simulink model "ASM_Traffic_V2X_Complete_Model_2"  (R2019a)
settings: Solver=ode1  StartTime=SIM.tstart.v  StopTime=Inf  FixedStep=SIM.StepSize.v  RelTol=1e-3
PostLoadFcn:
  | if any(exist('dsrtsu_mdlpostloadfcn', 'file') ~= 0), dsrtsu_mdlpostloadfcn('Execute', bdroot); end
  | try, asm_mdl_postloadfcn(bdroot, 'UpdateModel', 2200); catch, disp(lasterr); end,
undefined symbols (not defined in the file): _SensorPnts_1, _SensorPnts_13, _SensorPnts_17, _SensorPnts_21, _SensorPnts_25, _SensorPnts_29, _SensorPnts_33, _SensorPnts_37, _SensorPnts_41, _SensorPnts_45, _SensorPnts_49, _SensorPnts_5, _SensorPnts_53, _SensorPnts_57, _SensorPnts_9, _to_, CPT, G5A, ITS, MDL, rad, s_to_rpm, SIM
libraries: simulink x169, ASM_VehicleDynamics_lib x126, ASM_Traffic_lib x83, ASM_Utils_lib x49, mdbs x45, ASM_Environment_lib x17, dspindex x12, dsaV2xLibraryAux x10, dsmpblib x6, dsaV2xAsn1Library x4, dsaV2xLibrary x4, ASM_BrakeHydraulics_lib x4
(part 7 of 36)

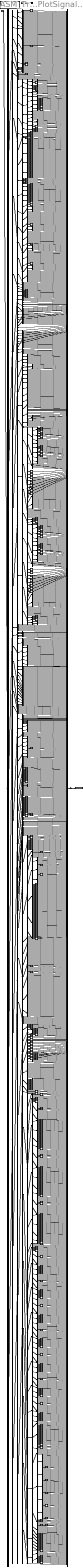
== system ASM_Traffic_V2X_Complete_Model_2/MDLUserInterface/ModelDesk_Plotting/ModelDesk_PlotSignalCollector ==
  ASMSignalBus : Inport
  Accelerations : BusSelector  OutputSignals=VehicleCoG,Wheels
  ActiveBrakeCylinder : BusSelector  OutputSignals=p[bar],p_max[bar],Enable_p_Brake_Desired[0|1],p_Brake_Desired[bar]
  ActiveLateralController : BusSelector  OutputSignals=s_Preview_LatCtrl[m],Angle_SteeringWheel_LatCtrl[deg],e_Lat[m]
  ActiveTire : BusSelector  OutputSignals=v_Circumf_Dyn_FL_Wheel[km|h],Slip_x_FL[],Slip_y_FL[],r_Dyn_FL_Tire[m],CorneringStiffness_FL[N],Coef_RollingRes_FL[],Trq_x_FL_CoorSys_CP[Nm],Trq_y_FL_CoorSys_W[Nm],Trq_z_FL_CoorSys_CP[Nm],F_x_Dyn_FL_Tire_CoorSys_CP[N],F_y_Dyn_FL_Tire_CoorSys_CP[N],F_z_Dyn_FL_Tire_CoorSys_CP[N]
  ActiveTire1 : BusSelector  OutputSignals=v_Circumf_Dyn_FR_Wheel[km|h],Slip_x_FR[],Slip_y_FR[],r_Dyn_FR_Tire[m],CorneringStiffness_FR[N],Coef_RollingRes_FR[],Trq_x_FR_CoorSys_CP[Nm],Trq_y_FR_CoorSys_W[Nm],Trq_z_FR_CoorSys_CP[Nm],F_x_Dyn_FR_Tire_CoorSys_CP[N],F_y_Dyn_FR_Tire_CoorSys_CP[N],F_z_Dyn_FR_Tire_CoorSys_CP[N]
  ActiveTire2 : BusSelector  OutputSignals=v_Circumf_Dyn_RL_Wheel[km|h],Slip_x_RL[],Slip_y_RL[],r_Dyn_RL_Tire[m],CorneringStiffness_RL[N],Coef_RollingRes_RL[],Trq_x_RL_CoorSys_CP[Nm],Trq_y_RL_CoorSys_W[Nm],Trq_z_RL_CoorSys_CP[Nm],F_x_Dyn_RL_Tire_CoorSys_CP[N],F_y_Dyn_RL_Tire_CoorSys_CP[N],F_z_Dyn_RL_Tire_CoorSys_CP[N]
  ActiveTire3 : BusSelector  OutputSignals=v_Circumf_Dyn_RR_Wheel[km|h],Slip_x_RR[],Slip_y_RR[],r_Dyn_RR_Tire[m],CorneringStiffness_RR[N],Coef_RollingRes_RR[],Trq_x_RR_CoorSys_CP[Nm],Trq_y_RR_CoorSys_W[Nm],Trq_z_RR_CoorSys_CP[Nm],F_x_Dyn_RR_Tire_CoorSys_CP[N],F_y_Dyn_RR_Tire_CoorSys_CP[N],F_z_Dyn_RR_Tire_CoorSys_CP[N]
  ActiveTransmission : BusSelector  OutputSignals=Gear[],omega_In_Trm[rad|s],omega_Out_Trm[rad|s],Trq_Out_Trm[Nm],i_Trm[],Inertia_Trm[kgm2],i_unsync_Trm[]
  Aerodynamics : BusSelector  OutputSignals=Forces,Torques,Coefficients
  Ambient : BusSelector  OutputSignals=T_Ambient[degC],p_Ambient[Pa]
  Angle_FL_Wheel[Alpha;Beta;Gamma][deg] : BusSelector  OutputSignals=Angle_Alpha_FL_Wheel[deg],Angle_Beta_FL_Wheel[deg],Angle_Gamma_FL_Wheel[deg]
  Angle_FL_Wheel[Toe;Camber][deg] : BusSelector  OutputSignals=Angle_Toe_FL_Wheel_CoorSys_V[deg],Angle_Camber_FL_Wheel_CoorSys_V[deg]
  Angle_FR_Wheel[Alpha;Beta;Gamma][deg] : BusSelector  OutputSignals=Angle_Alpha_FR_Wheel[deg],Angle_Beta_FR_Wheel[deg],Angle_Gamma_FR_Wheel[deg]
  Angle_FR_Wheel[Toe;Camber][deg] : BusSelector  OutputSignals=Angle_Toe_FR_Wheel_CoorSys_V[deg],Angle_Camber_FR_Wheel_CoorSys_V[deg]
  Angle_Fellows[x;y;z][deg] : BusSelector  OutputSignals=Angle_Roll_Fellows[deg],Angle_Pitch_Fellows[deg],Angle_Yaw_Fellows[deg],Angle_Wheel_Fellows[deg]
  Angle_RL_Wheel[Alpha;Beta;Gamma][deg] : BusSelector  OutputSignals=Angle_Alpha_RL_Wheel[deg],Angle_Beta_RL_Wheel[deg],Angle_Gamma_RL_Wheel[deg]
  Angle_RL_Wheel[Toe;Camber][deg] : BusSelector  OutputSignals=Angle_Toe_RL_Wheel_CoorSys_V[deg],Angle_Camber_RL_Wheel_CoorSys_V[deg]
  Angle_RR_Wheel[Alpha;Beta;Gamma][deg] : BusSelector  OutputSignals=Angle_Alpha_RR_Wheel[deg],Angle_Beta_RR_Wheel[deg],Angle_Gamma_RR_Wheel[deg]
  Angle_RR_Wheel[Toe;Camber][deg] : BusSelector  OutputSignals=Angle_Toe_RR_Wheel_CoorSys_V[deg],Angle_Camber_RR_Wheel_CoorSys_V[deg]
  Angle_Vehicle_CoorSys_E[x;y;z][deg] : BusSelector  OutputSignals=Angle_Roll_Vehicle_CoorSys_E[deg],Angle_Pitch_Vehicle_CoorSys_E[deg],Angle_Yaw_Vehicle_CoorSys_E[deg]
  Angle_Vehicle_Init_CoorSys_E[x;y;z][rad] : BusSelector  OutputSignals=Angle_Roll_Vehicle_Init[rad],Angle_Pitch_Vehicle_Init[rad],Angle_Yaw_Vehicle_Init[rad]
  Angle_Wheel[FL;FR][Toe;Camber][deg] : BusSelector  OutputSignals=Angle_FL_Wheel[Toe;Camber][deg],Angle_FR_Wheel[Toe;Camber][deg]
  Angle_Wheel[RL;RR][Toe;Camber][deg] : BusSelector  OutputSignals=Angle_RL_Wheel[Toe;Camber][deg],Angle_RR_Wheel[Toe;Camber][deg]
  Angular : BusSelector  OutputSignals=w_Vehicle_CoG_dt[x;y;z][rad|s2]
  Angular1 : BusSelector  OutputSignals=w_Vehicle_CoG[x;y;z][deg|s]
  Angular2 : BusSelector  OutputSignals=WheelBodyAngularVelocity,WheelAngularVelocity
  Angular3 : BusSelector  OutputSignals=Angle_Vehicle_CoorSys_E[x;y;z][deg],RotationMatrix_V_to_E[3x3]
  AutomaticTransmission : BusSelector  OutputSignals=LockUpClutch,GearBox,TorqueConverter
  AutomaticTrmCtrlSignals : BusSelector  OutputSignals=SelectorLever[-3T|-2P|-1R|0N|1D],SW_TipTronic[-1Down|0Off|1Up]
  BasicEngine : BusSelector  OutputSignals=EngineTorques,FuelConsumption
  BellValve : BusSelector  OutputSignals=ValveState[1ChamberCon|2AmbientCon|3CloseAll],p_In_BellValve[bar],p_Out_BellValve[bar],T_In_BellValve[degC],m_dot_BellValve[Kg|s],Ctrl_BellValve[0_1]
  Brake : BusSelector  OutputSignals=MasterBrakeCylinder,BrakeHydraulics,BrakeDisc,BrakeBooster,Manifold
  BrakeBooster : BusSelector  OutputSignals=ManifoldValve,VacuumChamber,BellValve,RearChamber,PushRod,ControllerBellValve
  BrakeCylinderLinear : BusSelector  OutputSignals=p[bar],p_max[bar]
  BrakeCylinderPhysical : BusSelector  OutputSignals=Displ_Piston[mm],F[N],p[bar],p_max[bar]
  BrakeDisc : BusSelector  OutputSignals=Torque,MaximumTorque,Pressure,Const_BrakeDiscFactor
  BrakeHydraulics : BusSelector  OutputSignals=BrakingCircuit,BrakeHydraulicsModel[]
  BrakingCircuit : BusSelector  OutputSignals=Pressure
  BusSelector_1 : BusSelector  OutputSignals=SoftECU,VehicleDynamics,BasicEngine,Drivetrain,Environment
  CO2_Emission : BusSelector  OutputSignals=CO2_Emission[kg|h],CO2_Emission_Total[kg]
  CentralDifferential : BusSelector  OutputSignals=omega_Out_Front_CentralDiff[rad|s],omega_Out_Rear_CentralDiff[rad|s],omega_In_CentralDiff[rad|s],Trq_Lock[Nm],omega_Cage[rad|s],Const_i_MainReductionGear[],Const_TrqDistribution[]
  Clutch : BusSelector  OutputSignals=Trq_Fric_Clutch[Nm],Trq_TorsionSpring_Clutch[Nm],omega_Out_ClutchPlate[rad|s]
  Clutch_4WD : BusSelector  OutputSignals=Trq_Lock_Clutch_4WD[Nm],omega_Clutch_4WD_In[rad|s],omega_Clutch_4WD_Out[rad|s]
  Coefficients : BusSelector  OutputSignals=Cw_x[]
  Collision_Sensor : BusSelector  OutputSignals=Collision_Sensor_1
  Collision_Sensor_1 : BusSelector  OutputSignals=Info,SensorOutput
  Common : BusSelector  OutputSignals=LaneID_PrefLane[],LaneID_Absolute[],LaneDirection_Absolute[],LaneDirection_Relative[],LaneWidth[m],LaneCurvature[1|m],Curvature[1|m]
  ComplianceAligningTorque : BusSelector  OutputSignals=Displ_x_Wheel_Trq_z_Left[mm],Displ_x_Wheel_Trq_z_Right[mm],Displ_y_Wheel_Trq_z_Left[mm],Displ_y_Wheel_Trq_z_Right[mm],Angle_Alpha_Wheel_Trq_z_Left[deg],Angle_Alpha_Wheel_Trq_z_Right[deg],Angle_Gamma_Wheel_Trq_z_Left[deg],Angle_Gamma_Wheel_Trq_z_Right[deg]
  ComplianceAligningTorque1 : BusSelector  OutputSignals=Displ_x_Wheel_Trq_z_Left[mm],Displ_x_Wheel_Trq_z_Right[mm],Displ_y_Wheel_Trq_z_Left[mm],Displ_y_Wheel_Trq_z_Right[mm],Angle_Alpha_Wheel_Trq_z_Left[deg],Angle_Alpha_Wheel_Trq_z_Right[deg],Angle_Gamma_Wheel_Trq_z_Left[deg],Angle_Gamma_Wheel_Trq_z_Right[deg]
  ComplianceLatForce : BusSelector  OutputSignals=Displ_x_Wheel_F_y_Left[mm],Displ_x_Wheel_F_y_Right[mm],Displ_y_Wheel_F_y_Left[mm],Displ_y_Wheel_F_y_Right[mm],Angle_Alpha_Wheel_F_y_Left[deg],Angle_Alpha_Wheel_F_y_Right[deg],Angle_Gamma_Wheel_F_y_Left[deg],Angle_Gamma_Wheel_F_y_Right[deg]
  ComplianceLatForce1 : BusSelector  OutputSignals=Displ_x_Wheel_F_y_Left[mm],Displ_x_Wheel_F_y_Right[mm],Displ_y_Wheel_F_y_Left[mm],Displ_y_Wheel_F_y_Right[mm],Angle_Alpha_Wheel_F_y_Left[deg],Angle_Alpha_Wheel_F_y_Right[deg],Angle_Gamma_Wheel_F_y_Left[deg],Angle_Gamma_Wheel_F_y_Right[deg]
  ComplianceLongForce : BusSelector  OutputSignals=Displ_x_Wheel_F_x_Left[mm],Displ_x_Wheel_F_x_Right[mm],Displ_y_Wheel_F_x_Left[mm],Displ_y_Wheel_F_x_Right[mm],Angle_Alpha_Wheel_F_x_Left[deg],Angle_Alpha_Wheel_F_x_Right[deg],Angle_Gamma_Wheel_F_x_Left[deg],Angle_Gamma_Wheel_F_x_Right[deg]
  ComplianceLongForce1 : BusSelector  OutputSignals=Displ_x_Wheel_F_x_Left[mm],Displ_x_Wheel_F_x_Right[mm],Displ_y_Wheel_F_x_Left[mm],Displ_y_Wheel_F_x_Right[mm],Angle_Alpha_Wheel_F_x_Left[deg],Angle_Alpha_Wheel_F_x_Right[deg],Angle_Gamma_Wheel_F_x_Left[deg],Angle_Gamma_Wheel_F_x_Right[deg]
  ComplianceLongTorque : BusSelector  OutputSignals=Displ_x_Wheel_Trq_x_Left[mm],Displ_x_Wheel_Trq_x_Right[mm],Displ_y_Wheel_Trq_x_Left[mm],Displ_y_Wheel_Trq_x_Right[mm],Angle_Alpha_Wheel_Trq_x_Left[deg],Angle_Alpha_Wheel_Trq_x_Right[deg],Angle_Gamma_Wheel_Trq_x_Left[deg],Angle_Gamma_Wheel_Trq_x_Right[deg]
  ComplianceLongTorque1 : BusSelector  OutputSignals=Displ_x_Wheel_Trq_x_Left[mm],Displ_x_Wheel_Trq_x_Right[mm],Displ_y_Wheel_Trq_x_Left[mm],Displ_y_Wheel_Trq_x_Right[mm],Angle_Alpha_Wheel_Trq_x_Left[deg],Angle_Alpha_Wheel_Trq_x_Right[deg],Angle_Gamma_Wheel_Trq_x_Left[deg],Angle_Gamma_Wheel_Trq_x_Right[deg]
  Const_BrakeDiscFactor : BusSelector  OutputSignals=Const_BrakeDiscFactor_FL[m3],Const_BrakeDiscFactor_FR[m3],Const_BrakeDiscFactor_RL[m3],Const_BrakeDiscFactor_RR[m3]
  ContactPoint : BusSelector  OutputSignals=r_FL_Tire[m],Pos_CP_FL_CoorSys_E[x;y][m]
  ContactPoint1 : BusSelector  OutputSignals=r_FR_Tire[m],Pos_CP_FR_CoorSys_E[x;y][m]
  ContactPoint2 : BusSelector  OutputSignals=r_RL_Tire[m],Pos_CP_RL_CoorSys_E[x;y][m]
  ContactPoint3 : BusSelector  OutputSignals=r_RR_Tire[m],Pos_CP_RR_CoorSys_E[x;y][m]
  ContentID : Constant  Value=81472368640
  ControllerBellValve : BusSelector  OutputSignals=p_Setpoint[bar],p_MasterBrakeCyl[bar],p_delta[bar],ValveState[1ChamberCon|2AmbientCon],Ctrl_A_BellValve[0_1],F_Pedal[N]
  Controller_ACC : BusSelector  OutputSignals=State_ACC[0Off|1On],Sw_ACC_Distance[s],Control_Mode_ACC[0Off|1CC|2DC],v_Set_CC[km|h],v_Set_DC[km|h],v_Set[km|h],a_x_Set[m|s2],a_x_UpperLimit[m|s2],a_x_LowerLimit[m|s2],a_x_RisingRateMax[m|s3],a_x_FallingRateMax[m|s3]s,Distance_Set[m],Dist_Ref_Vehicle[m],FCW[0Off|1On],AEB[0Off|1On],TTC[s],Collision[0Off|1On],Sw_BrakeMode[1Comfort|2AEBOnly|3AEBOff],Enable_Trq_Brake_ACC[0|1],Enable_Trq_Engine_ACC[0|1]
  Crankshaft : BusSelector  OutputSignals=n_Engine[rad|s],n_Engine[rpm],Trq_Mass_Mod[Nm],Const_Inertia_Engine[kgm2],Trq_Eff_Crank[Nm]
  CurrentLane : BusSelector  OutputSignals=Common,LeftSide,RightSide
  CustomPoints : BusSelector  OutputSignals=ID[],Object_ID[],Dist_CoorSys_S[m],Angle_Hor_CoorSys_S[deg],Pos_CoorSys_E[x;y;z][m]
  CustomPoints1 : BusSelector  OutputSignals=ID[],Object_ID[],Dist_CoorSys_S[m],Angle_Hor_CoorSys_S[deg],Pos_CoorSys_E[x;y;z][m]
  CustomPoints2 : BusSelector  OutputSignals=ID[],Object_ID[],Dist_CoorSys_S[m],Angle_Hor_CoorSys_S[deg],Pos_CoorSys_E[x;y;z][m]
  Custom_Sensor : BusSelector  OutputSignals=Sensor_Front_1
  Damper_Left : BusSelector  OutputSignals=Displ_Damper_FL_dt[m|s],Displ_Damper_FL_dq1_Front[],Displ_Damper_FL_dq2_Front[],Displ_Damper_FL[m]
  Damper_Left1 : BusSelector  OutputSignals=Displ_Damper_RL_dt[m|s],Displ_Damper_RL_dq1_Rear,Displ_Damper_RL_dq2_Rear,Displ_Damper_RL[m]
  Damper_Right : BusSelector  OutputSignals=Displ_Damper_FR_dt[m|s],Displ_Damper_FR_dq1_Front[],Displ_Damper_FR_dq2_Front[],Displ_Damper_FR[m]
  Damper_Right1 : BusSelector  OutputSignals=Displ_Damper_RR_dt[m|s],Displ_Damper_RR_dq1_Rear[],Displ_Damper_RR_dq2_Rear[],Displ_Damper_RR[m]
  DataTypeConversion_{1,37,66,856,1103,1105..1106,1258,1545} (9 alike) : DataTypeConversion  OutDataTypeStr=double  SaturateOnIntegerOverflow=on  RndMeth=Zero
  DesiredBrakePressure : BusSelector  OutputSignals=Enable_p_Brake_Desired[0|1],p_Brake_Desired[bar]
  DiscreteObjects : BusSelector  OutputSignals=DiscreteObjectsState[],Data_Valid[]
  Dist_Response_Maneuver : BusSelector  OutputSignals=Distance_xy[m],Distance_z[m]
  Dist_Response_Traffic : BusSelector  OutputSignals=Distance_xy[m],Distance_z[m]
  Driver : BusSelector  OutputSignals=OutputSignals,LongitudinalController,ReferenceVelocity,LateralController
  Drivetrain : BusSelector  OutputSignals=Transmission,FinalDriveAssembly,Crankshaft,Starter,TestBench
  Efficiency : BusSelector  OutputSignals=eta_Eff_Engine[0_1],eta_Ind_Engine[0_1],eta_Mechanical_Engine[0_1]
  EngineOperation : BusSelector  OutputSignals=Sw_Starter[0Off|1On],State_Engine[0|1|2|3|4]
  EngineTorques : BusSelector  OutputSignals=Const_TimeConst[s],Trq_Eff_Engine[Nm],Trq_Driver_Des[Nm],Trq_Fric_Engine[Nm],Trq_Ind_Engine[Nm],Trq_FullLoad_Engine[Nm]
  Environment : BusSelector  OutputSignals=Driver,Road,Maneuver,Traffic
  F_FL_Tire_CoorSys_V[x;y;z][N] : BusSelector  OutputSignals=F_x_FL_Tire_CoorSys_V[N],F_y_FL_Tire_CoorSys_V[N],F_z_FL_Tire_CoorSys_V[N]
  F_FR_Tire_CoorSys_V[x;y;z][N] : BusSelector  OutputSignals=F_x_FR_Tire_CoorSys_V[N],F_y_FR_Tire_CoorSys_V[N],F_z_FR_Tire_CoorSys_V[N]
  F_RL_Tire_CoorSys_V[x;y;z][N] : BusSelector  OutputSignals=F_x_RL_Tire_CoorSys_V[N],F_y_RL_Tire_CoorSys_V[N],F_z_RL_Tire_CoorSys_V[N]
  F_RR_Tire_CoorSys_V[x;y;z][N] : BusSelector  OutputSignals=F_x_RR_Tire_CoorSys_V[N],F_y_RR_Tire_CoorSys_V[N],F_z_RR_Tire_CoorSys_V[N]
  FellowMovement : BusSelector  OutputSignals=FellowMovement,FellowPositions,FellowVelocities,TrafficScheduler,UserSignals_Customized
  FellowMovement1 : BusSelector  OutputSignals=d_Total_Fellows[m],LaneIdx_Total_Fellows[],s_Fellows[m],v_Fellows[km|h]
  FellowPositions : BusSelector  OutputSignals=Pos_Fellows_MainPnt_CoorSys_E[x;y;z][m],Angle_Fellows[x;y;z][deg],Angle_Wheel_Fellows[deg]
  FellowVelocities : BusSelector  OutputSignals=v_Fellows[x;y;z][km|h],w_Fellows[x;y;z][deg|s]
  FellowsGeometry : BusSelector  OutputSignals=Info,Data_Valid_Fellows[0|1],PosVec_MainPnt_Fellows[x;y;z][m],Length_Fellows[m],Width_Fellows[m],Height_Fellows[m],Wheel_Radius_Fellows[m],TrackWidth_Front_Fellows[m],TrackWidth_Rear_Fellows[m],WheelBase_Fellows[m],TrafficObject_Type_Fellows[]
  FinalDriveAssembly : BusSelector  OutputSignals=i_FinalDrive[],CentralDifferential,FrontDifferential,RearDifferential,Shaft_TGCL4WD,Shaft_CF,Shaft_CR,TransferGearbox,Clutch_4WD,Shaft_FL,Shaft_FR,Shaft_RL,Shaft_RR
  Forces : BusSelector  OutputSignals=F_x_Aero_CoorSys_V[N],F_y_Aero_CoorSys_V[N],F_z_Aero_CoorSys_V[N]
  ForcesAndTorques : BusSelector  OutputSignals=g_F_Steering_SteeringRod[N],Trq_Steering[Nm],Trq_PowerSteering[Nm],TrqSpring_SteeringColumn[Nm],Trq_PowerSteeringDynamics[Nm],TrqSpring_PowerSteeringSystem[Nm]
  FrontDifferential : BusSelector  OutputSignals=omega_Out_Lef_FrontDifferentialt[rad|s],omega_Out_Right_FrontDifferential[rad|s],omega_In_CentralDiff_FrontDifferential[rad|s],Trq_Lock_FrontDifferential[Nm],omega_Cage[rad|s],Const_i_MainReductionGear[],Const_TrqDistribution[]
  FuelConsumption : BusSelector  OutputSignals=mdot_Fuel[g|h],b_e[g|kWh],Efficiency,CO2_Emission,Fuel_Consumption[l|h],Fuel_Consumption_Total[l]
  GearBox : BusSelector  OutputSignals=i_unsync_Trm[],i_Trm[],Trq_Out_Trm[Nm],omega_In_Trm[rad|s],Inertia_Trm[kgm2],omega_Out_Trm[rad|s]
  GearBox1 : BusSelector  OutputSignals=i_unsync_Trm[],i_Trm[],Trq_Out_Trm[Nm],omega_In_Trm[rad|s],Inertia_Trm[kgm2],omega_Out_Trm[rad|s]
  GearShifter : BusSelector  OutputSignals=Pos_AccPedal[%],Pos_BrakePedal[%],Pos_ClutchPedal[%],Gear[],SelectorLever[-3T|-2P|-1R|0N|1D]
  Generalized : BusSelector  OutputSignals=v_Vehicle[x;y;z][km|h],w_Vehicle[x;y;z][deg|s],z_Wheel_dt[FL;FR;RL;RR][m|s]
  GeneralizedForcesAndTorques : BusSelector  OutputSignals=g_F_Vehicle[x;y;z][N],g_Trq_Vehicle[x;y;z][N],g_F_z_Wheel[FL;FR;RL;RR][N]
  GeneralizedForcesAndTorques1 : BusSelector  OutputSignals=g_FTrq_Tire_Steering[N],g_Trq_FL_Steering[N],g_Trq_FR_Steering[N],g_F_FL_Steering[N],g_F_FR_Steering[N]
  GeneralizedVelocitiesDerivative : BusSelector  OutputSignals=v_Vehicle_dt[x;y;z][m|s2],w_Vehicle_dt[x;y;z][rad|s2],q_Wheel_dt2[q1_Front;q2_Front;q1_Rear;q2_Rear][]
  GravitationalForces : BusSelector  OutputSignals=F_Vehicle_Gravitational[x;y;z][N],F_FL_Gravitational[x;y;z][N],F_FR_Gravitational[x;y;z][N],F_RL_Gravitational[x;y;z][N],F_RR_Gravitationa[x;y;z]l[N]
  GravityAcceleration : BusSelector  OutputSignals=a_Gravity_CoorSys_V[x;y;z][m|s2]
  GyroscopicForces : BusSelector  OutputSignals=F_Vehicle_Gyroscopic[x;y;z][N],F_FL_Gyroscopic[x;y;z][N],F_FR_Gyroscopic[x;y;z][N],F_RL_Gyroscopic[x;y;z][N],F_RR_Gyroscopic[x;y;z][N]
  GyroscopicTorques : BusSelector  OutputSignals=Trq_Vehicle_Gyroscope[x;y;z][Nm],Trq_FL_Gyroscope[x;y;z][Nm],Trq_FR_Gyroscope[x;y;z][Nm],Trq_RL_Gyroscope[x;y;z][Nm],Trq_RR_Gyroscope[x;y;z][Nm]
  IdleSpeedControl : BusSelector  OutputSignals=Const_n_Engine_Idle_Set[rpm],Pos_AccPedal[%]
  Info : BusSelector  OutputSignals=CurrentSegment[],t_local[s],s_local[m],ManeuverTime[s],ManeuverState[],ErrorFlag[],CurrentSequence[]
  Info1 : BusSelector  OutputSignals=TrafficState[],ErrorFlag[],CurrentSequence_Fellows[],CurrentSegment_Fellows[],t_local_Fellows[s],CurrentSequence_UserSignals[],CurrentSegment_UserSignals[],t_local_UserSignals[s],CurrentSegment[],t_local[s]
  Info{6..12} (7 alike) : BusSelector  OutputSignals=ObjectSensor2D_Sfcn_State[],ObjectSensor2D_Data_Valid[0|1]
  Info13 : BusSelector  OutputSignals=TrafficSignSensor_Dyn_Sfcn_State[],TrafficSignSensor_Dyn_Data_Valid[0|1]
  Info14 : BusSelector  OutputSignals=CustomSensor_ScopezoneSfcn_State[],CustomSensor_OutputSfcn_State[],CustomSensor_Data_Valid[0|1]
  Info15 : BusSelector  OutputSignals=LineSensor_Data_Outport[],LineSensor_Data_Outport_Version[],LineSensor_Data_Valid[0|1|2],Num_Pnts_Detected_Road_Lanes[],Num_Pnts_Detected_Road_Shape_Lines[],Num_Pnts_Detected_Road_Shape_ContObj[],Num_Pnts_Detected_Junction_Borders[],Num_Pnts_Detected_Junction_Shape_Lines[],Num_Pnts_Detected_Junction_Shape_ContObj[]
  Info16 : BusSelector  OutputSignals=Sfunc_State[],Data_Valid[0|1]
  Info2 : BusSelector  OutputSignals=FellowParameters_Sfcn_State[],FellowParameters_Data_Valid[0|1]
  Info3 : BusSelector  OutputSignals=Flag_Object_In_Scope[0Out|1In],Flag_Sensor_Apex_In_Object[0Out|1In]
  Info4 : BusSelector  OutputSignals=Flag_Object_In_Scope[0Out|1In],Flag_Sensor_Apex_In_Object[0Out|1In]
  Info5 : BusSelector  OutputSignals=Flag_Object_In_Scope[0Out|1In],Flag_Sensor_Apex_In_Object[0Out|1In]
  InfoBlock : Subsystem
      settings: OpenFcn=|
      | parent_blk=get_param(gcb,'Parent');
      | asm_mdld_plot_update_gui(parent_blk);
      mask Display: fprintf('Structural changes of the signal bus require an update \nof the ''ModelDesk_PlotSignalCollector'' block. \n\nTo start the update process double click this information block.\n\n WARNING:\n During update this subsystem will be cleared completely')
  InitialVehStates : BusSelector  OutputSignals=s_Vehicle_Init[m],d_Vehicle_Init[m],LaneIdx_Vehicle_Init[],Pos_z_Vehicle_Rel_Init[m],Angle_Yaw_Vehicle_Rel_Init[deg],v_Vehicle_Init[km|h],Route_Id_Init[],Route_Direction_Init[]
  Interface_ACC : BusSelector  OutputSignals=Trq_Request_Brake_ACC[Nm],Trq_Request_Engine_ACC[Nm]
  Kinematics_Left : BusSelector  OutputSignals=Position_Left,Orientation_Left,Spring_Left,Damper_Left
  Kinematics_Left1 : BusSelector  OutputSignals=Position_Left,Orientation_Left,Spring_Left,Damper_Left
  Kinematics_Right : BusSelector  OutputSignals=Position_Right,Orientation_Right,Spring_Right,Damper_Right
  Kinematics_Right1 : BusSelector  OutputSignals=Position_Right,Orientation_Right,Spring_Right,Damper_Right
  LaneSensor_Dynamic : BusSelector  OutputSignals=Parameters,Sensor_Output
  Lanes_Left : BusSelector  OutputSignals=LaneID_PrefLane[],LaneID_Absolute[],LaneDirection_Absolute[],LaneDirection_Relative[],LaneWidth[m],LaneCurvature[1|m],Pos_Left[x;y;z][m],Yaw_Angle_Left[deg],Yaw_Angle_RelVehicle_Left[deg],Curvature_Left[1|m],MarkerType_Left[],MarkerWidth_Left[m],MarkerColor_Left[],LineID_1_Left[],LineID_2_Left[],Distance_Marker_Left[m],Pos_Right[x;y;z][m],Yaw_Angle_Right[deg],Yaw_Angle_RelVehicle_Right[deg],Curvature_Right[1|m],MarkerType_Right[],MarkerWidth_Right[m],MarkerColor_Right[],LineID_1_Right[],LineID_2_Right[],Distance_Marker_Right[m]
  Lanes_Right : BusSelector  OutputSignals=LaneID_PrefLane[],LaneID_Absolute[],LaneDirection_Absolute[],LaneDirection_Relative[],LaneWidth[m],LaneCurvature[1|m],Pos_Left[x;y;z][m],Yaw_Angle_Left[deg],Yaw_Angle_RelVehicle_Left[deg],Curvature_Left[1|m],MarkerType_Left[],MarkerWidth_Left[m],MarkerColor_Left[],LineID_1_Left[],LineID_2_Left[],Distance_Marker_Left[m],Pos_Right[x;y;z][m],Yaw_Angle_Right[deg],Yaw_Angle_RelVehicle_Right[deg],Curvature_Right[1|m],MarkerType_Right[],MarkerWidth_Right[m],MarkerColor_Right[],LineID_1_Right[],LineID_2_Right[],Distance_Marker_Right[m]
  LatCtrl1 : BusSelector  OutputSignals=s_Preview_Lat[m],Angle_Steering[rad],Angle_SteeringWheel[deg]
  LatCtrl2 : BusSelector  OutputSignals=Angle_SteeringWheel[deg],Angle_Steering[deg],s_Preview_Lat[m],e_Yaw[deg],e_Lat[m],e_Lat_Preview[m]
  LateralController : BusSelector  OutputSignals=ActiveLateralController,signal2.LatCtrl1,LatCtrl2,PositionError
  LeftSide : BusSelector  OutputSignals=Pos_Left[x;y;z][m],Yaw_Angle_Left[deg],Yaw_Angle_RelVehicle_Left[deg],Curvature_Left[1|m],MarkerType_Left[],MarkerWidth_Left[m],MarkerColor_Left[],LineID_1_Left[],LineID_2_Left[],Distance_Marker_Left[m]
  Line_Sensor : BusSelector  OutputSignals=Line_Sensor_1
  Line_Sensor_1 : BusSelector  OutputSignals=Info,Pos_Road_Lane_Animation_CoorSys_E,Pos_Road_Shape_Line_Animation_CoorSys_E,Pos_Road_Shape_ContObj_Animation_CoorSys_E,Pos_Junction_Border_Animation_CoorSys_E,Pos_Junction_Shape_Line_Animation_CoorSys_E,Pos_Junction_Shape_ContObj_Animation_CoorSys_E,Dummy_SensorOutput
  Linear : BusSelector  OutputSignals=a_Vehicle_CoG[x;y;z][m|s2],a_Vehicle_Cog_withG[x;y;z][m|s2]
  Linear1 : BusSelector  OutputSignals=a_FL_Wheel[x;y;z][m|s2],a_FR_Wheel[x;y;z][m|s2],a_RL_Wheel[x;y;z][m|s2],a_RR_Wheel[x;y;z][m|s2]
  Linear2 : BusSelector  OutputSignals=v_Vehicle_CoG[x;y;z][km|h],v_Total_Vehicle[km|h],Angle_SideSlip_Vehicle[deg]
  Linear3 : BusSelector  OutputSignals=WheelBodyVelocity
  Linear4 : BusSelector  OutputSignals=Pos_Vehicle_CoorSys_E[x;y;z][m],s_Vehicle[m]
  Linear5 : BusSelector  OutputSignals=Pos_FL_Wheels_CoorSys_E[x;y;z][m],Pos_FR_Wheels_CoorSys_E[x;y;z][m],Pos_RL_Wheels_CoorSys_E[x;y;z][m],Pos_RR_Wheels_CoorSys_E[x;y;z][m]
  LockUpClutch : BusSelector  OutputSignals=Trq_Fric_Clutch[Nm],Trq_TorsionSpring_Clutch[Nm],omega_Out_ClutchPlate[rad|s]
  Lockup_Clutch_Control : BusSelector  OutputSignals=Ctrl_Lockup_Clutch[%]
  LongCtrl : BusSelector  OutputSignals=t_Preview[s],Pos_AccPedal[%],Pos_BrakePedal[%]
  LongitudinalController : BusSelector  OutputSignals=LongCtrl,GearShifter
  MDLD_DATA_CAPTURE : MDLD_Utils_lib/ModelDeskPlotInterface/DataCapture_Sfcn/MDLD_DATA_CAPTURE  inputPortWidth=15518  measurementSignals=[0 0 0 0 0 0 0 0 0 0 0 0 0 0 0 0 0 0 0 0 0 0 0 0 0 0 0 0 0 0 0 0 0 0 0 0 0 0 0 0 0 0 0 0 0 0 0 0 0 0 0 0 0 0 0 0 0 0 0 0 0 0 0 0 0 0 0 0 0 0 0 0 0 0 0 0 0 0 0 0 0 0 0 0 0 0 0 0 0 0 0 0 0 0 0 0 0 0 0 0 0 0 0 0 0 0 0 0 0 0 0 0 0 0 0 0 0 0 0 0 0 0 0 0 0 0 0 0 0 0 0 0 0 0 0 0 0 0 0 0 0 0 0 0 0 0 0 0 0 0 0 0 0 0 0 0 0 0 0 0 0 0 0 0 0 0 0 0 0 0 0 0 0 0 0 0 0 0 0 0 0 0 0 0 0 0 0 0 0 0 0 0 0 0 0 0 0 0 0 0 0 0 0 0 0 0 0 0 0 0 0 0 0 0 0 0 0 0 0 0 0 0 0 0 0 0 0 0 0 0 0 0 0 0 0 0 0 0 0 0 0 0 0 0 0 0 0 0 0 0 0 0 0 0 0 0 0 0 0 0 0 0 0 0 0 0 0 0 0 0 0 0 0 0 0 0 0 0 0 0 0 0 0 0 0 0 0 0 0 0 0 0 0 0 0 0 0 0 0 0 0 0 0 0 0 0 0 0 0 0 0 0 0 0 0 0 0 0 0 0 0 0 0 0 0 0 0 0 0 0 0 0 0 0 0 0 0 0 0 0 0 0 0 0 0 0 0 0 0 0 0 0 0 0 0 0 0 0 0 0 0 0 0 0 0 0 0 0 0 0 0 0 0 0 0 0 0 0 0 0 0 0 0 0 0 0 0 0 0 0 0 0 0 0 0 0 0 0 0 0 0 0 0 0 0 0 0 0 0 0 0 0 0 0 0 0 0 0 0 0 0 0 0 0 0 0 0 0 0 0 0 0 0 0 0 0 0 0 0 0 0 0 0 0 0 0 0 0 0 0 0 0 0 0 0 0 0 0 0 0 0 0 0 0 0 0 0 0 0 0 0 0 0 0 0 0 0 0 0 0 0 0 0 0 0 0 0 0 0 0 0 0 0 0 0 0 0 0 0 0 0 0 0 0 0 0 0 0 0 0 0 0 0 0 0 0 0 0 0 0 0 0 0 0 0 0 0 0 0 0 0 0 0 0 0 0 0 0 0 0 0 0 0 0 0 0 0 0 0 0 0 0 0 0 0 0 0 0 0 0 0 0 0 0 0 0 0 0 0 0 0 0 0 0 0 0 0 0 0 0 0 0 0 0 0 0 0 0 0 0 0 0 0 0 0 0 0 0 0 0 0 0 0 0 0 0 0 0 0 0 0 0 0 0 0 0 0 0 0 0 0 0 0 0 0 0 0 0 0 0 0 0 0 0 0 0 0 0 0 0 0 0 0 0 0 0 0 0 0 0 0 0 0 0 0 0 0 0 0 0 0 0 0 0 0 0 0 0 0 0 0 0 0 0 0 0 0 0 0 0 0 0 0 0 0 0 0 0 0 0 0 0 0 0 0 0 0 0 0 0 0 0 0 0 0 0 0 0 0 0 0 0 0 0 0 0 0 0 0 0 0 0 0 0 0 0 0 0 0 0 0 0 0 0 0 0 0 0 0 0 0 0 0 0 0 0 0 0 0 0 0 0 0 0 0 0 0 0 0 0 0 0 0 0 0 0 0 0 0 0 0 0 0 0 0 0 0 0 0 0 0 0 0 0 0 0 0 0 0 0 0 0 0 0 0 0 0 0 0 0 0 0 0 0 0 0 0 0 0 0 0 0 0 0 0 0 0 0 0 0 0 0 0 0 0 0 0 0 0 0 0 0 0 0 0 0 0 0 0 0 0 0 0 0 0 0 0 0 0 0 0 0 0 0 0 0 0 0 0 0 0 0 0 0 0 0 0 0 0 0 0 0 0 0 0 0 0 0 0 0 0 0 0 0 0 0 0 0 0 0 0 0 0 0 0 0 0 0 0 0 0 0 0 0 0 0 0 0 0 0 0 0 0 0 0 0 0 0 0 0 0 0 0 0 0 0 0 0 0 0 0 0 0 0 0 0 0 0 0 0 0 0 0 0 0 0 0 0 0 0 0 0 0 0 0 0 0 0 0 0 0 0 0 0 0 0 0 0 0 0 0 0 0 0 0 0 0 0 0 0 0 0 0 0 0 0 0 0 0 0 0 0 0 0 0 0 0 0 0 0 0 0 0 0 0 0 0 0 0 0 0 0 0 0 0 0 0 0 0 0 0 0 0 0 0 0 0 0 0 0 0 0 0 0 0 0 0 0 0 0 0 0 0 0 0 0 0 0 0 0 0 0 0 0 0 0 0 0 0 0 0 0 0 0 0 0 0 0 0 0 0 0 0 0 0 0 0 0 0 0 0 0 0 0 0 0 0 0 0 0 0 0 0 0 0 0 0 0 0 0 0 0 0 0 0 0 0 0 0 0 0 0 0 0 0 0 0 0 0 0 0 0 0 0 0 0 0 0 0 0 0 0 0 0 0 0 0 0 0 0 0 0 0 0 0 0 0 0 0 0 0 0 0 0 0 0 0 0 0 0 0 0 0 0 0 0 0 0 0 0 0 0 0 0 0 0 0 0 0 0 0 0 0 0 0 0 0 0 0 0 0 0 0 0 0 0 0 0 0 0 0 0 0 0 0 0 0 0 0 0 0 0 0 0 0 0 0 0 0 0 0 0 0 0 0 0 0 0 0 0 0 0 0 0 0 0 0 0 0 0 0 0 0 0 0 0 0 0 0 0 0 0 0 0 0 0 0 0 0 0 0 0 0 0 0 0 0 0 0 0 0 0 0 0 0 0 0 0 0 0 0 0 0 0 0 0 0 0 0 0 0 0 0 0 0 0 0 0 0 0 0 0 0 0 0 0 0 0 0 0 0 0 0 0 0 0 0 0 0 0 0 0 0 0 0 0 0 0 0 0 0 0 0 0 0 0 0 0 0 0 0 0 0 0 0 0 0 0 0 0 0 0 0 0 0 0 0 0 0 0 0 0 0 0 0 0 0 0 0 0 0 0 0 0 0 0 0 0 0 0 0 0 0 0 0 0 0 0 0 0 0 0 0 0 0 0 0 0 0 0 0 0 0 0 0 0 0 0 0 0 0 0 0 0 0 0 0 0 0 0 0 0 0 0 0 0 0 0 0 0 0 0 0 0 0 0 0 0 0 0 0 0 0 0 0 0 0 0 0 0 0 0 0 0 0 0 0 0 0 0 0 0 0 0 0 0 0 0 0 0 0 0 0 0 0 0 0 0 0 0 0 0 0 0 0 0 0 0 0 0 0 0 0 0 0 0 0 0 0 0 0 0 0 0 0 0 0 0 0 0 0 0 0 0 0 0 0 0 0 0 0 0 0 0 0 0 0 0 0 0 0 0 0 0 0 0 0 0 0 0 0 0 0 0 0 0 0 0 0 0 0 0 0 0 0 0 0 0 0 0 0 0 0 0 0 0 0 0 0 0 0 0 0 0 0 0 0 0 0 0 0 0 0 0 0 0 0 0 0 0 0 0 0 0 0 0 0 0 0 0 0 0 0 0 0 0 0 0 0 0 0 0 0 0 0 0 0 0 0 0 0 0 0 0 0 0 0 0 0 0 0 0 0 0 0 0 0 0 0 0 0 0 0 0 0 0 0 0 0 0 0 0 0 0 0 0 0 0 0 0 0 0 0 0 0 0 0 0 0 0 0 0 0 0 0 0 0 0 0 0 0 0 0 0 0 0 0 0 0 0 0 0 0 0 0 0 0 0 0 0 0 0 0 0 0 0 0 0 0 0 0 0 0 0 0 0 0 0 0 0 0 0 0 0 0 0 0 0 0 0 0 0 0 0 0 0 0 0 0 0 0 0 0 0 0 0 0 0 0 0 0 0 0 0 0 0 0 0 0 0 0 0 0 0 0 0 0 0 0 0 0 0 0 0 0 0 0 0 0 0 0 0 0 0 0 0 0 0 0 0 0 0 0 0 0 0 0 0 0 0 0 0 0 0 0 0 0 0 0 0 0 0 0 0 0 0 0 0 0 0 0 0 0 0 0 0 0 0 0 0 0 0 0 0 0 0 0 0 0 0 0 0 0 0 0 0 0 0 0 0 0 0 0 0 0 0 0 0 0 0 0 0 0 0 0 0 0 0 0 0 0 0 0 0 0 0 0 0 0 0 0 0 0 0 0 0 0 0 0 0 0 0 0 0 0 0 0 0 0 0 0 0 0 0 0 0 0 0 0 0 0 0 0 0 0 0 0 0 0 0 0 0 0 0 0 0 0 0 0 0 0 0 0 0 0 0 0 0 0 0 0 0 0 0 0 0 0 0 0 0 0 0 0 0 0 0 0 0 0 0 0 0 0 0 0 0 0 0 0 0 0 0 0 0 0 0 0 0 0 0 0 0 0 0 0 0 0 0 0 0 0 0 0 0 0 0 0 0 0 ...(+27038 chars)]  downsampling=1  samplingPeriod=SIM.StepSize.v  uuid=0  ASMProperties=struct('Name','mdld_data_capture','Version','1.0','Library','mdld_utils_lib')  startTriggerDelay=0  startTriggerLogic=0  startTriggerCount=0  startTriggerConditions=[0,0,0,0,0,0,0,0,0]  stopTriggerDelay=0  stopTriggerLogic=0  stopTriggerCount=0  stopTriggerConditions=[0,0,0,0,0,0,0,0,0]
  Maneuver : BusSelector  OutputSignals=ManeuverScheduler,UserSignals_Customized
  ManeuverScheduler : BusSelector  OutputSignals=MdlControl,InitialVehStates,ModeSignals,RefSignals,Parameters,UserSignals,Info
  Manifold : BusSelector  OutputSignals=Pos_AccPedal[%],p_Manifold[bar]
  ManifoldValve : BusSelector  OutputSignals=p_In_MainfoldValve[bar],p_Out_MainfoldValve[bar],T_In_MainfoldValve[degC],m_dot_ManifoldValve[Kg|s],m_dot_Out_ManifoldValve[Kg|s],m_dot_In_ManifoldValve[Kg|s]
  ManualTransmission : BusSelector  OutputSignals=Clutch,GearBox
  MassForcesAndTorques : BusSelector  OutputSignals=GravitationalForces,GyroscopicForces,GyroscopicTorques,ResidualAccelerations
  MasterBrakeCylinder : BusSelector  OutputSignals=ActiveBrakeCylinder,BrakeCylinderLinear,BrakeCylinderPhysical
  MaximumTorque : BusSelector  OutputSignals=Trq_FL_max_Brake[Nm],Trq_FR_max_Brake[Nm],Trq_RL_max_Brake[Nm],Trq_RR_max_Brake[Nm]
  MdlControl : BusSelector  OutputSignals=Reset_VehicleStates[0|1],RoadControl[],Get_VehPos_Trigger[],Keep_VehiclePosition[0|1]
  Measurement_Points : BusSelector  OutputSignals=Distance_MeasPnt_Marker_Left[m],Distance_MeasPnt_Marker_Right[m],Velocity_MeasPnt_Marker_Left[m|s],Velocity_MeasPnt_Marker_Right[m|s]
  ModeSignals : BusSelector  OutputSignals=AccBr_Mode[1Stim|2Driver],GearClutch_Mode[1Stim|2Driver|3OpenClutch|4RefGear],Steer_Mode[1Stim|2Driver|3Fix],Road_Mode[1NoRoad|2Straight|3Circle|4Road],LatDriver[1LatCtrl1|2LatCtrl2],LatCtrl_Mode[1Pos|2Yaw],AdaptVelocityToRoad_Mode[1Off|2On],ForceToRoad_Mode[1Off|2On],SelectorLever_Mode[1Stim|2Driver],CurvatureCalculation_Mode[1Road|2Driver]
  Network_Item : BusSelector  OutputSignals=Network_Item_ID[],Network_Item_Type[],Network_Item_Type_Absolute[],Preferred_Lane_Direct[],Preferred_Lane_Oncoming[]
  Object{1..5} (5 alike) : BusSelector  OutputSignals=Object_Valid[0|1],Object_ID[],Object_Type[],Pos_x_CoorSys_S[m],Pos_y_CoorSys_S[m],Pos_z_CoorSys_S[m],Angle_Hor_Rel[deg],Angle_Ver_Rel[deg],Distance[m],Network_Item_Type[0Junction|1Road],Network_Item_ID[],Parent_Object_ID[],CustomValues[]
  ObjectParameters : BusSelector  OutputSignals=FellowsGeometry,TrafficObjects,DiscreteObjects
  Object_Sensor_2D : BusSelector  OutputSignals=Sample_Pulse,Sensor_Scheduler,Sensor_1_Front,Sensor_2_Front_Left,Sensor_3_Left,Sensor_4_Rear_Left,Sensor_5_Front_Right,Sensor_6_Right,Sensor_7_Rear_Right
  Object_Sensor_3D : BusSelector  OutputSignals=Sample_Pulse,Sensor_Scheduler,Sensor_1_Front_Long,Sensor_2_Front_Mid,Sensor_3_Rear
  Operator_Interface_ACC : BusSelector  OutputSignals=Sw_ACC_On[0Off|1On],Sw_ACC_Off[0Off|1On],Sw_ACC_Cancel[0Off|1On],Sw_ACC_Resume[0Off|1On],Sw_ACC_Speed_Set[0Off|1On],Sw_ACC_Speed_Increase[0Off|1On],Sw_ACC_Speed_Decrease[0Off|1On],ACC_State[1OFF|2Standby|3ON],V_Set_CruiseControl[km|h]
  Orientation_Left : BusSelector  OutputSignals=Angle_FL_Wheel[Alpha;Beta;Gamma][deg],w_Rel_FL_Wheel_dq1_Front_dt[x;y;z][],w_Rel_FL_Wheel_dq2_Front_dt[x;y;z][],w_Rel_FL_Wheel_dDispl_SteeringRod_dt[x;y;z][rad|m],UnitVec_y_Wheel_FL_CoorSys_V[x;y;z]
  Orientation_Left1 : BusSelector  OutputSignals=Angle_RL_Wheel[Alpha;Beta;Gamma][deg],w_Rel_RL_Wheel_dq1_Rear_dt[x;y;z][],w_Rel_RL_Wheel_dq2_Rear_dt[x;y;z][],w_Rel_RL_Wheel_dDispl_SteeringRod_dt[x;y;z][rad|m],UnitVec_y_Wheel_RL_CoorSys_V[x;y;z]
  Orientation_Right : BusSelector  OutputSignals=Angle_FR_Wheel[Alpha;Beta;Gamma][deg],w_Rel_FR_Wheel_dq1_Front[x;y;z][],w_Rel_FR_Wheel_dq2_Front[x;y;z][],w_Rel_FR_Wheel_dDispl_SteeringRod_dt[x;y;z][rad|m],UnitVec_y_Wheel_FR_CoorSys_V[x;y;z]
  Orientation_Right1 : BusSelector  OutputSignals=Angle_RR_Wheel[Alpha;Beta;Gamma][deg],w_Rel_RR_Wheel_dq1_Rear[x;y;z][],w_Rel_RR_Wheel_dq2_Rear[x;y;z][],w_Rel_RR_Wheel_dDispl_SteeringRod_dt[x;y;z][rad|m],UnitVec_y_Wheel_RR_CoorSys_V[x;y;z]
  OutputPoint : BusSelector  OutputSignals=F_OutputPoint[N],p_OutputPoint[bar],Pos_BrakePedal_OutputPoint[%],F_Max_Pedal[N],p_Max_Booster[bar]
  OutputSignals : BusSelector  OutputSignals=Pos_AccPedal[%],Pos_BrakePedal[%],Pos_ClutchPedal[%],Gear[],t_Preview_vRef[s],Angle_SteeringWheel[deg],AutomaticTrmCtrlSignals,StartButtonSignals,ParkingBrakeSignals
  Parameter : BusSelector  OutputSignals=Sensor_Enable[0Off|1On],SensorIdx[],t_Offs_Sensor[s],t_Cycle_Sensor[s],t_Delay_SensorOutput[s],Geometry[],Pos_Sensor_Apex_CoorSys_V[x;y;z][m],Angle_Orientation_Sensor_CoorSys_V[x;y;z][deg],Length_ScopeZone[m],Angle_ScopeZone_Horizontal[deg],Angle_ScopeZone_Vertical[deg],Length_ScopeZone_Head[m],Length_BlindZone[m],Occlusion_Mode[1No_Occlusion|2Basic_3D|3Occlusion_Ratio_3D],Threshold_Occlusion_Ratio[0_1],Object_Points_Calculation_Enable[0Off|1On],Object_Points_Occlusion_Enable[0Off|1On]
  Parameter1 : BusSelector  OutputSignals=Sensor_Enable[0Off|1On],SensorIdx[],t_Offs_Sensor[s],t_Cycle_Sensor[s],t_Delay_SensorOutput[s],Geometry[],Pos_Sensor_Apex_CoorSys_V[x;y;z][m],Angle_Orientation_Sensor_CoorSys_V[x;y;z][deg],Length_ScopeZone[m],Angle_ScopeZone_Horizontal[deg],Angle_ScopeZone_Vertical[deg],Length_ScopeZone_Head[m],Length_BlindZone[m],Occlusion_Mode[1No_Occlusion|2Basic_3D|3Occlusion_Ratio_3D],Threshold_Occlusion_Ratio[0_1],Object_Points_Calculation_Enable[0Off|1On],Object_Points_Occlusion_Enable[0Off|1On]
  Parameter2 : BusSelector  OutputSignals=Sensor_Enable[0Off|1On],SensorIdx[],t_Offs_Sensor[s],t_Cycle_Sensor[s],t_Delay_SensorOutput[s],Geometry[],Pos_Sensor_Apex_CoorSys_V[x;y;z][m],Angle_Orientation_Sensor_CoorSys_V[x;y;z][deg],Length_ScopeZone[m],Angle_ScopeZone_Horizontal[deg],Angle_ScopeZone_Vertical[deg],Length_ScopeZone_Head[m],Length_BlindZone[m],Occlusion_Mode[1No_Occlusion|2Basic_3D|3Occlusion_Ratio_3D],Threshold_Occlusion_Ratio[0_1],Object_Points_Calculation_Enable[0Off|1On],Object_Points_Occlusion_Enable[0Off|1On]
  Parameters : BusSelector  OutputSignals=Enable_Evaluation[0|1],Evaluation_Distance[m],Border_Mode[0Center|1Inner|2Outer],Enable_Junction_Evaluation[0|1],Num_Lanes[Left;Right],Enable_MeasPoint[0|1],MeasPoint_1_CoorSysV[x;y][m],MeasPoint_2_CoorSysV[x;y][m],MeasPoint_3_CoorSysV[x;y][m],MeasPoint_4_CoorSysV[x;y][m],MeasPoint_1_CoorSysE[x;y][m],MeasPoint_2_CoorSysE[x;y][m],MeasPoint_3_CoorSysE[x;y][m],MeasPoint_4_CoorSysE[x;y][m]
  Parameters1 : BusSelector  OutputSignals=a_x_Max[m|s2],a_x_Brake_Threshold[m|s2],a_y_Max[m|s2],Curv_Road_Circle[1|m],Gear_Max[],Width_Deadzone_LatCtrl[m],v_Lat[m|s],Object_Type_ID[]
  Parameters10 : BusSelector  OutputSignals=Sensor_Enable[0Off|1On],Pos_Sensor_Apex_CoorSys_V[x;y;z][m],Angle_Orientation_Sensor_CoorSys_V[x;y;z][deg],Length_ScopeZone[m],Angle_ScopeZone_Horizontal[deg],Angle_ScopeZone_Vertical[deg]
  Parameters{2..8} (7 alike) : BusSelector  OutputSignals=Sensor_Enable[0Off|1On],SensorIdx[],t_Offs_Sensor[s],t_Cycle_Sensor[s],t_Delay_SensorOutput[s],Pos_Sensor_Apex_CoorSys_V[x;y;z][m],Angle_z_Orientation_Sensor_CoorSys_V[deg],Angle_ScopeZone_Horizontal[deg],Length_ScopeZone[m],Num_SensorRays_Used[],Sensor_Detection_Mode[1Ray|2Sector],Object_Detection_Mode[1Object|2Continuous|3All]
  Parameters9 : BusSelector  OutputSignals=Sensor_Enable[0Off|1On],Pos_Sensor_Apex_CoorSys_V[x;y;z][m],Angle_Orientation_Sensor_CoorSys_V[x;y;z][deg],Length_ScopeZone[m],Angle_ScopeZone_Horizontal[deg],Angle_ScopeZone_Vertical[deg],Angle_Sign_Orientation_Max[deg]
  ParkingBrakeSignals : BusSelector  OutputSignals=Sw_ParkingBrake[0Off|1On]
  Pos_Fellows_MainPnt_CoorSys_E[x;y;z][m] : BusSelector  OutputSignals=Pos_x_Fellows[m],Pos_y_Fellows[m],Pos_z_Fellows[m]
  Pos_Junction_Border_Animation_CoorSys_E : BusSelector  OutputSignals=Pos_x_Junction_Border_Animation_CoorSys_E,Pos_y_Junction_Border_Animation_CoorSys_E,Pos_z_Junction_Border_Animation_CoorSys_E
  Pos_Junction_Shape_ContObj_Animation_CoorSys_E : BusSelector  OutputSignals=Pos_x_Junction_Shape_ContObj_Animation_CoorSys_E,Pos_y_Junction_Shape_ContObj_Animation_CoorSys_E,Pos_z_Junction_Shape_ContObj_Animation_CoorSys_E
  Pos_Junction_Shape_Line_Animation_CoorSys_E : BusSelector  OutputSignals=Pos_x_Junction_Shape_Line_Animation_CoorSys_E,Pos_y_Junction_Shape_Line_Animation_CoorSys_E,Pos_z_Junction_Shape_Line_Animation_CoorSys_E
  Pos_Road_Lane_Animation_CoorSys_E : BusSelector  OutputSignals=Pos_x_Road_Lane_Animation_CoorSys_E,Pos_y_Road_Lane_Animation_CoorSys_E,Pos_z_Road_Lane_Animation_CoorSys_E
  Pos_Road_Shape_ContObj_Animation_CoorSys_E : BusSelector  OutputSignals=Pos_x_Road_Shape_ContObj_Animation_CoorSys_E,Pos_y_Road_Shape_ContObj_Animation_CoorSys_E,Pos_z_Road_Shape_ContObj_Animation_CoorSys_E
  Pos_Road_Shape_Line_Animation_CoorSys_E : BusSelector  OutputSignals=Pos_x_Road_Shape_Line_Animation_CoorSys_E,Pos_y_Road_Shape_Line_Animation_CoorSys_E,Pos_z_Road_Shape_Line_Animation_CoorSys_E
  Pos_Vehicle_CoorSys_E[x;y;z][m] : BusSelector  OutputSignals=Pos_x_Vehicle_CoorSys_E[m],Pos_y_Vehicle_CoorSys_E[m],Pos_z_Vehicle_CoorSys_E[m]
  Pos_Vehicle_GPS[Long;Lat][deg] : BusSelector  OutputSignals=Longitude[deg],Latitude[deg]
  Pos_Vehicle_Init_CoorSys_E[x;y;z][m] : BusSelector  OutputSignals=Const_Pos_x_Vehicle_Init[m],Const_Pos_y_Vehicle_Init[m],Const_Pos_z_Vehicle_Init[m]
  Pos_Wheel[FL;FR][x;y;z][m] : BusSelector  OutputSignals=Pos_FL_Wheel[x;y;z][m],Pos_FR_Wheel[x;y;z][m]
  Pos_Wheel[RL;RR][x;y;z][m] : BusSelector  OutputSignals=Pos_RL_Wheel[x;y;z][m],Pos_RR_Wheel[x;y;z][m]
  PositionError : BusSelector  OutputSignals=e_Lat[m],e_Lat_Abs[m],e_Lat_Total[m]
  Position_Left : BusSelector  OutputSignals=Pos_FL_Wheel[x;y;z][m],Pos_FL_Wheel_dq1_Front[x;y;z][],Pos_FL_Wheel_dq2_Front[x;y;z][],Pos_FL_Wheel_dDispl_SteeringRod[x;y;z][]
  Position_Left1 : BusSelector  OutputSignals=Pos_RL_Wheel[x;y;z][m],Pos_RL_Wheel_dq1_Rear[x;y;z][],Pos_RL_Wheel_dq2_Rear[x;y;z][],Pos_RL_Wheel_dDispl_SteeringRod[x;y;z][]
  Position_Right : BusSelector  OutputSignals=Pos_FR_Wheel[x;y;z][m],Pos_FR_Wheel_dq1_Front[x;y;z][],Pos_FR_Wheel_dq2_Front[x;y;z][],Pos_FR_Wheel_dDispl_SteeringRod[x;y;z][]
  Position_Right1 : BusSelector  OutputSignals=Pos_RR_Wheel[x;y;z][m],Pos_RR_Wheel_dq1_Rear[x;y;z][],Pos_RR_Wheel_dq2_Rear[x;y;z][],Pos_RR_Wheel_dDispl_SteeringRod[x;y;z][]
  Positions : BusSelector  OutputSignals=Vehicle,Wheels
  Pressure : BusSelector  OutputSignals=p_FL_Brake[bar],p_FR_Brake[bar],p_RL_Brake[bar],p_RR_Brake[bar]
  Pressure1 : BusSelector  OutputSignals=p_FL_Brake[bar],p_FR_Brake[bar],p_RL_Brake[bar],p_RR_Brake[bar]
  PushRod : BusSelector  OutputSignals=F_Pedal[N],F_Spring[N],F_RearChamber[N],F_VacuumChamber[N],F_PushRod[N],x[m],V_delta[m3],A_Diaphragm[m2],OutputPoint
  RadarEffects : BusSelector  OutputSignals=ID[],Object_ID[],Dist_CoorSys_S[m],Angle_Hor_CoorSys_S[deg],Pos_ObjectPoint_CoorSys_E[x;y;z][m]
  RadarEffects1 : BusSelector  OutputSignals=ID[],Object_ID[],Dist_CoorSys_S[m],Angle_Hor_CoorSys_S[deg],Pos_ObjectPoint_CoorSys_E[x;y;z][m]
  RadarEffects2 : BusSelector  OutputSignals=ID[],Object_ID[],Dist_CoorSys_S[m],Angle_Hor_CoorSys_S[deg],Pos_ObjectPoint_CoorSys_E[x;y;z][m]
  RearChamber : BusSelector  OutputSignals=m_dot_In_RearChamber[kg|s],m_dot_Out_RearChamber[kg|s],T_RearChamber[degC],p_RearChamber[bar],V_RearChamber[m3]
  RearDifferential : BusSelector  OutputSignals=omega_Out_Lef_RearDifferentialt[rad|s],omega_Out_Right_RearDifferential[rad|s],omega_In_CentralDiff_RearDifferential[rad|s],Trq_Lock_RearDifferential[Nm],omega_Cage[rad|s],Const_i_MainReductionGear[],Const_TrqDistribution[]
  RefSignals : BusSelector  OutputSignals=Pos_AccPedal_Maneuver[%],Pos_BrakePedal_Maneuver[%],Pos_ClutchPedal_Maneuver[%],Gear_Maneuver[],Angle_SteeringWheel_Maneuver[deg],v_Vehicle_Ref_Maneuver[m|s],d_Maneuver[m],LaneIdx_Maneuver[],Dist_Def_Maneuver[],v_Vehicle_Ref_Preview_Maneuver[m|s],v_Vehicle_Ref_Preview_State[0Invalid|1CurrentSeg|2NextSeg],Sw_SteeringMode_Maneuver[1Angle|2Trq],Trq_Steering_Maneuver[Nm],SelectorLever_Maneuver[],Dist_Def_Refline_Maneuver[]
  ReferenceVelocity : BusSelector  OutputSignals=v_Road[km|h],s_Preview_vRef[m],a_x_Vehicle_Ref[m|s2],v_Vehicle_Ref[m|s],v_Vehicle_Ref[km|h]
  RelativePositionFront : BusSelector  OutputSignals=Pos_Wheel[FL;FR][x;y;z][m],UnitVec_y_Wheel_CoorSys_V[FL;FR][x;y;z],Angle_Wheel[FL;FR][Toe;Camber][deg]
  RelativePositionRear : BusSelector  OutputSignals=Pos_Wheel[RL;RR][x;y;z][m],UnitVec_y_Wheel_CoorSys_V[RL;RR][x;y;z],Angle_Wheel[RL;RR][Toe;Camber][deg]
  Reshape_{55..56,75,79..82,91..102,120..171,173..174,176..197,199,219,239,259,286..293,427..430,434..437,445..448,452..455,469..476,519..522,527..530,534..537,545..548,552..555,569..576,619..622,753,773,775..787,803..822,840..841,844..853,869,879,889..944,975,981,1035..1062,1065..1070,1092..1101,1110..1113,1120..1121,1132..1161,1168..1169,1180..1209,1216..1217,1228..1257,1262..1265,1271,1281..1288,1296,1306..1313,1321,1331..1338,1346,1356..1363,1371,1381..1388,1396,1406..1413,1421,1431..1438,1443..1463,1465..1466,1486,1499,1512,1525,1538,1540..1541,1545,1554..1571,1577..1583} (537 alike) : Reshape
  ResidualAccelerations : BusSelector  OutputSignals=a_Vehicle_CoG_Residual[x;y;z][m|s2],a_FL_Residual[x;y;z][m|s2],a_FR_Residual[x;y;z][m|s2],a_RL_Residua[x;y;z]l[m|s2],a_RR_Residual[x;y;z][m|s2]
  RightSide : BusSelector  OutputSignals=Pos_Right[x;y;z][m],Yaw_Angle_Right[deg],Yaw_Angle_RelVehicle_Right[deg],Curvature_Right[1|m],MarkerType_Right[],MarkerWidth_Right[m],MarkerColor_Right[],LineID_1_Right[],LineID_2_Right[],Distance_Marker_Right[m]
  Road : BusSelector  OutputSignals=Road_Init,Road_ASMVeh,Road_ContactPoints,Road_Preview,Road_Info,Road_TrafficFellows,UserSignals,UserSignals_Customized,Pos_Vehicle_GPS[Long;Lat][deg],Ambient,LaneSensor_Dynamic
  Road_ASMVeh : BusSelector  OutputSignals=s_Veh_Road[m],s_Total_Veh_Road[m],d_Total_Veh_Road[m],s_Veh_Road_Trj[m],LaneIdx_Total_Veh_Road[],Curv_Veh_Road[1|m],Pos_x_Ref_Veh_Road[m],Pos_y_Ref_Veh_Road[m],Angle_Yaw_Veh_Road[deg],Slope_Veh_Road[%],v_Wind_Coor_Sys_E[x;y;z][m|s],Slope_Lateral_Veh_Road[deg]
  Road_ContactPoints : BusSelector  OutputSignals=Pos_z_CP[:][m],Fric_Coeff_CP[:][],UnitVec_z_CP[:][x;y;z],Sw_Tire_Parameter_Set_CP[:][1|2|3|4]
  Road_Info : BusSelector  OutputSignals=RoadState[],RouteLength_Veh[m],Flag_RouteClosed_Veh[0|1],Dist_Response_Maneuver,Speed_Limit_Veh[km|h],Network_Item_Type_Veh[],Network_Item_Id_Veh[],RoadSegment_Veh[],LaneSection_Veh[],RoadWidth_Veh[m],Network_Load_Idx[],d_Veh_Ref_Line[m],Dist_Border_Left[m],Dist_Border_Right[m]
  Road_Init : BusSelector  OutputSignals=Pos_Vehicle_Init_CoorSys_E[x;y;z][m],Angle_Vehicle_Init_CoorSys_E[x;y;z][rad]
  Road_Preview : BusSelector  OutputSignals=Pos_x_Preview_Road[m],Pos_y_Preview_Road[m],Curv_Preview_Road[1|m],Speed_Limit_Preview_Road[km|h],Pos_z_Preview_Road[m],Roll_Preview_Road[deg],Pitch_Preview_Road[deg],x_Preview_DriverCurv[m],y_Preview_DriverCurv[m]
  Road_TrafficFellows : BusSelector  OutputSignals=Pos_x_Fellows_Road[m],Pos_y_Fellows_Road[m],Pos_z_Fellows_Road[m],Angle_Yaw_Fellows_Road[deg],Angle_Pitch_Fellows_Road[deg],Angle_Roll_Fellows_Road[deg],Curv_Fellows_Road[1|m],d_Total_Fellows_Road[m],LaneIdx_Total_Fellows_Road[],RoadSegment_Fellows[],LaneSection_Fellows[],Speed_Limit_Fellows[],Network_Item_Type_Fellows[],Network_Item_Id_Fellows[],d_Fellows_RefLine[m],RouteLength_Fellows[m],Flag_RouteClosed_Fellows[0|1],Dist_Response_Traffic,Angle_Yaw_Fellows_RoadRefline[deg]
  RotationAngle : BusSelector  OutputSignals=Angle_Rot_FL_Wheel[deg],Angle_Rot_FR_Wheel[deg],Angle_Rot_RL_Wheel[deg],Angle_Rot_RR_Wheel[deg]
  SFunction_Info : BusSelector  OutputSignals=Sfcn_State[0|1],Input_Data_Valid[0|1],Data_Valid[0|1]
  Sample_Pulse : BusSelector  OutputSignals=Pulse[0|1]
  Sample_Pulse1 : BusSelector  OutputSignals=Pulse[0|1]
  Sensor1 : BusSelector  OutputSignals=a_Angular_Sensor1_CoorSys_V[x;y;z][rad|s2],a_Total_Sensor1_CoorSys_V[x;y;z][m|s2],a_Sensor1_CoorSys_V[x;y;z][m|s2],v_Sensor1_CoorSys_V[x;y;z][m|s],w_Sensor1_CoorSys_V[x;y;z][rad|s],a_Angular_Sensor1_CoorSys_VH[x;y;z][rad|s2],a_Total_Sensor1_CoorSys_VH[x;y;z][m|s2],a_Sensor1_CoorSys_VH[x;y;z][m|s2],v_Sensor1_CoorSys_VH[x;y;z][m|s],w_Sensor1_CoorSys_VH[x;y;z][rad|s]
  Sensor2 : BusSelector  OutputSignals=a_Angular_Sensor2_CoorSys_V[x;y;z][rad|s2],a_Total_Sensor2_CoorSys_V[x;y;z][m|s2],a_Sensor2_CoorSys_V[x;y;z][m|s2],v_Sensor2_CoorSys_V[x;y;z][m|s],w_Sensor2_CoorSys_V[x;y;z][rad|s],a_Angular_Sensor2_CoorSys_VH[x;y;z][rad|s2],a_Total_Sensor2_CoorSys_VH[x;y;z][m|s2],a_Sensor2_CoorSys_VH[x;y;z][m|s2],v_Sensor2_CoorSys_VH[x;y;z][m|s],w_Sensor2_CoorSys_VH[x;y;z][rad|s]
  Sensor3 : BusSelector  OutputSignals=a_Angular_Sensor3_CoorSys_V[x;y;z][rad|s2],a_Total_Sensor3_CoorSys_V[x;y;z][m|s2],a_Sensor3_CoorSys_V[x;y;z][m|s2],v_Sensor3_CoorSys_V[x;y;z][m|s],w_Sensor3_CoorSys_V[x;y;z][rad|s],a_Angular_Sensor3_CoorSys_VH[x;y;z][rad|s2],a_Total_Sensor3_CoorSys_VH[x;y;z][m|s2],a_Sensor3_CoorSys_VH[x;y;z][m|s2],v_Sensor3_CoorSys_VH[x;y;z][m|s],w_Sensor3_CoorSys_VH[x;y;z][rad|s]
  Sensor4 : BusSelector  OutputSignals=a_Angular_Sensor4_CoorSys_V[x;y;z][rad|s2],a_Total_Sensor4_CoorSys_V[x;y;z][m|s2],a_Sensor4_CoorSys_V[x;y;z][m|s2],v_Sensor4_CoorSys_V[x;y;z][m|s],w_Sensor4_CoorSys_V[x;y;z][rad|s],a_Angular_Sensor4_CoorSys_VH[x;y;z][rad|s2],a_Total_Sensor4_CoorSys_VH[x;y;z][m|s2],a_Sensor4_CoorSys_VH[x;y;z][m|s2],v_Sensor4_CoorSys_VH[x;y;z][m|s],w_Sensor4_CoorSys_VH[x;y;z][rad|s]
  SensorIndex{,1..9} (10 alike) : BusSelector  OutputSignals=Idx_Sensor[]
  SensorMotion : BusSelector  OutputSignals=Sensor1,Sensor2,Sensor3,Sensor4
  SensorOutput : BusSelector  OutputSignals=v_Rel_Object[m|s],a_Rel_Object[m|s2],Dist_Object[m],Angle_Hor_Object[deg],Angle_Ver_Object[deg],Pos_Sensor_Apex_E[x;y;z][m],Pos_Object_NearestPnt_E[x;y;z][m],Object_Info[-1None|1Fellow|2Static],Object_ID[],Object_Type[],Occlusion_Ratio_Object[-1|0_1],Flag_NearestPnt_Occluded[-1|0|1],Pos_NearestSurf_Pnt1_CoorSys_S[x;y;z][m],Pos_NearestSurf_Pnt2_CoorSys_S[x;y;z][m],Pos_NearestSurf_Pnt3_CoorSys_S[x;y;z][m],Pos_NearestSurf_Pnt4_CoorSys_S[x;y;z][m],NearestSurf_Pnts_Index[],NearestSurf_Index[]
  SensorOutput1 : BusSelector  OutputSignals=v_Rel_Object[m|s],a_Rel_Object[m|s2],Dist_Object[m],Angle_Hor_Object[deg],Angle_Ver_Object[deg],Pos_Sensor_Apex_E[x;y;z][m],Pos_Object_NearestPnt_E[x;y;z][m],Object_Info[-1None|1Fellow|2Static],Object_ID[],Object_Type[],Occlusion_Ratio_Object[-1|0_1],Flag_NearestPnt_Occluded[-1|0|1],Pos_NearestSurf_Pnt1_CoorSys_S[x;y;z][m],Pos_NearestSurf_Pnt2_CoorSys_S[x;y;z][m],Pos_NearestSurf_Pnt3_CoorSys_S[x;y;z][m],Pos_NearestSurf_Pnt4_CoorSys_S[x;y;z][m],NearestSurf_Pnts_Index[],NearestSurf_Index[]
  SensorOutput10 : BusSelector  OutputSignals=Object1,Object2,Object3,Object4,Object5
  SensorOutput11 : BusSelector  OutputSignals=Collision_Flag[0NoCollision|1Collision],Collision_Flag_Held[0NoCollision|1Collision],Object_ID[],Time_Collision[s],Pos_Collision_Point[x;y][m],v_Collision_CoG_Vehicle[x;y][m|s],v_Collision_CoG_Vehicle_Total[m|s],v_Rel_Collision_Point[x;y][m|s],v_Rel_Collision_Point_Total[m|s]
  SensorOutput2 : BusSelector  OutputSignals=v_Rel_Object[m|s],a_Rel_Object[m|s2],Dist_Object[m],Angle_Hor_Object[deg],Angle_Ver_Object[deg],Pos_Sensor_Apex_E[x;y;z][m],Pos_Object_NearestPnt_E[x;y;z][m],Object_Info[-1None|1Fellow|2Static],Object_ID[],Object_Type[],Occlusion_Ratio_Object[-1|0_1],Flag_NearestPnt_Occluded[-1|0|1],Pos_NearestSurf_Pnt1_CoorSys_S[x;y;z][m],Pos_NearestSurf_Pnt2_CoorSys_S[x;y;z][m],Pos_NearestSurf_Pnt3_CoorSys_S[x;y;z][m],Pos_NearestSurf_Pnt4_CoorSys_S[x;y;z][m],NearestSurf_Pnts_Index[],NearestSurf_Index[]
  SensorOutput{3..9} (7 alike) : BusSelector  OutputSignals=Angle_Hor_Rel[deg],Object_ID[],Object_Type[],Distance[m],v_Rel[m|s],a_Rel[m|s2],Height_Min[m],Height_Max[m]
  SensorOutput[] : BusSelector  OutputSignals=Traffic_Sign_Valid[0|1],TrafficObject_ID[],TrafficObject_Type[],Pos_CoorSys_E[x;y;z][m],Angle_CoorSys_E[x;y;z][deg],Pos_CoorSys_S[x;y;z][m],Angle_Hor_Rel[deg],Angle_Ver_Rel[deg],Angle_Sign_Orientation_Rel[deg],Distance[m],Traffic_Sign_Type[],Traffic_Sign_Subtype[],Traffic_Sign_Value[],Traffic_Sign_Country[],Traffic_Sign_Visibility[0_100],Traffic_Sign_Lanes[],Object_Stream_ID[],Object_State[],Parent_Object_ID[],Network_Item_Type[0Junction|1Road],Network_Item_ID[]
  SensorStatus{,1..6} (7 alike) : BusSelector  OutputSignals=Flag_Object_In_Scope[0Out|1In],Flag_Sensor_Apex_In_Object[0Out|1In]
  Sensor_1_Front : BusSelector  OutputSignals=Parameters,SensorIndex,SensorStatus,SensorOutput,Info
  Sensor_1_Front_Long : BusSelector  OutputSignals=Parameter,SensorIndex,Info,SensorOutput,RadarEffects,CustomPoints
  Sensor_2_Front_Left : BusSelector  OutputSignals=Parameters,SensorIndex,SensorStatus,SensorOutput,Info
  Sensor_2_Front_Mid : BusSelector  OutputSignals=Parameter,SensorIndex,Info,SensorOutput,RadarEffects,CustomPoints
  Sensor_3_Left : BusSelector  OutputSignals=Parameters,SensorIndex,SensorStatus,SensorOutput,Info
  Sensor_3_Rear : BusSelector  OutputSignals=Parameter,SensorIndex,Info,SensorOutput,RadarEffects,CustomPoints
  Sensor_4_Rear_Left : BusSelector  OutputSignals=Parameters,SensorIndex,SensorStatus,SensorOutput,Info
  Sensor_5_Front_Right : BusSelector  OutputSignals=Parameters,SensorIndex,SensorStatus,SensorOutput,Info
  Sensor_6_Right : BusSelector  OutputSignals=Parameters,SensorIndex,SensorStatus,SensorOutput,Info
  Sensor_7_Rear_Right : BusSelector  OutputSignals=Parameters,SensorIndex,SensorStatus,SensorOutput,Info
  Sensor_Front_1 : BusSelector  OutputSignals=Info,SensorOutput[],Parameters
  Sensor_Front_2 : BusSelector  OutputSignals=Info,SensorOutput,Parameters
  Sensor_Output : BusSelector  OutputSignals=SFunction_Info,Network_Item,CurrentLane,Lanes_Left,Lanes_Right,Measurement_Points
  Sensor_Scheduler : BusSelector  OutputSignals=SensorEnable[0Off|1On],SensorIdx_Selected[],Conflict_Flag[0|1],CylceConflict_Info[],IndexConflict_Info[],SensorSelection_Data[0|1],DelayPulse_SensorOutput[0|1]
  Sensor_Scheduler1 : BusSelector  OutputSignals=SensorEnable[0Off|1On],SensorIdx_Selected[],Conflict_Flag[0|1],CylceConflict_Info[],IndexConflict_Info[],SensorSelection_Data[0|1],DelayPulse_SensorOutput[0|1]
  Sensors : BusSelector  OutputSignals=Object_Sensor_3D,Object_Sensor_2D,TrafficSign_Sensor_Dyn,Custom_Sensor,Line_Sensor,Collision_Sensor,Sensors_Common
  Sensors_Common : BusSelector  OutputSignals=Enable_SensorScheduling[0Off|1On]
  Shaft_CF : BusSelector  OutputSignals=Trq_CF_Shaft[Nm],omega_Delta_CF_Shaft[rad|s]
  Shaft_CR : BusSelector  OutputSignals=Trq_CR_Shaft[Nm],omega_Delta_CR_Shaft[rad|s]
  Shaft_FL : BusSelector  OutputSignals=Trq_FL_Shaft[Nm],omega_Delta_FL_Shaft[rad|s]
  Shaft_FR : BusSelector  OutputSignals=Trq_FR_Shaft[Nm],omega_Delta_FR_Shaft[rad|s]
  Shaft_RL : BusSelector  OutputSignals=Trq_RL_Shaft[Nm],omega_Delta_RL_Shaft[rad|s]
  Shaft_RR : BusSelector  OutputSignals=Trq_RR_Shaft[Nm],omega_Delta_RR_Shaft[rad|s]
  Shaft_TGCL4WD : BusSelector  OutputSignals=Trq_TGCL4WD_Shaft[Nm],omega_Delta_TGCL4WD_Shaft[rad|s]
  ShaftsTorques_CoorSys_V : BusSelector  OutputSignals=Trq_Shaft_FL_CoorSys_V[x;y;z][Nm],Trq_Shaft_FR_CoorSys_V[x;y;z][Nm],Trq_Shaft_RL_CoorSys_V[x;y;z][Nm],Trq_Shaft_RR_CoorSys_V[x;y;z][Nm]
  Shift_Lock_Control : BusSelector  OutputSignals=Ctrl_Parking_Pawl[0|1]
  Shift_Strategy : BusSelector  OutputSignals=Gear_Requested[]
  SignalFilter : Mux  Inputs=1584
  SignalFilterGain : Gain  SaturateOnIntegerOverflow=on  OutDataTypeStr=Inherit: Same as input  ParamDataTypeStr=Inherit: Same as input
  SoftECU : BusSelector  OutputSignals=SoftECU_Engine,SoftECU_Brake,SoftECU_ACC,SoftECU_Transmission,SoftECU_PowerSteering,SoftECU_StartButton
  SoftECU_ACC : BusSelector  OutputSignals=Controller_ACC,Interface_ACC,Operator_Interface_ACC,Target_Selection_ACC
  SoftECU_Brake : BusSelector  OutputSignals=DesiredBrakePressure
  SoftECU_Engine : BusSelector  OutputSignals=TorqueIntervention_Fast,TorqueIntervention_Slow,IdleSpeedControl,EngineOperation
  SoftECU_PowerSteering : BusSelector  OutputSignals=Trq_PowerSteering[Nm]
  SoftECU_StartButton : BusSelector  OutputSignals=Flag_NotPressed_Pedal[0|1],Lock[0|1],Sw_Acc[0|1],Sw_Ignition[0|1],Sw_StarterReq[0|1],State_StartButton[-2|-1|0|1|2|3]
  SoftECU_Transmission : BusSelector  OutputSignals=Lockup_Clutch_Control,Shift_Lock_Control,Shift_Strategy,Tip_Shift_Control,Torque_Intervention_Control
  Spring_Left : BusSelector  OutputSignals=Displ_Spring_FL[m],Displ_Spring_FL_dq1_Front[],Displ_Spring_FL_dq2_Front[]
  Spring_Left1 : BusSelector  OutputSignals=Displ_Spring_RL[m],Displ_Spring_RL_dq1_Rear[],Displ_Spring_RL_dq2_Rear[]
  Spring_Right : BusSelector  OutputSignals=Displ_Spring_FR[m],Displ_Spring_FR_dq1_Front[],Displ_Spring_FR_dq2_Front[]
  Spring_Right1 : BusSelector  OutputSignals=Displ_Spring_RR[m],Displ_Spring_RR_dq1_Rear[],Displ_Spring_RR_dq2_Rear[]
  Stabilizer : BusSelector  OutputSignals=Displ_Stabilizer[m],Displ_Stabilizer_FL[m],Displ_Stabilizer_FR[m],Displ_Stabilizer_dq1_Front[],Displ_Stabilizer_dq2_Front[]
  Stabilizer1 : BusSelector  OutputSignals=Displ_Stabilizer[m],Displ_Stabilizer_RL[m],Displ_Stabilizer_RR[m],Displ_Stabilizer_dq1_Rear[],Displ_Stabilizer_dq2_Rear[]
  StartButtonSignals : BusSelector  OutputSignals=Sw_StartButton[0Off|1On]
  Starter : BusSelector  OutputSignals=Trq_Starter[Nm],Inertia_Starter[kgm2]
  StatesSteeringSystem : BusSelector  OutputSignals=Angle_EPSSystem[deg],Angle_EPSSystem_dt[deg|s],Angle_LowerSteeringColumn[deg],Angle_LowerSteeringColumn_dt[deg|s],Angle_UpperSteeringColumn[deg],Angle_UpperSteeringColumn_dt[deg|s],Angle_SteeringWheel[deg],Angle_SteeringWheel_dt[deg|s],Displ_Steering[m],Displ_Steering_dt[m|s],Displ_SteeringRod_dt2[m|s2],Angle_SteeringGear[deg],Angle_SteeringGear_dt[deg|s],Angle_EPSPinion[rad],Angle_EPSPinion_dt[rad|s],i_Steering[rad|m],FrictionForce_SteeringRod[N],i_Steering_Wheel2Rod[rad|m]
  Steering : BusSelector  OutputSignals=Displ_Steering[m],Displ_Steering_dt[m|s],Displ_SteeringRod_dt2[m|s2],m_Steering[kg],ForcesAndTorques,GeneralizedForcesAndTorques,i_Steering[rad|m],i_Steering_Mean[],Angle_SteeringGear[deg],Angle_SteeringWheel[deg],Angle_SteeringGear_dt[deg|s],Angle_SteeringWheel_dt[deg|s],Const_Stiffness_SteeringColumn[Nm|rad],StatesSteeringSystem,FrictionTrq_SteeringSystem[Nm],SteeringWheelTorque
  SteeringWheelTorque : BusSelector  OutputSignals=TrqSensor_Steering[Nm],Trq_Driver[Nm],g_torque_SteeringWheel[Nm],TrqFriction_SteeringWheel[Nm],Trq_SteeringWheel[Nm]
  Suspension : BusSelector  OutputSignals=SuspensionFront,SuspensionRear
  SuspensionComplianceFront : BusSelector  OutputSignals=Angle_Comp_FR_Wheel_dt[x;y;z][m],Angle_Comp_FL_Wheel_dt[x;y;z][m],Angle_Comp_FR_Wheel[x;y;z][rad],Angle_Comp_FL_Wheel[x;y;z][rad],Displ_Comp_FR_Wheel_dt[x;y;z][m],Displ_Comp_FL_Wheel_dt[x;y;z][m],Displ_Comp_FR_Wheel[x;y;z][m],Displ_Comp_FL_Wheel[x;y;z][m],ComplianceLongForce,ComplianceLatForce,ComplianceAligningTorque,ComplianceLongTorque
  SuspensionComplianceRear : BusSelector  OutputSignals=Angle_Comp_RR_Wheel_dt[x;y;z][m],Angle_Comp_RL_Wheel_dt[x;y;z][m],Angle_Comp_RR_Wheel[x;y;z][rad],Angle_Comp_RL_Wheel[x;y;z][rad],Displ_Comp_RR_Wheel_dt[x;y;z][m],Displ_Comp_RL_Wheel_dt[x;y;z][m],Displ_Comp_RR_Wheel[x;y;z][m],Displ_Comp_RL_Wheel[x;y;z][m],ComplianceLongForce,ComplianceLatForce,ComplianceAligningTorque,ComplianceLongTorque
  SuspensionForcesFront : BusSelector  OutputSignals=F_FL_Spring[N],F_FL_Spring_dDispl_FL_Spring[N|m],F_FL_Damper[N],F_FL_Damper_dDispl_FL_Damper_dt[N|(m|s)],F_Stabilizer[N],F_Stabilizer_dDispl_Stabilizer[N|m],F_FR_Spring[N],F_FR_Spring_dDispl_FR_Spring[N|m],F_FR_Damper[N],F_FR_Damper_dDispl_FR_Damper_dt[N|(m|s)]
  SuspensionForcesRear : BusSelector  OutputSignals=F_RL_Spring[N],F_RL_Spring_dDispl_RL_Spring[N|m],F_RL_Damper[N],F_RL_Damper_dDispl_RL_Damper_dt[N|(m|s)],F_Stabilizer[N],F_Stabilizer_dDispl_Stabilizer[N|m],F_RR_Spring[N],F_RR_Spring_dDispl_RR_Spring[N|m],F_RR_Damper[N],F_RR_Damper_dDispl_RR_Damper_dt[N|(m|s)]
  SuspensionFront : BusSelector  OutputSignals=SuspensionKinematicsFront,SuspensionComplianceFront,SuspensionForcesFront,RelativePositionFront
  SuspensionKinematicsFront : BusSelector  OutputSignals=Kinematics_Left,Kinematics_Right,Stabilizer,SusKinFrontModel[]
  SuspensionKinematicsRear : BusSelector  OutputSignals=Kinematics_Left,Kinematics_Right,Stabilizer,SusKinRearModel[]
  SuspensionRear : BusSelector  OutputSignals=SuspensionKinematicsRear,SuspensionComplianceRear,SuspensionForcesRear,RelativePositionRear
  Target_Selection_ACC : BusSelector  OutputSignals=Target_Detected[0|1],Dist_Long[m],v_Rel[m|s],InLaneCheck[0|1],LaneCrossingCheck[0|1],v_Rel_Road[m|s],s_Fellows_Near[m]
  Terminator : Terminator
  TestBench : BusSelector  OutputSignals=Trq_TestBench[Nm],Inertia_TestBench[kgm2]
  Tip_Shift_Control : BusSelector  OutputSignals=Gear_Requested[]
  Tire : BusSelector  OutputSignals=Tire_FL,Tire_FR,Tire_RL,Tire_RR,TireModelSwitch
  TireForcesAndTorques : BusSelector  OutputSignals=F_FL_Tire_CoorSys_V[x;y;z][N],Trq_FL_Tire_CoorSys_V[x;y;z][Nm]
  TireForcesAndTorques1 : BusSelector  OutputSignals=F_FR_Tire_CoorSys_V[x;y;z][N],Trq_FR_Tire_CoorSys_V[x;y;z][Nm]
  TireForcesAndTorques2 : BusSelector  OutputSignals=F_RL_Tire_CoorSys_V[x;y;z][N],Trq_RL_Tire_CoorSys_V[x;y;z][Nm]
  TireForcesAndTorques3 : BusSelector  OutputSignals=F_RR_Tire_CoorSys_V[x;y;z][N],Trq_RR_Tire_CoorSys_V[x;y;z][Nm]
  TireModelSwitch : BusSelector  OutputSignals=Sw_Tire_Model[1TMEasy|2MF]
  TireWheelTorques : BusSelector  OutputSignals=Trq_Tire_Whee_FL[Nm],Trq_Tire_Whee_FR[Nm],Trq_Tire_Whee_RL[Nm],Trq_Tire_Whee_RR[Nm]
  Tire_FL : BusSelector  OutputSignals=ContactPoint,TireForcesAndTorques,ActiveTire
  Tire_FR : BusSelector  OutputSignals=ContactPoint,TireForcesAndTorques,ActiveTire
  Tire_RL : BusSelector  OutputSignals=ContactPoint,TireForcesAndTorques,ActiveTire
  Tire_RR : BusSelector  OutputSignals=ContactPoint,TireForcesAndTorques,ActiveTire
  Torque : BusSelector  OutputSignals=Trq_FL_Brake[Nm],Trq_FR_Brake[Nm],Trq_RL_Brake[Nm],Trq_RR_Brake[Nm]
  TorqueConverter : BusSelector  OutputSignals=Trq_Pump[Nm],Trq_Turbine[Nm]
  TorqueIntervention_Fast : BusSelector  OutputSignals=Enable_Trq_Intervention_Fast[0|1],Trq_Request_Fast[Nm],Engine_Dynamic_Fast[0|1]
  TorqueIntervention_Slow : BusSelector  OutputSignals=Enable_Trq_Intervention_Fast[0|1],Trq_Request_Fast[Nm],Enable_TrqDecrease_ESP[0|1],Trq_DecreaseRequest_ESP[Nm],Enable_TrqDecrease_Extern[0|1],Trq_DecreaseRequest_Extern[Nm],Pos_AccPedal[%],Pos_AccPedal_Request_Fast_ESP[%],Pos_AccPedal_Request_Slow_ESP[%],Pos_AccPedal_Request_Extern[%],Pos_AccPedal_Influenced[%]
  Torque_Intervention_Control : BusSelector  OutputSignals=Gear[],Factor_Trq_Engine_Red[%]
  Torques : BusSelector  OutputSignals=Trq_x_Aero_CoorSys_V[Nm],Trq_y_Aero_CoorSys_V[Nm],Trq_z_Aero_CoorSys_V[Nm]
  Traffic : BusSelector  OutputSignals=FellowMovement,ObjectParameters,Sensors
  TrafficObjects : BusSelector  OutputSignals=TrafficObjectsState[],Data_Valid[]
  TrafficScheduler : BusSelector  OutputSignals=s_Fellows_Ref_Scheduler[m],v_Fellows_Ref_Scheduler[km|h],Angle_Yaw_Fellows_Ref_Scheduler[deg],d_Fellows_Ref_Scheduler[m],LaneIdx_Fellows_Ref_Scheduler[],ForceToRoad_Fellows_Ref_Scheduler[0|1],v_Lat_Fellows_Ref_Scheduler[m|s],Flag_FellowsUsed[0|1],Direction_Fellows_Ref_Scheduler[-1|1],Flag_FellowsMode[0vel|1pos],Dist_Def_Trf[],Route_Id_Fellows_Ref_Scheduler[],UserSignals[],UserSignals_Fellows[],Info,Dist_Refline_Response[m]
  TrafficSign_Sensor_Dyn : BusSelector  OutputSignals=Sensor_Front_1
  TransferGearbox : BusSelector  OutputSignals=Trq_In_Transfer_Gearbox[Nm],omega_Out_Transfer_Gearbox[rad|s]
  Transmission : BusSelector  OutputSignals=ActiveTransmission,ManualTransmission,AutomaticTransmission
  Trq_FL_Tire_CoorSys_V[x;y;z][Nm] : BusSelector  OutputSignals=Trq_x_FL_Tire_CoorSys_V[Nm],Trq_y_FL_Tire_CoorSys_V[Nm],Trq_z_FL_Tire_CoorSys_V[Nm]
  Trq_FR_Tire_CoorSys_V[x;y;z][Nm] : BusSelector  OutputSignals=Trq_x_FR_Tire_CoorSys_V[Nm],Trq_y_FR_Tire_CoorSys_V[Nm],Trq_z_FR_Tire_CoorSys_V[Nm]
  Trq_RL_Tire_CoorSys_V[x;y;z][Nm] : BusSelector  OutputSignals=Trq_x_RL_Tire_CoorSys_V[Nm],Trq_y_RL_Tire_CoorSys_V[Nm],Trq_z_RL_Tire_CoorSys_V[Nm]
  Trq_RR_Tire_CoorSys_V[x;y;z][Nm] : BusSelector  OutputSignals=Trq_x_RR_Tire_CoorSys_V[Nm],Trq_y_RR_Tire_CoorSys_V[Nm],Trq_z_RR_Tire_CoorSys_V[Nm]
  UnitVec_y_Wheel_CoorSys_V[FL;FR][x;y;z] : BusSelector  OutputSignals=UnitVec_y_FL_Wheel_CoorSys_V[x;y;z],UnitVec_y_FR_Wheel_CoorSys_V[x;y;z]
  UnitVec_y_Wheel_CoorSys_V[RL;RR][x;y;z] : BusSelector  OutputSignals=UnitVec_y_RL_Wheel_CoorSys_V[x;y;z],UnitVec_y_RR_Wheel_CoorSys_V[x;y;z]
  UserSignals : BusSelector  OutputSignals=User1[],User2[],User3[],User4[],User5[],User6[],User7[],User8[],User9[],User10[]
  UserSignals1 : BusSelector  OutputSignals=User1[],User2[],User3[],User4[],User5[],User6[],User7[],User8[],User9[],User10[],User11[],User12[],User13[],User14[],User15[],User16[],User17[],User18[],User19[],User20[],User21[],User22[],User23[],User24[],User25[],User26[],User27[],User28[],User29[],User30[]
  UserSignals_Customized : BusSelector  OutputSignals=GPS_Method[],Const_Offset_Lat[deg],Const_Offset_Long[deg]
  UserSignals_Customized1 : BusSelector  OutputSignals=ExternalSegmentEnd_Mode[],ExternalSegmentEnd_Value[],ASM_Vehicle_TurnLights[],ECU_Commands[],Mnv_DataStream_5[],Mnv_DataStream_6[],Mnv_DataStream_7[],Mnv_DataStream_8[]
  UserSignals_Customized2 : BusSelector  OutputSignals=ManeuverSegmentEndTrigger[0|1],Fellow1_TurnLights,Fellow2_TurnLights,Fellow3_TurnLights,Fellow4_TurnLights,Fellow5_TurnLights,Fellow6_TurnLights,Fellow7_TurnLights,Fellow8_TurnLights,Fellow9_TurnLights,Fellow10_TurnLights,Fellow11_TurnLights,Fellow12_TurnLights,Fellow13_TurnLights,Fellow14_TurnLights,Fellow15_TurnLights
  VacuumChamber : BusSelector  OutputSignals=m_dot_In_1_VacuumChamber[kg|s],m_dot_In_2_VacuumChamber[kg|s],m_dot_Out_2_VacuumChamber[kg|s],T_VacuumChamber[degC],p_VacuumChamber[bar],V_VacuumChamber[m3]
  Vehicle : BusSelector  OutputSignals=Linear,Angular
  Vehicle1 : BusSelector  OutputSignals=Linear,Angular
  VehicleCoG : BusSelector  OutputSignals=Linear,Angular
  VehicleDynamics : BusSelector  OutputSignals=VehicleMovement,Tire,Aerodynamics,Wheel,Steering,Brake,Suspension
  VehicleEquationOfMotion : BusSelector  OutputSignals=GeneralizedForcesAndTorques,GeneralizedVelocitiesDerivative
  VehicleMassAndAdditionalLoads : BusSelector  OutputSignals=m_TotalVehicle[kg],PosVec_CoG_TotalVehicle[x;y;z][m],Inertia_Tensor_TotalVehicle[3x3][kgm2],m_TotalV1[kg],PosVec_CoG_TotalV1[x;y;z][m],Inertia_Tensor_TotalV1[3x3][kgm2]
  VehicleMovement : BusSelector  OutputSignals=Accelerations,Velocities,Positions,VehicleEquationOfMotion,GravityAcceleration,SensorMotion,VehicleMassAndAdditionalLoads,MassForcesAndTorques
  Velocities : BusSelector  OutputSignals=Vehicle,Wheels,Generalized
  Wheel : BusSelector  OutputSignals=WheelSpeed_CoorSys_V,ShaftsTorques_CoorSys_V,TireWheelTorques,WheelSpeed,RotationAngle
  WheelAngularVelocity : BusSelector  OutputSignals=w_FL_Abs_Wheel[x;y;z][rad|s],w_FR_Abs_Wheel[x;y;z][rad|s],w_RL_Abs_Wheel[x;y;z][rad|s],w_RR_Abs_Wheel[x;y;z][rad|s]
  WheelBodyAngularVelocity : BusSelector  OutputSignals=w_FL_Abs_WheelBody[x;y;z][rad|s],w_FR_Abs_WheelBody[x;y;z][rad|s],w_RL_Abs_WheelBody[x;y;z][rad|s],w_RR_Abs_WheelBody[x;y;z][rad|s]
  WheelBodyVelocity : BusSelector  OutputSignals=v_FL_Abs_WheelBody[x;y;z][km|h],v_FR_Abs_WheelBody[x;y;z][km|h],v_RL_Abs_WheelBody[x;y;z][km|h],v_RR_Abs_WheelBody[x;y;z][km|h]
  WheelSpeed : BusSelector  OutputSignals=omega_FL_Wheel[rad|s],omega_FR_Wheel[rad|s],omega_RL_Wheel[rad|s],omega_RR_Wheel[rad|s]
  WheelSpeed_CoorSys_V : BusSelector  OutputSignals=w_Wheel_FL_CoorSys_V[x;y;z][rad|s],w_Wheel_FR_CoorSys_V[x;y;z][rad|s],w_Wheel_RL_CoorSys_V[x;y;z][rad|s],w_Wheel_RR_CoorSys_V[x;y;z][rad|s]
  Wheels : BusSelector  OutputSignals=Linear
  Wheels1 : BusSelector  OutputSignals=Linear,Angular
  Wheels2 : BusSelector  OutputSignals=Linear
  a_Vehicle_CoG[x;y;z][m|s2] : BusSelector  OutputSignals=a_x_Vehicle_CoG[m|s2],a_y_Vehicle_CoG[m|s2],a_z_Vehicle_CoG[m|s2]
  v_Vehicle[x;y;z][km|h] : BusSelector  OutputSignals=v_x_Vehicle[km|h],v_y_Vehicle[km|h],v_z_Vehicle[km|h]
  v_Vehicle_CoG[x;y;z][km|h] : BusSelector  OutputSignals=v_x_Vehicle_CoG[km|h],v_y_Vehicle_CoG[km|h],v_z_Vehicle_CoG[km|h]
  w_Vehicle[x;y;z][deg|s] : BusSelector  OutputSignals=RollRate_Vehicle[deg|s],PitchRate_Vehicle[deg|s],YawRate_Vehicle[deg|s]
  w_Vehicle_CoG[x;y;z][deg|s] : BusSelector  OutputSignals=RollRate_Vehicle_CoG[deg|s],PitchRate_Vehicle_CoG[deg|s],YawRate_Vehicle_CoG[deg|s]
  w_Vehicle_CoG_dt[x;y;z][rad|s2] : BusSelector  OutputSignals=w_x_Vehicle_CoG_dt[rad|s2],w_y_Vehicle_CoG_dt[rad|s2],w_z_Vehicle_CoG_dt[rad|s2]
  z_Wheel_dt[FL;FR;RL;RR][m|s] : BusSelector  OutputSignals=z_FL_Wheel_dt[m|s],z_FR_Wheel_dt[m|s],z_RL_Wheel_dt[m|s],z_RR_Wheel_dt[m|s]
  wires:
  ASMSignalBus/1 -> BusSelector_1/1
  BusSelector_1/1 -> SoftECU/1  "<SoftECU>"
  SoftECU/1 -> SoftECU_Engine/1  "<SoftECU_Engine>"
  SoftECU_Engine/1 -> TorqueIntervention_Fast/1  "<TorqueIntervention_Fast>"
  SoftECU_Engine/2 -> TorqueIntervention_Slow/1  "<TorqueIntervention_Slow>"
  SoftECU_Engine/3 -> IdleSpeedControl/1  "<IdleSpeedControl>"
  SoftECU_Engine/4 -> EngineOperation/1  "<EngineOperation>"
  SoftECU/2 -> SoftECU_Brake/1  "<SoftECU_Brake>"
  SoftECU_Brake/1 -> DesiredBrakePressure/1  "<DesiredBrakePressure>"
  SoftECU/3 -> SoftECU_ACC/1  "<SoftECU_ACC>"
  SoftECU_ACC/1 -> Controller_ACC/1  "<Controller_ACC>"
  SoftECU_ACC/2 -> Interface_ACC/1  "<Interface_ACC>"
  SoftECU_ACC/3 -> Operator_Interface_ACC/1  "<Operator_Interface_ACC>"
  SoftECU_ACC/4 -> Target_Selection_ACC/1  "<Target_Selection_ACC>"
  SoftECU/4 -> SoftECU_Transmission/1  "<SoftECU_Transmission>"
  SoftECU_Transmission/1 -> Lockup_Clutch_Control/1  "<Lockup_Clutch_Control>"
  SoftECU_Transmission/2 -> Shift_Lock_Control/1  "<Shift_Lock_Control>"
  SoftECU_Transmission/3 -> Shift_Strategy/1  "<Shift_Strategy>"
  SoftECU_Transmission/4 -> Tip_Shift_Control/1  "<Tip_Shift_Control>"
  SoftECU_Transmission/5 -> Torque_Intervention_Control/1  "<Torque_Intervention_Control>"
  SoftECU/5 -> SoftECU_PowerSteering/1  "<SoftECU_PowerSteering>"
  SoftECU/6 -> SoftECU_StartButton/1  "<SoftECU_StartButton>"
  BusSelector_1/2 -> VehicleDynamics/1  "<VehicleDynamics>"
  VehicleDynamics/1 -> VehicleMovement/1  "<VehicleMovement>"
  VehicleMovement/1 -> Accelerations/1  "<Accelerations>"
  Accelerations/1 -> VehicleCoG/1  "<VehicleCoG>"
  VehicleCoG/1 -> Linear/1  "<Linear>"
  Linear/1 -> a_Vehicle_CoG[x;y;z][m|s2]/1  "<a_Vehicle_CoG[x;y;z][m|s2]>"
  VehicleCoG/2 -> Angular/1  "<Angular>"
  Angular/1 -> w_Vehicle_CoG_dt[x;y;z][rad|s2]/1  "<w_Vehicle_CoG_dt[x;y;z][rad|s2]>"
  Accelerations/2 -> Wheels/1  "<Wheels>"
  Wheels/1 -> Linear1/1  "<Linear>"
  VehicleMovement/2 -> Velocities/1  "<Velocities>"
  Velocities/1 -> Vehicle/1  "<Vehicle>"
  Vehicle/1 -> Linear2/1  "<Linear>"
  Linear2/1 -> v_Vehicle_CoG[x;y;z][km|h]/1  "<v_Vehicle_CoG[x;y;z][km|h]>"
  Vehicle/2 -> Angular1/1  "<Angular>"
  Angular1/1 -> w_Vehicle_CoG[x;y;z][deg|s]/1  "<w_Vehicle_CoG[x;y;z][deg|s]>"
  Velocities/2 -> Wheels1/1  "<Wheels>"
  Wheels1/1 -> Linear3/1  "<Linear>"
  Linear3/1 -> WheelBodyVelocity/1  "<WheelBodyVelocity>"
  Wheels1/2 -> Angular2/1  "<Angular>"
  Angular2/1 -> WheelBodyAngularVelocity/1  "<WheelBodyAngularVelocity>"
  Angular2/2 -> WheelAngularVelocity/1  "<WheelAngularVelocity>"
  Velocities/3 -> Generalized/1  "<Generalized>"
  Generalized/1 -> v_Vehicle[x;y;z][km|h]/1  "<v_Vehicle[x;y;z][km|h]>"
  Generalized/2 -> w_Vehicle[x;y;z][deg|s]/1  "<w_Vehicle[x;y;z][deg|s]>"
  Generalized/3 -> z_Wheel_dt[FL;FR;RL;RR][m|s]/1  "<z_Wheel_dt[FL;FR;RL;RR][m|s]>"
  VehicleMovement/3 -> Positions/1  "<Positions>"
  Positions/1 -> Vehicle1/1  "<Vehicle>"
  Vehicle1/1 -> Linear4/1  "<Linear>"
  Linear4/1 -> Pos_Vehicle_CoorSys_E[x;y;z][m]/1  "<Pos_Vehicle_CoorSys_E[x;y;z][m]>"
  Vehicle1/2 -> Angular3/1  "<Angular>"
  Angular3/1 -> Angle_Vehicle_CoorSys_E[x;y;z][deg]/1  "<Angle_Vehicle_CoorSys_E[x;y;z][deg]>"
  Positions/2 -> Wheels2/1  "<Wheels>"
  Wheels2/1 -> Linear5/1  "<Linear>"
  VehicleMovement/4 -> VehicleEquationOfMotion/1  "<VehicleEquationOfMotion>"
  VehicleEquationOfMotion/1 -> GeneralizedForcesAndTorques/1  "<GeneralizedForcesAndTorques>"
  VehicleEquationOfMotion/2 -> GeneralizedVelocitiesDerivative/1  "<GeneralizedVelocitiesDerivative>"
  VehicleMovement/5 -> GravityAcceleration/1  "<GravityAcceleration>"
  VehicleMovement/6 -> SensorMotion/1  "<SensorMotion>"
  SensorMotion/1 -> Sensor1/1  "<Sensor1>"
  SensorMotion/2 -> Sensor2/1  "<Sensor2>"
  SensorMotion/3 -> Sensor3/1  "<Sensor3>"
  SensorMotion/4 -> Sensor4/1  "<Sensor4>"
  VehicleMovement/7 -> VehicleMassAndAdditionalLoads/1  "<VehicleMassAndAdditionalLoads>"
  VehicleMovement/8 -> MassForcesAndTorques/1  "<MassForcesAndTorques>"
  MassForcesAndTorques/1 -> GravitationalForces/1  "<GravitationalForces>"
  MassForcesAndTorques/2 -> GyroscopicForces/1  "<GyroscopicForces>"
  MassForcesAndTorques/3 -> GyroscopicTorques/1  "<GyroscopicTorques>"
  MassForcesAndTorques/4 -> ResidualAccelerations/1  "<ResidualAccelerations>"
  VehicleDynamics/2 -> Tire/1  "<Tire>"
  Tire/1 -> Tire_FL/1  "<Tire_FL>"
  Tire_FL/1 -> ContactPoint/1  "<ContactPoint>"
  Tire_FL/2 -> TireForcesAndTorques/1  "<TireForcesAndTorques>"
  TireForcesAndTorques/1 -> F_FL_Tire_CoorSys_V[x;y;z][N]/1  "<F_FL_Tire_CoorSys_V[x;y;z][N]>"
  TireForcesAndTorques/2 -> Trq_FL_Tire_CoorSys_V[x;y;z][Nm]/1  "<Trq_FL_Tire_CoorSys_V[x;y;z][Nm]>"
  Tire_FL/3 -> ActiveTire/1  "<ActiveTire>"
  Tire/2 -> Tire_FR/1  "<Tire_FR>"
  Tire_FR/1 -> ContactPoint1/1  "<ContactPoint>"
  Tire_FR/2 -> TireForcesAndTorques1/1  "<TireForcesAndTorques>"
  TireForcesAndTorques1/1 -> F_FR_Tire_CoorSys_V[x;y;z][N]/1  "<F_FR_Tire_CoorSys_V[x;y;z][N]>"
  TireForcesAndTorques1/2 -> Trq_FR_Tire_CoorSys_V[x;y;z][Nm]/1  "<Trq_FR_Tire_CoorSys_V[x;y;z][Nm]>"
  Tire_FR/3 -> ActiveTire1/1  "<ActiveTire>"
  Tire/3 -> Tire_RL/1  "<Tire_RL>"
  Tire_RL/1 -> ContactPoint2/1  "<ContactPoint>"
  Tire_RL/2 -> TireForcesAndTorques2/1  "<TireForcesAndTorques>"
  TireForcesAndTorques2/1 -> F_RL_Tire_CoorSys_V[x;y;z][N]/1  "<F_RL_Tire_CoorSys_V[x;y;z][N]>"
  TireForcesAndTorques2/2 -> Trq_RL_Tire_CoorSys_V[x;y;z][Nm]/1  "<Trq_RL_Tire_CoorSys_V[x;y;z][Nm]>"
  Tire_RL/3 -> ActiveTire2/1  "<ActiveTire>"
  Tire/4 -> Tire_RR/1  "<Tire_RR>"
  Tire_RR/1 -> ContactPoint3/1  "<ContactPoint>"
  Tire_RR/2 -> TireForcesAndTorques3/1  "<TireForcesAndTorques>"
  TireForcesAndTorques3/1 -> F_RR_Tire_CoorSys_V[x;y;z][N]/1  "<F_RR_Tire_CoorSys_V[x;y;z][N]>"
  TireForcesAndTorques3/2 -> Trq_RR_Tire_CoorSys_V[x;y;z][Nm]/1  "<Trq_RR_Tire_CoorSys_V[x;y;z][Nm]>"
  Tire_RR/3 -> ActiveTire3/1  "<ActiveTire>"
  Tire/5 -> TireModelSwitch/1  "<TireModelSwitch>"
  VehicleDynamics/3 -> Aerodynamics/1  "<Aerodynamics>"
  Aerodynamics/1 -> Forces/1  "<Forces>"
  Aerodynamics/2 -> Torques/1  "<Torques>"
  Aerodynamics/3 -> Coefficients/1  "<Coefficients>"
  VehicleDynamics/4 -> Wheel/1  "<Wheel>"
  Wheel/1 -> WheelSpeed_CoorSys_V/1  "<WheelSpeed_CoorSys_V>"
  Wheel/2 -> ShaftsTorques_CoorSys_V/1  "<ShaftsTorques_CoorSys_V>"
  Wheel/3 -> TireWheelTorques/1  "<TireWheelTorques>"
  Wheel/4 -> WheelSpeed/1  "<WheelSpeed>"
  Wheel/5 -> RotationAngle/1  "<RotationAngle>"
  VehicleDynamics/5 -> Steering/1  "<Steering>"
  Steering/5 -> ForcesAndTorques/1  "<ForcesAndTorques>"
  Steering/6 -> GeneralizedForcesAndTorques1/1  "<GeneralizedForcesAndTorques>"
  Steering/14 -> StatesSteeringSystem/1  "<StatesSteeringSystem>"
  Steering/16 -> SteeringWheelTorque/1  "<SteeringWheelTorque>"
  VehicleDynamics/6 -> Brake/1  "<Brake>"
  Brake/1 -> MasterBrakeCylinder/1  "<MasterBrakeCylinder>"
  MasterBrakeCylinder/1 -> ActiveBrakeCylinder/1  "<ActiveBrakeCylinder>"
  MasterBrakeCylinder/2 -> BrakeCylinderLinear/1  "<BrakeCylinderLinear>"
  MasterBrakeCylinder/3 -> BrakeCylinderPhysical/1  "<BrakeCylinderPhysical>"
  Brake/2 -> BrakeHydraulics/1  "<BrakeHydraulics>"
  BrakeHydraulics/1 -> BrakingCircuit/1  "<BrakingCircuit>"
  BrakingCircuit/1 -> Pressure/1  "<Pressure>"
  Brake/3 -> BrakeDisc/1  "<BrakeDisc>"
  BrakeDisc/1 -> Torque/1  "<Torque>"
  BrakeDisc/2 -> MaximumTorque/1  "<MaximumTorque>"
  BrakeDisc/3 -> Pressure1/1  "<Pressure>"
  BrakeDisc/4 -> Const_BrakeDiscFactor/1  "<Const_BrakeDiscFactor>"
  Brake/4 -> BrakeBooster/1  "<BrakeBooster>"
  BrakeBooster/1 -> ManifoldValve/1  "<ManifoldValve>"
  BrakeBooster/2 -> VacuumChamber/1  "<VacuumChamber>"
  BrakeBooster/3 -> BellValve/1  "<BellValve>"
  BrakeBooster/4 -> RearChamber/1  "<RearChamber>"
  BrakeBooster/5 -> PushRod/1  "<PushRod>"
  PushRod/9 -> OutputPoint/1  "<OutputPoint>"
  BrakeBooster/6 -> ControllerBellValve/1  "<ControllerBellValve>"
  Brake/5 -> Manifold/1  "<Manifold>"
  VehicleDynamics/7 -> Suspension/1  "<Suspension>"
  Suspension/1 -> SuspensionFront/1  "<SuspensionFront>"
  SuspensionFront/1 -> SuspensionKinematicsFront/1  "<SuspensionKinematicsFront>"
  SuspensionKinematicsFront/1 -> Kinematics_Left/1  "<Kinematics_Left>"
  Kinematics_Left/1 -> Position_Left/1  "<Position_Left>"
  Kinematics_Left/2 -> Orientation_Left/1  "<Orientation_Left>"
  Orientation_Left/1 -> Angle_FL_Wheel[Alpha;Beta;Gamma][deg]/1  "<Angle_FL_Wheel[Alpha;Beta;Gamma][deg]>"
  Kinematics_Left/3 -> Spring_Left/1  "<Spring_Left>"
  Kinematics_Left/4 -> Damper_Left/1  "<Damper_Left>"
  SuspensionKinematicsFront/2 -> Kinematics_Right/1  "<Kinematics_Right>"
  Kinematics_Right/1 -> Position_Right/1  "<Position_Right>"
  Kinematics_Right/2 -> Orientation_Right/1  "<Orientation_Right>"
  Orientation_Right/1 -> Angle_FR_Wheel[Alpha;Beta;Gamma][deg]/1  "<Angle_FR_Wheel[Alpha;Beta;Gamma][deg]>"
  Kinematics_Right/3 -> Spring_Right/1  "<Spring_Right>"
  Kinematics_Right/4 -> Damper_Right/1  "<Damper_Right>"
  SuspensionKinematicsFront/3 -> Stabilizer/1  "<Stabilizer>"
  SuspensionFront/2 -> SuspensionComplianceFront/1  "<SuspensionComplianceFront>"
  SuspensionComplianceFront/9 -> ComplianceLongForce/1  "<ComplianceLongForce>"
  SuspensionComplianceFront/10 -> ComplianceLatForce/1  "<ComplianceLatForce>"
  SuspensionComplianceFront/11 -> ComplianceAligningTorque/1  "<ComplianceAligningTorque>"
  SuspensionComplianceFront/12 -> ComplianceLongTorque/1  "<ComplianceLongTorque>"
  SuspensionFront/3 -> SuspensionForcesFront/1  "<SuspensionForcesFront>"
  SuspensionFront/4 -> RelativePositionFront/1  "<RelativePositionFront>"
  RelativePositionFront/1 -> Pos_Wheel[FL;FR][x;y;z][m]/1  "<Pos_Wheel[FL;FR][x;y;z][m]>"
  RelativePositionFront/2 -> UnitVec_y_Wheel_CoorSys_V[FL;FR][x;y;z]/1  "<UnitVec_y_Wheel_CoorSys_V[FL;FR][x;y;z]>"
  RelativePositionFront/3 -> Angle_Wheel[FL;FR][Toe;Camber][deg]/1  "<Angle_Wheel[FL;FR][Toe;Camber][deg]>"
  Angle_Wheel[FL;FR][Toe;Camber][deg]/1 -> Angle_FL_Wheel[Toe;Camber][deg]/1  "<Angle_FL_Wheel[Toe;Camber][deg]>"
  Angle_Wheel[FL;FR][Toe;Camber][deg]/2 -> Angle_FR_Wheel[Toe;Camber][deg]/1  "<Angle_FR_Wheel[Toe;Camber][deg]>"
  Suspension/2 -> SuspensionRear/1  "<SuspensionRear>"
  SuspensionRear/1 -> SuspensionKinematicsRear/1  "<SuspensionKinematicsRear>"
  SuspensionKinematicsRear/1 -> Kinematics_Left1/1  "<Kinematics_Left>"
  Kinematics_Left1/1 -> Position_Left1/1  "<Position_Left>"
  Kinematics_Left1/2 -> Orientation_Left1/1  "<Orientation_Left>"
  Orientation_Left1/1 -> Angle_RL_Wheel[Alpha;Beta;Gamma][deg]/1  "<Angle_RL_Wheel[Alpha;Beta;Gamma][deg]>"
  Kinematics_Left1/3 -> Spring_Left1/1  "<Spring_Left>"
  Kinematics_Left1/4 -> Damper_Left1/1  "<Damper_Left>"
  SuspensionKinematicsRear/2 -> Kinematics_Right1/1  "<Kinematics_Right>"
  Kinematics_Right1/1 -> Position_Right1/1  "<Position_Right>"
  Kinematics_Right1/2 -> Orientation_Right1/1  "<Orientation_Right>"
  Orientation_Right1/1 -> Angle_RR_Wheel[Alpha;Beta;Gamma][deg]/1  "<Angle_RR_Wheel[Alpha;Beta;Gamma][deg]>"
  Kinematics_Right1/3 -> Spring_Right1/1  "<Spring_Right>"
  Kinematics_Right1/4 -> Damper_Right1/1  "<Damper_Right>"
  SuspensionKinematicsRear/3 -> Stabilizer1/1  "<Stabilizer>"
  SuspensionRear/2 -> SuspensionComplianceRear/1  "<SuspensionComplianceRear>"
  SuspensionComplianceRear/9 -> ComplianceLongForce1/1  "<ComplianceLongForce>"
  SuspensionComplianceRear/10 -> ComplianceLatForce1/1  "<ComplianceLatForce>"
  SuspensionComplianceRear/11 -> ComplianceAligningTorque1/1  "<ComplianceAligningTorque>"
  SuspensionComplianceRear/12 -> ComplianceLongTorque1/1  "<ComplianceLongTorque>"
  SuspensionRear/3 -> SuspensionForcesRear/1  "<SuspensionForcesRear>"
  SuspensionRear/4 -> RelativePositionRear/1  "<RelativePositionRear>"
  RelativePositionRear/1 -> Pos_Wheel[RL;RR][x;y;z][m]/1  "<Pos_Wheel[RL;RR][x;y;z][m]>"
  RelativePositionRear/2 -> UnitVec_y_Wheel_CoorSys_V[RL;RR][x;y;z]/1  "<UnitVec_y_Wheel_CoorSys_V[RL;RR][x;y;z]>"
  RelativePositionRear/3 -> Angle_Wheel[RL;RR][Toe;Camber][deg]/1  "<Angle_Wheel[RL;RR][Toe;Camber][deg]>"
  Angle_Wheel[RL;RR][Toe;Camber][deg]/1 -> Angle_RL_Wheel[Toe;Camber][deg]/1  "<Angle_RL_Wheel[Toe;Camber][deg]>"
  Angle_Wheel[RL;RR][Toe;Camber][deg]/2 -> Angle_RR_Wheel[Toe;Camber][deg]/1  "<Angle_RR_Wheel[Toe;Camber][deg]>"
  BusSelector_1/3 -> BasicEngine/1  "<BasicEngine>"
  BasicEngine/1 -> EngineTorques/1  "<EngineTorques>"
  BasicEngine/2 -> FuelConsumption/1  "<FuelConsumption>"
  FuelConsumption/3 -> Efficiency/1  "<Efficiency>"
  FuelConsumption/4 -> CO2_Emission/1  "<CO2_Emission>"
  BusSelector_1/4 -> Drivetrain/1  "<Drivetrain>"
  Drivetrain/1 -> Transmission/1  "<Transmission>"
  Transmission/1 -> ActiveTransmission/1  "<ActiveTransmission>"
  Transmission/2 -> ManualTransmission/1  "<ManualTransmission>"
  ManualTransmission/1 -> Clutch/1  "<Clutch>"
  ManualTransmission/2 -> GearBox/1  "<GearBox>"
  Transmission/3 -> AutomaticTransmission/1  "<AutomaticTransmission>"
  AutomaticTransmission/1 -> LockUpClutch/1  "<LockUpClutch>"
  AutomaticTransmission/2 -> GearBox1/1  "<GearBox>"
  AutomaticTransmission/3 -> TorqueConverter/1  "<TorqueConverter>"
  Drivetrain/2 -> FinalDriveAssembly/1  "<FinalDriveAssembly>"
  FinalDriveAssembly/2 -> CentralDifferential/1  "<CentralDifferential>"
  FinalDriveAssembly/3 -> FrontDifferential/1  "<FrontDifferential>"
  FinalDriveAssembly/4 -> RearDifferential/1  "<RearDifferential>"
  FinalDriveAssembly/5 -> Shaft_TGCL4WD/1  "<Shaft_TGCL4WD>"
  FinalDriveAssembly/6 -> Shaft_CF/1  "<Shaft_CF>"
  FinalDriveAssembly/7 -> Shaft_CR/1  "<Shaft_CR>"
  FinalDriveAssembly/8 -> TransferGearbox/1  "<TransferGearbox>"
  FinalDriveAssembly/9 -> Clutch_4WD/1  "<Clutch_4WD>"
  FinalDriveAssembly/10 -> Shaft_FL/1  "<Shaft_FL>"
  FinalDriveAssembly/11 -> Shaft_FR/1  "<Shaft_FR>"
  FinalDriveAssembly/12 -> Shaft_RL/1  "<Shaft_RL>"
  FinalDriveAssembly/13 -> Shaft_RR/1  "<Shaft_RR>"
  Drivetrain/3 -> Crankshaft/1  "<Crankshaft>"
  Drivetrain/4 -> Starter/1  "<Starter>"
  Drivetrain/5 -> TestBench/1  "<TestBench>"
  BusSelector_1/5 -> Environment/1  "<Environment>"
  Environment/1 -> Driver/1  "<Driver>"
  Driver/1 -> OutputSignals/1  "<OutputSignals>"
  OutputSignals/7 -> AutomaticTrmCtrlSignals/1  "<AutomaticTrmCtrlSignals>"
  OutputSignals/8 -> StartButtonSignals/1  "<StartButtonSignals>"
  OutputSignals/9 -> ParkingBrakeSignals/1  "<ParkingBrakeSignals>"
  Driver/2 -> LongitudinalController/1  "<LongitudinalController>"
  LongitudinalController/1 -> LongCtrl/1  "<LongCtrl>"
  LongitudinalController/2 -> GearShifter/1  "<GearShifter>"
  Driver/3 -> ReferenceVelocity/1  "<ReferenceVelocity>"
  Driver/4 -> LateralController/1  "<LateralController>"
  LateralController/1 -> ActiveLateralController/1  "<ActiveLateralController>"
  LateralController/2 -> LatCtrl1/1  "<LatCtrl1>"
  LateralController/3 -> LatCtrl2/1  "<LatCtrl2>"
  LateralController/4 -> PositionError/1  "<PositionError>"
  Environment/2 -> Road/1  "<Road>"
  Road/1 -> Road_Init/1  "<Road_Init>"
  Road_Init/1 -> Pos_Vehicle_Init_CoorSys_E[x;y;z][m]/1  "<Pos_Vehicle_Init_CoorSys_E[x;y;z][m]>"
  Road_Init/2 -> Angle_Vehicle_Init_CoorSys_E[x;y;z][rad]/1  "<Angle_Vehicle_Init_CoorSys_E[x;y;z][rad]>"
  Road/2 -> Road_ASMVeh/1  "<Road_ASMVeh>"
  Road/3 -> Road_ContactPoints/1  "<Road_ContactPoints>"
  Road/4 -> Road_Preview/1  "<Road_Preview>"
  Road/5 -> Road_Info/1  "<Road_Info>"
  Road_Info/4 -> Dist_Response_Maneuver/1  "<Dist_Response_Maneuver>"
  Road/6 -> Road_TrafficFellows/1  "<Road_TrafficFellows>"
  Road_TrafficFellows/18 -> Dist_Response_Traffic/1  "<Dist_Response_Traffic>"
  Road/7 -> UserSignals/1  "<UserSignals>"
  Road/8 -> UserSignals_Customized/1  "<UserSignals_Customized>"
  Road/9 -> Pos_Vehicle_GPS[Long;Lat][deg]/1  "<Pos_Vehicle_GPS[Long;Lat][deg]>"
  Road/10 -> Ambient/1  "<Ambient>"
  Road/11 -> LaneSensor_Dynamic/1  "<LaneSensor_Dynamic>"
  LaneSensor_Dynamic/1 -> Parameters/1  "<Parameters>"
  LaneSensor_Dynamic/2 -> Sensor_Output/1  "<Sensor_Output>"
  Sensor_Output/1 -> SFunction_Info/1  "<SFunction_Info>"
  Sensor_Output/2 -> Network_Item/1  "<Network_Item>"
  Sensor_Output/3 -> CurrentLane/1  "<CurrentLane>"
  CurrentLane/1 -> Common/1  "<Common>"
  CurrentLane/2 -> LeftSide/1  "<LeftSide>"
  CurrentLane/3 -> RightSide/1  "<RightSide>"
  Sensor_Output/4 -> Lanes_Left/1  "<Lanes_Left>"
  Sensor_Output/5 -> Lanes_Right/1  "<Lanes_Right>"
  Sensor_Output/6 -> Measurement_Points/1  "<Measurement_Points>"
  Environment/3 -> Maneuver/1  "<Maneuver>"
  Maneuver/1 -> ManeuverScheduler/1  "<ManeuverScheduler>"
  ManeuverScheduler/1 -> MdlControl/1  "<MdlControl>"
  ManeuverScheduler/2 -> InitialVehStates/1  "<InitialVehStates>"
  ManeuverScheduler/3 -> ModeSignals/1  "<ModeSignals>"
  ManeuverScheduler/4 -> RefSignals/1  "<RefSignals>"
  ManeuverScheduler/5 -> Parameters1/1  "<Parameters>"
  ManeuverScheduler/6 -> UserSignals1/1  "<UserSignals>"
  ManeuverScheduler/7 -> Info/1  "<Info>"
  Maneuver/2 -> UserSignals_Customized1/1  "<UserSignals_Customized>"
  Environment/4 -> Traffic/1  "<Traffic>"
  Traffic/1 -> FellowMovement/1  "<FellowMovement>"
  FellowMovement/1 -> FellowMovement1/1  "<FellowMovement>"
  FellowMovement/2 -> FellowPositions/1  "<FellowPositions>"
  FellowPositions/1 -> Pos_Fellows_MainPnt_CoorSys_E[x;y;z][m]/1  "<Pos_Fellows_MainPnt_CoorSys_E[x;y;z][m]>"
  FellowPositions/2 -> Angle_Fellows[x;y;z][deg]/1  "<Angle_Fellows[x;y;z][deg]>"
  FellowMovement/3 -> FellowVelocities/1  "<FellowVelocities>"
  FellowMovement/4 -> TrafficScheduler/1  "<TrafficScheduler>"
  TrafficScheduler/15 -> Info1/1  "<Info>"
  FellowMovement/5 -> UserSignals_Customized2/1  "<UserSignals_Customized>"
  Traffic/2 -> ObjectParameters/1  "<ObjectParameters>"
  ObjectParameters/1 -> FellowsGeometry/1  "<FellowsGeometry>"
  FellowsGeometry/1 -> Info2/1  "<Info>"
  ObjectParameters/2 -> TrafficObjects/1  "<TrafficObjects>"
  ObjectParameters/3 -> DiscreteObjects/1  "<DiscreteObjects>"
  Traffic/3 -> Sensors/1  "<Sensors>"
  Sensors/1 -> Object_Sensor_3D/1  "<Object_Sensor_3D>"
  Object_Sensor_3D/1 -> Sample_Pulse/1  "<Sample_Pulse>"
  Object_Sensor_3D/2 -> Sensor_Scheduler/1  "<Sensor_Scheduler>"
  Object_Sensor_3D/3 -> Sensor_1_Front_Long/1  "<Sensor_1_Front_Long>"
  Sensor_1_Front_Long/1 -> Parameter/1  "<Parameter>"
  Sensor_1_Front_Long/2 -> SensorIndex/1  "<SensorIndex>"
  Sensor_1_Front_Long/3 -> Info3/1  "<Info>"
  Sensor_1_Front_Long/4 -> SensorOutput/1  "<SensorOutput>"
  Sensor_1_Front_Long/5 -> RadarEffects/1  "<RadarEffects>"
  Sensor_1_Front_Long/6 -> CustomPoints/1  "<CustomPoints>"
  Object_Sensor_3D/4 -> Sensor_2_Front_Mid/1  "<Sensor_2_Front_Mid>"
  Sensor_2_Front_Mid/1 -> Parameter1/1  "<Parameter>"
  Sensor_2_Front_Mid/2 -> SensorIndex1/1  "<SensorIndex>"
  Sensor_2_Front_Mid/3 -> Info4/1  "<Info>"
  Sensor_2_Front_Mid/4 -> SensorOutput1/1  "<SensorOutput>"
  Sensor_2_Front_Mid/5 -> RadarEffects1/1  "<RadarEffects>"
  Sensor_2_Front_Mid/6 -> CustomPoints1/1  "<CustomPoints>"
  Object_Sensor_3D/5 -> Sensor_3_Rear/1  "<Sensor_3_Rear>"
  Sensor_3_Rear/1 -> Parameter2/1  "<Parameter>"
  Sensor_3_Rear/2 -> SensorIndex2/1  "<SensorIndex>"
  Sensor_3_Rear/3 -> Info5/1  "<Info>"
  Sensor_3_Rear/4 -> SensorOutput2/1  "<SensorOutput>"
  Sensor_3_Rear/5 -> RadarEffects2/1  "<RadarEffects>"
  Sensor_3_Rear/6 -> CustomPoints2/1  "<CustomPoints>"
  Sensors/2 -> Object_Sensor_2D/1  "<Object_Sensor_2D>"
  Object_Sensor_2D/1 -> Sample_Pulse1/1  "<Sample_Pulse>"
  Object_Sensor_2D/2 -> Sensor_Scheduler1/1  "<Sensor_Scheduler>"
  Object_Sensor_2D/3 -> Sensor_1_Front/1  "<Sensor_1_Front>"
  Sensor_1_Front/1 -> Parameters2/1  "<Parameters>"
  Sensor_1_Front/2 -> SensorIndex3/1  "<SensorIndex>"
  Sensor_1_Front/3 -> SensorStatus/1  "<SensorStatus>"
  Sensor_1_Front/4 -> SensorOutput3/1  "<SensorOutput>"
  Sensor_1_Front/5 -> Info6/1  "<Info>"
  Object_Sensor_2D/4 -> Sensor_2_Front_Left/1  "<Sensor_2_Front_Left>"
  Sensor_2_Front_Left/1 -> Parameters3/1  "<Parameters>"
  Sensor_2_Front_Left/2 -> SensorIndex4/1  "<SensorIndex>"
  Sensor_2_Front_Left/3 -> SensorStatus1/1  "<SensorStatus>"
  Sensor_2_Front_Left/4 -> SensorOutput4/1  "<SensorOutput>"
  Sensor_2_Front_Left/5 -> Info7/1  "<Info>"
  Object_Sensor_2D/5 -> Sensor_3_Left/1  "<Sensor_3_Left>"
  Sensor_3_Left/1 -> Parameters4/1  "<Parameters>"
  Sensor_3_Left/2 -> SensorIndex5/1  "<SensorIndex>"
  Sensor_3_Left/3 -> SensorStatus2/1  "<SensorStatus>"
  Sensor_3_Left/4 -> SensorOutput5/1  "<SensorOutput>"
  Sensor_3_Left/5 -> Info8/1  "<Info>"
  Object_Sensor_2D/6 -> Sensor_4_Rear_Left/1  "<Sensor_4_Rear_Left>"
  Sensor_4_Rear_Left/1 -> Parameters5/1  "<Parameters>"
  Sensor_4_Rear_Left/2 -> SensorIndex6/1  "<SensorIndex>"
  Sensor_4_Rear_Left/3 -> SensorStatus3/1  "<SensorStatus>"
  Sensor_4_Rear_Left/4 -> SensorOutput6/1  "<SensorOutput>"
  Sensor_4_Rear_Left/5 -> Info9/1  "<Info>"
  Object_Sensor_2D/7 -> Sensor_5_Front_Right/1  "<Sensor_5_Front_Right>"
  Sensor_5_Front_Right/1 -> Parameters6/1  "<Parameters>"
  Sensor_5_Front_Right/2 -> SensorIndex7/1  "<SensorIndex>"
  Sensor_5_Front_Right/3 -> SensorStatus4/1  "<SensorStatus>"
  Sensor_5_Front_Right/4 -> SensorOutput7/1  "<SensorOutput>"
  Sensor_5_Front_Right/5 -> Info10/1  "<Info>"
  Object_Sensor_2D/8 -> Sensor_6_Right/1  "<Sensor_6_Right>"
  Sensor_6_Right/1 -> Parameters7/1  "<Parameters>"
  Sensor_6_Right/2 -> SensorIndex8/1  "<SensorIndex>"
  Sensor_6_Right/3 -> SensorStatus5/1  "<SensorStatus>"
  Sensor_6_Right/4 -> SensorOutput8/1  "<SensorOutput>"
  Sensor_6_Right/5 -> Info11/1  "<Info>"
  Object_Sensor_2D/9 -> Sensor_7_Rear_Right/1  "<Sensor_7_Rear_Right>"
  Sensor_7_Rear_Right/1 -> Parameters8/1  "<Parameters>"
  Sensor_7_Rear_Right/2 -> SensorIndex9/1  "<SensorIndex>"
  Sensor_7_Rear_Right/3 -> SensorStatus6/1  "<SensorStatus>"
  Sensor_7_Rear_Right/4 -> SensorOutput9/1  "<SensorOutput>"
  Sensor_7_Rear_Right/5 -> Info12/1  "<Info>"
  Sensors/3 -> TrafficSign_Sensor_Dyn/1  "<TrafficSign_Sensor_Dyn>"
  TrafficSign_Sensor_Dyn/1 -> Sensor_Front_1/1  "<Sensor_Front_1>"
  Sensor_Front_1/1 -> Info13/1  "<Info>"
  Sensor_Front_1/2 -> SensorOutput[]/1  "<SensorOutput[]>"
  Sensor_Front_1/3 -> Parameters9/1  "<Parameters>"
  Sensors/4 -> Custom_Sensor/1  "<Custom_Sensor>"
  Custom_Sensor/1 -> Sensor_Front_2/1  "<Sensor_Front_1>"
  Sensor_Front_2/1 -> Info14/1  "<Info>"
  Sensor_Front_2/2 -> SensorOutput10/1  "<SensorOutput>"
  SensorOutput10/1 -> Object1/1  "<Object1>"
  SensorOutput10/2 -> Object2/1  "<Object2>"
  SensorOutput10/3 -> Object3/1  "<Object3>"
  SensorOutput10/4 -> Object4/1  "<Object4>"
  SensorOutput10/5 -> Object5/1  "<Object5>"
  Sensor_Front_2/3 -> Parameters10/1  "<Parameters>"
  Sensors/5 -> Line_Sensor/1  "<Line_Sensor>"
  Line_Sensor/1 -> Line_Sensor_1/1  "<Line_Sensor_1>"
  Line_Sensor_1/1 -> Info15/1  "<Info>"
  Line_Sensor_1/2 -> Pos_Road_Lane_Animation_CoorSys_E/1  "<Pos_Road_Lane_Animation_CoorSys_E>"
  Line_Sensor_1/3 -> Pos_Road_Shape_Line_Animation_CoorSys_E/1  "<Pos_Road_Shape_Line_Animation_CoorSys_E>"
  Line_Sensor_1/4 -> Pos_Road_Shape_ContObj_Animation_CoorSys_E/1  "<Pos_Road_Shape_ContObj_Animation_CoorSys_E>"
  Line_Sensor_1/5 -> Pos_Junction_Border_Animation_CoorSys_E/1  "<Pos_Junction_Border_Animation_CoorSys_E>"
  Line_Sensor_1/6 -> Pos_Junction_Shape_Line_Animation_CoorSys_E/1  "<Pos_Junction_Shape_Line_Animation_CoorSys_E>"
  Line_Sensor_1/7 -> Pos_Junction_Shape_ContObj_Animation_CoorSys_E/1  "<Pos_Junction_Shape_ContObj_Animation_CoorSys_E>"
  Sensors/6 -> Collision_Sensor/1  "<Collision_Sensor>"
  Collision_Sensor/1 -> Collision_Sensor_1/1  "<Collision_Sensor_1>"
  Collision_Sensor_1/1 -> Info16/1  "<Info>"
  Collision_Sensor_1/2 -> SensorOutput11/1  "<SensorOutput>"
  Sensors/7 -> Sensors_Common/1  "<Sensors_Common>"
  ContentID/1 -> Terminator/1
  TorqueIntervention_Fast/1 -> DataTypeConversion_1/1  "<Enable_Trq_Intervention_Fast[0|1]>"
  DataTypeConversion_1/1 -> SignalFilter/1
  TorqueIntervention_Fast/2 -> SignalFilter/2  "<Trq_Request_Fast[Nm]>"
  TorqueIntervention_Fast/3 -> SignalFilter/3  "<Engine_Dynamic_Fast[0|1]>"
  TorqueIntervention_Slow/1 -> SignalFilter/4  "<Enable_Trq_Intervention_Fast[0|1]>"
  TorqueIntervention_Slow/2 -> SignalFilter/5  "<Trq_Request_Fast[Nm]>"
  TorqueIntervention_Slow/3 -> SignalFilter/6  "<Enable_TrqDecrease_ESP[0|1]>"
  TorqueIntervention_Slow/4 -> SignalFilter/7  "<Trq_DecreaseRequest_ESP[Nm]>"
  TorqueIntervention_Slow/5 -> SignalFilter/8  "<Enable_TrqDecrease_Extern[0|1]>"
  TorqueIntervention_Slow/6 -> SignalFilter/9  "<Trq_DecreaseRequest_Extern[Nm]>"
  TorqueIntervention_Slow/7 -> SignalFilter/10  "<Pos_AccPedal[%]>"
  TorqueIntervention_Slow/8 -> SignalFilter/11  "<Pos_AccPedal_Request_Fast_ESP[%]>"
  TorqueIntervention_Slow/9 -> SignalFilter/12  "<Pos_AccPedal_Request_Slow_ESP[%]>"
  TorqueIntervention_Slow/10 -> SignalFilter/13  "<Pos_AccPedal_Request_Extern[%]>"
  TorqueIntervention_Slow/11 -> SignalFilter/14  "<Pos_AccPedal_Influenced[%]>"
  IdleSpeedControl/1 -> SignalFilter/15  "<Const_n_Engine_Idle_Set[rpm]>"
  IdleSpeedControl/2 -> SignalFilter/16  "<Pos_AccPedal[%]>"
  EngineOperation/1 -> SignalFilter/17  "<Sw_Starter[0Off|1On]>"
  EngineOperation/2 -> SignalFilter/18  "<State_Engine[0|1|2|3|4]>"
  DesiredBrakePressure/1 -> SignalFilter/19  "<Enable_p_Brake_Desired[0|1]>"
  DesiredBrakePressure/2 -> SignalFilter/20  "<p_Brake_Desired[bar]>"
  Controller_ACC/1 -> SignalFilter/21  "<State_ACC[0Off|1On]>"
  Controller_ACC/2 -> SignalFilter/22  "<Sw_ACC_Distance[s]>"
  Controller_ACC/3 -> SignalFilter/23  "<Control_Mode_ACC[0Off|1CC|2DC]>"
  Controller_ACC/4 -> SignalFilter/24  "<v_Set_CC[km|h]>"
  Controller_ACC/5 -> SignalFilter/25  "<v_Set_DC[km|h]>"
  Controller_ACC/6 -> SignalFilter/26  "<v_Set[km|h]>"
  Controller_ACC/7 -> SignalFilter/27  "<a_x_Set[m|s2]>"
  Controller_ACC/8 -> SignalFilter/28  "<a_x_UpperLimit[m|s2]>"
  Controller_ACC/9 -> SignalFilter/29  "<a_x_LowerLimit[m|s2]>"
  Controller_ACC/10 -> SignalFilter/30  "<a_x_RisingRateMax[m|s3]>"
  Controller_ACC/11 -> SignalFilter/31  "<a_x_FallingRateMax[m|s3]s>"
  Controller_ACC/12 -> SignalFilter/32  "<Distance_Set[m]>"
  Controller_ACC/13 -> SignalFilter/33  "<Dist_Ref_Vehicle[m]>"
  Controller_ACC/14 -> SignalFilter/34  "<FCW[0Off|1On]>"
  Controller_ACC/15 -> SignalFilter/35  "<AEB[0Off|1On]>"
  Controller_ACC/16 -> SignalFilter/36  "<TTC[s]>"
  Controller_ACC/17 -> DataTypeConversion_37/1  "<Collision[0Off|1On]>"
  DataTypeConversion_37/1 -> SignalFilter/37
  Controller_ACC/18 -> SignalFilter/38  "<Sw_BrakeMode[1Comfort|2AEBOnly|3AEBOff]>"
  Controller_ACC/19 -> SignalFilter/39  "<Enable_Trq_Brake_ACC[0|1]>"
  Controller_ACC/20 -> SignalFilter/40  "<Enable_Trq_Engine_ACC[0|1]>"
  Interface_ACC/1 -> SignalFilter/41  "<Trq_Request_Brake_ACC[Nm]>"
  Interface_ACC/2 -> SignalFilter/42  "<Trq_Request_Engine_ACC[Nm]>"
  Operator_Interface_ACC/1 -> SignalFilter/43  "<Sw_ACC_On[0Off|1On]>"
  Operator_Interface_ACC/2 -> SignalFilter/44  "<Sw_ACC_Off[0Off|1On]>"
  Operator_Interface_ACC/3 -> SignalFilter/45  "<Sw_ACC_Cancel[0Off|1On]>"
  Operator_Interface_ACC/4 -> SignalFilter/46  "<Sw_ACC_Resume[0Off|1On]>"
  Operator_Interface_ACC/5 -> SignalFilter/47  "<Sw_ACC_Speed_Set[0Off|1On]>"
  Operator_Interface_ACC/6 -> SignalFilter/48  "<Sw_ACC_Speed_Increase[0Off|1On]>"
  Operator_Interface_ACC/7 -> SignalFilter/49  "<Sw_ACC_Speed_Decrease[0Off|1On]>"
  Operator_Interface_ACC/8 -> SignalFilter/50  "<ACC_State[1OFF|2Standby|3ON]>"
  Operator_Interface_ACC/9 -> SignalFilter/51  "<V_Set_CruiseControl[km|h]>"
  Target_Selection_ACC/1 -> SignalFilter/52  "<Target_Detected[0|1]>"
  Target_Selection_ACC/2 -> SignalFilter/53  "<Dist_Long[m]>"
  Target_Selection_ACC/3 -> SignalFilter/54  "<v_Rel[m|s]>"
  Target_Selection_ACC/4 -> Reshape_55/1  "<InLaneCheck[0|1]>"
  Reshape_55/1 -> SignalFilter/55
  Target_Selection_ACC/5 -> Reshape_56/1  "<LaneCrossingCheck[0|1]>"
  Reshape_56/1 -> SignalFilter/56
  Target_Selection_ACC/6 -> SignalFilter/57  "<v_Rel_Road[m|s]>"
  Target_Selection_ACC/7 -> SignalFilter/58  "<s_Fellows_Near[m]>"
  Lockup_Clutch_Control/1 -> SignalFilter/59  "<Ctrl_Lockup_Clutch[%]>"
  Shift_Lock_Control/1 -> SignalFilter/60  "<Ctrl_Parking_Pawl[0|1]>"
  Shift_Strategy/1 -> SignalFilter/61  "<Gear_Requested[]>"
  Tip_Shift_Control/1 -> SignalFilter/62  "<Gear_Requested[]>"
  Torque_Intervention_Control/1 -> SignalFilter/63  "<Gear[]>"
  Torque_Intervention_Control/2 -> SignalFilter/64  "<Factor_Trq_Engine_Red[%]>"
  SoftECU_PowerSteering/1 -> SignalFilter/65  "<Trq_PowerSteering[Nm]>"
  SoftECU_StartButton/1 -> DataTypeConversion_66/1  "<Flag_NotPressed_Pedal[0|1]>"
  DataTypeConversion_66/1 -> SignalFilter/66
  SoftECU_StartButton/2 -> SignalFilter/67  "<Lock[0|1]>"
  SoftECU_StartButton/3 -> SignalFilter/68  "<Sw_Acc[0|1]>"
  SoftECU_StartButton/4 -> SignalFilter/69  "<Sw_Ignition[0|1]>"
  SoftECU_StartButton/5 -> SignalFilter/70  "<Sw_StarterReq[0|1]>"
  SoftECU_StartButton/6 -> SignalFilter/71  "<State_StartButton[-2|-1|0|1|2|3]>"
  a_Vehicle_CoG[x;y;z][m|s2]/1 -> SignalFilter/72  "<a_x_Vehicle_CoG[m|s2]>"
  a_Vehicle_CoG[x;y;z][m|s2]/2 -> SignalFilter/73  "<a_y_Vehicle_CoG[m|s2]>"
  a_Vehicle_CoG[x;y;z][m|s2]/3 -> SignalFilter/74  "<a_z_Vehicle_CoG[m|s2]>"
  Linear/2 -> Reshape_75/1  "<a_Vehicle_Cog_withG[x;y;z][m|s2]>"
  Reshape_75/1 -> SignalFilter/75
  w_Vehicle_CoG_dt[x;y;z][rad|s2]/1 -> SignalFilter/76  "<w_x_Vehicle_CoG_dt[rad|s2]>"
  w_Vehicle_CoG_dt[x;y;z][rad|s2]/2 -> SignalFilter/77  "<w_y_Vehicle_CoG_dt[rad|s2]>"
  w_Vehicle_CoG_dt[x;y;z][rad|s2]/3 -> SignalFilter/78  "<w_z_Vehicle_CoG_dt[rad|s2]>"
  Linear1/1 -> Reshape_79/1  "<a_FL_Wheel[x;y;z][m|s2]>"
  Reshape_79/1 -> SignalFilter/79
  Linear1/2 -> Reshape_80/1  "<a_FR_Wheel[x;y;z][m|s2]>"
  Reshape_80/1 -> SignalFilter/80
  Linear1/3 -> Reshape_81/1  "<a_RL_Wheel[x;y;z][m|s2]>"
  Reshape_81/1 -> SignalFilter/81
  Linear1/4 -> Reshape_82/1  "<a_RR_Wheel[x;y;z][m|s2]>"
  Reshape_82/1 -> SignalFilter/82
  v_Vehicle_CoG[x;y;z][km|h]/1 -> SignalFilter/83  "<v_x_Vehicle_CoG[km|h]>"
  v_Vehicle_CoG[x;y;z][km|h]/2 -> SignalFilter/84  "<v_y_Vehicle_CoG[km|h]>"
  v_Vehicle_CoG[x;y;z][km|h]/3 -> SignalFilter/85  "<v_z_Vehicle_CoG[km|h]>"
  Linear2/2 -> SignalFilter/86  "<v_Total_Vehicle[km|h]>"
  Linear2/3 -> SignalFilter/87  "<Angle_SideSlip_Vehicle[deg]>"
  w_Vehicle_CoG[x;y;z][deg|s]/1 -> SignalFilter/88  "<RollRate_Vehicle_CoG[deg|s]>"
  w_Vehicle_CoG[x;y;z][deg|s]/2 -> SignalFilter/89  "<PitchRate_Vehicle_CoG[deg|s]>"
  w_Vehicle_CoG[x;y;z][deg|s]/3 -> SignalFilter/90  "<YawRate_Vehicle_CoG[deg|s]>"
  WheelBodyVelocity/1 -> Reshape_91/1  "<v_FL_Abs_WheelBody[x;y;z][km|h]>"
  Reshape_91/1 -> SignalFilter/91
  WheelBodyVelocity/2 -> Reshape_92/1  "<v_FR_Abs_WheelBody[x;y;z][km|h]>"
  Reshape_92/1 -> SignalFilter/92
  WheelBodyVelocity/3 -> Reshape_93/1  "<v_RL_Abs_WheelBody[x;y;z][km|h]>"
  Reshape_93/1 -> SignalFilter/93
  WheelBodyVelocity/4 -> Reshape_94/1  "<v_RR_Abs_WheelBody[x;y;z][km|h]>"
  Reshape_94/1 -> SignalFilter/94
  WheelBodyAngularVelocity/1 -> Reshape_95/1  "<w_FL_Abs_WheelBody[x;y;z][rad|s]>"
  Reshape_95/1 -> SignalFilter/95
  WheelBodyAngularVelocity/2 -> Reshape_96/1  "<w_FR_Abs_WheelBody[x;y;z][rad|s]>"
  Reshape_96/1 -> SignalFilter/96
  WheelBodyAngularVelocity/3 -> Reshape_97/1  "<w_RL_Abs_WheelBody[x;y;z][rad|s]>"
  Reshape_97/1 -> SignalFilter/97
  WheelBodyAngularVelocity/4 -> Reshape_98/1  "<w_RR_Abs_WheelBody[x;y;z][rad|s]>"
  Reshape_98/1 -> SignalFilter/98
  WheelAngularVelocity/1 -> Reshape_99/1  "<w_FL_Abs_Wheel[x;y;z][rad|s]>"
  Reshape_99/1 -> SignalFilter/99
  WheelAngularVelocity/2 -> Reshape_100/1  "<w_FR_Abs_Wheel[x;y;z][rad|s]>"
  Reshape_100/1 -> SignalFilter/100
  WheelAngularVelocity/3 -> Reshape_101/1  "<w_RL_Abs_Wheel[x;y;z][rad|s]>"
  Reshape_101/1 -> SignalFilter/101
  WheelAngularVelocity/4 -> Reshape_102/1  "<w_RR_Abs_Wheel[x;y;z][rad|s]>"
  Reshape_102/1 -> SignalFilter/102
  v_Vehicle[x;y;z][km|h]/1 -> SignalFilter/103  "<v_x_Vehicle[km|h]>"
  v_Vehicle[x;y;z][km|h]/2 -> SignalFilter/104  "<v_y_Vehicle[km|h]>"
  v_Vehicle[x;y;z][km|h]/3 -> SignalFilter/105  "<v_z_Vehicle[km|h]>"
  w_Vehicle[x;y;z][deg|s]/1 -> SignalFilter/106  "<RollRate_Vehicle[deg|s]>"
  w_Vehicle[x;y;z][deg|s]/2 -> SignalFilter/107  "<PitchRate_Vehicle[deg|s]>"
  w_Vehicle[x;y;z][deg|s]/3 -> SignalFilter/108  "<YawRate_Vehicle[deg|s]>"
  z_Wheel_dt[FL;FR;RL;RR][m|s]/1 -> SignalFilter/109  "<z_FL_Wheel_dt[m|s]>"
  z_Wheel_dt[FL;FR;RL;RR][m|s]/2 -> SignalFilter/110  "<z_FR_Wheel_dt[m|s]>"
  z_Wheel_dt[FL;FR;RL;RR][m|s]/3 -> SignalFilter/111  "<z_RL_Wheel_dt[m|s]>"
  z_Wheel_dt[FL;FR;RL;RR][m|s]/4 -> SignalFilter/112  "<z_RR_Wheel_dt[m|s]>"
  Pos_Vehicle_CoorSys_E[x;y;z][m]/1 -> SignalFilter/113  "<Pos_x_Vehicle_CoorSys_E[m]>"
  Pos_Vehicle_CoorSys_E[x;y;z][m]/2 -> SignalFilter/114  "<Pos_y_Vehicle_CoorSys_E[m]>"
  Pos_Vehicle_CoorSys_E[x;y;z][m]/3 -> SignalFilter/115  "<Pos_z_Vehicle_CoorSys_E[m]>"
  Linear4/2 -> SignalFilter/116  "<s_Vehicle[m]>"
  Angle_Vehicle_CoorSys_E[x;y;z][deg]/1 -> SignalFilter/117  "<Angle_Roll_Vehicle_CoorSys_E[deg]>"
  Angle_Vehicle_CoorSys_E[x;y;z][deg]/2 -> SignalFilter/118  "<Angle_Pitch_Vehicle_CoorSys_E[deg]>"
  Angle_Vehicle_CoorSys_E[x;y;z][deg]/3 -> SignalFilter/119  "<Angle_Yaw_Vehicle_CoorSys_E[deg]>"
  Angular3/2 -> Reshape_120/1  "<RotationMatrix_V_to_E[3x3]>"
  Reshape_120/1 -> SignalFilter/120
  Linear5/1 -> Reshape_121/1  "<Pos_FL_Wheels_CoorSys_E[x;y;z][m]>"
  Reshape_121/1 -> SignalFilter/121
  Linear5/2 -> Reshape_122/1  "<Pos_FR_Wheels_CoorSys_E[x;y;z][m]>"
  Reshape_122/1 -> SignalFilter/122
  Linear5/3 -> Reshape_123/1  "<Pos_RL_Wheels_CoorSys_E[x;y;z][m]>"
  Reshape_123/1 -> SignalFilter/123
  Linear5/4 -> Reshape_124/1  "<Pos_RR_Wheels_CoorSys_E[x;y;z][m]>"
  Reshape_124/1 -> SignalFilter/124
  GeneralizedForcesAndTorques/1 -> Reshape_125/1  "<g_F_Vehicle[x;y;z][N]>"
  Reshape_125/1 -> SignalFilter/125
  GeneralizedForcesAndTorques/2 -> Reshape_126/1  "<g_Trq_Vehicle[x;y;z][N]>"
  Reshape_126/1 -> SignalFilter/126
  GeneralizedForcesAndTorques/3 -> Reshape_127/1  "<g_F_z_Wheel[FL;FR;RL;RR][N]>"
  Reshape_127/1 -> SignalFilter/127
  GeneralizedVelocitiesDerivative/1 -> Reshape_128/1  "<v_Vehicle_dt[x;y;z][m|s2]>"
  Reshape_128/1 -> SignalFilter/128
  GeneralizedVelocitiesDerivative/2 -> Reshape_129/1  "<w_Vehicle_dt[x;y;z][rad|s2]>"
  Reshape_129/1 -> SignalFilter/129
  GeneralizedVelocitiesDerivative/3 -> Reshape_130/1  "<q_Wheel_dt2[q1_Front;q2_Front;q1_Rear;q2_Rear][]>"
  Reshape_130/1 -> SignalFilter/130
  GravityAcceleration/1 -> Reshape_131/1  "<a_Gravity_CoorSys_V[x;y;z][m|s2]>"
  Reshape_131/1 -> SignalFilter/131
  Sensor1/1 -> Reshape_132/1  "<a_Angular_Sensor1_CoorSys_V[x;y;z][rad|s2]>"
  Reshape_132/1 -> SignalFilter/132
  Sensor1/2 -> Reshape_133/1  "<a_Total_Sensor1_CoorSys_V[x;y;z][m|s2]>"
  Reshape_133/1 -> SignalFilter/133
  Sensor1/3 -> Reshape_134/1  "<a_Sensor1_CoorSys_V[x;y;z][m|s2]>"
  Reshape_134/1 -> SignalFilter/134
  Sensor1/4 -> Reshape_135/1  "<v_Sensor1_CoorSys_V[x;y;z][m|s]>"
  Reshape_135/1 -> SignalFilter/135
  Sensor1/5 -> Reshape_136/1  "<w_Sensor1_CoorSys_V[x;y;z][rad|s]>"
  Reshape_136/1 -> SignalFilter/136
  Sensor1/6 -> Reshape_137/1  "<a_Angular_Sensor1_CoorSys_VH[x;y;z][rad|s2]>"
  Reshape_137/1 -> SignalFilter/137
  Sensor1/7 -> Reshape_138/1  "<a_Total_Sensor1_CoorSys_VH[x;y;z][m|s2]>"
  Reshape_138/1 -> SignalFilter/138
  Sensor1/8 -> Reshape_139/1  "<a_Sensor1_CoorSys_VH[x;y;z][m|s2]>"
  Reshape_139/1 -> SignalFilter/139
  Sensor1/9 -> Reshape_140/1  "<v_Sensor1_CoorSys_VH[x;y;z][m|s]>"
  Reshape_140/1 -> SignalFilter/140
  Sensor1/10 -> Reshape_141/1  "<w_Sensor1_CoorSys_VH[x;y;z][rad|s]>"
  Reshape_141/1 -> SignalFilter/141
  Sensor2/1 -> Reshape_142/1  "<a_Angular_Sensor2_CoorSys_V[x;y;z][rad|s2]>"
  Reshape_142/1 -> SignalFilter/142
  Sensor2/2 -> Reshape_143/1  "<a_Total_Sensor2_CoorSys_V[x;y;z][m|s2]>"
  Reshape_143/1 -> SignalFilter/143
  Sensor2/3 -> Reshape_144/1  "<a_Sensor2_CoorSys_V[x;y;z][m|s2]>"
  Reshape_144/1 -> SignalFilter/144
  Sensor2/4 -> Reshape_145/1  "<v_Sensor2_CoorSys_V[x;y;z][m|s]>"
  Reshape_145/1 -> SignalFilter/145
  Sensor2/5 -> Reshape_146/1  "<w_Sensor2_CoorSys_V[x;y;z][rad|s]>"
  Reshape_146/1 -> SignalFilter/146
  Sensor2/6 -> Reshape_147/1  "<a_Angular_Sensor2_CoorSys_VH[x;y;z][rad|s2]>"
  Reshape_147/1 -> SignalFilter/147
  Sensor2/7 -> Reshape_148/1  "<a_Total_Sensor2_CoorSys_VH[x;y;z][m|s2]>"
  Reshape_148/1 -> SignalFilter/148
  Sensor2/8 -> Reshape_149/1  "<a_Sensor2_CoorSys_VH[x;y;z][m|s2]>"
  Reshape_149/1 -> SignalFilter/149
  Sensor2/9 -> Reshape_150/1  "<v_Sensor2_CoorSys_VH[x;y;z][m|s]>"
  Reshape_150/1 -> SignalFilter/150
  Sensor2/10 -> Reshape_151/1  "<w_Sensor2_CoorSys_VH[x;y;z][rad|s]>"
  Reshape_151/1 -> SignalFilter/151
  Sensor3/1 -> Reshape_152/1  "<a_Angular_Sensor3_CoorSys_V[x;y;z][rad|s2]>"
  Reshape_152/1 -> SignalFilter/152
  Sensor3/2 -> Reshape_153/1  "<a_Total_Sensor3_CoorSys_V[x;y;z][m|s2]>"
  Reshape_153/1 -> SignalFilter/153
  Sensor3/3 -> Reshape_154/1  "<a_Sensor3_CoorSys_V[x;y;z][m|s2]>"
  Reshape_154/1 -> SignalFilter/154
  Sensor3/4 -> Reshape_155/1  "<v_Sensor3_CoorSys_V[x;y;z][m|s]>"
  Reshape_155/1 -> SignalFilter/155
  Sensor3/5 -> Reshape_156/1  "<w_Sensor3_CoorSys_V[x;y;z][rad|s]>"
  Reshape_156/1 -> SignalFilter/156
  Sensor3/6 -> Reshape_157/1  "<a_Angular_Sensor3_CoorSys_VH[x;y;z][rad|s2]>"
  Reshape_157/1 -> SignalFilter/157
  Sensor3/7 -> Reshape_158/1  "<a_Total_Sensor3_CoorSys_VH[x;y;z][m|s2]>"
  Reshape_158/1 -> SignalFilter/158
  Sensor3/8 -> Reshape_159/1  "<a_Sensor3_CoorSys_VH[x;y;z][m|s2]>"
  Reshape_159/1 -> SignalFilter/159
  Sensor3/9 -> Reshape_160/1  "<v_Sensor3_CoorSys_VH[x;y;z][m|s]>"
  Reshape_160/1 -> SignalFilter/160
  Sensor3/10 -> Reshape_161/1  "<w_Sensor3_CoorSys_VH[x;y;z][rad|s]>"
  Reshape_161/1 -> SignalFilter/161
  Sensor4/1 -> Reshape_162/1  "<a_Angular_Sensor4_CoorSys_V[x;y;z][rad|s2]>"
  Reshape_162/1 -> SignalFilter/162
  Sensor4/2 -> Reshape_163/1  "<a_Total_Sensor4_CoorSys_V[x;y;z][m|s2]>"
  Reshape_163/1 -> SignalFilter/163
  Sensor4/3 -> Reshape_164/1  "<a_Sensor4_CoorSys_V[x;y;z][m|s2]>"
  Reshape_164/1 -> SignalFilter/164
  Sensor4/4 -> Reshape_165/1  "<v_Sensor4_CoorSys_V[x;y;z][m|s]>"
  Reshape_165/1 -> SignalFilter/165
  Sensor4/5 -> Reshape_166/1  "<w_Sensor4_CoorSys_V[x;y;z][rad|s]>"
  Reshape_166/1 -> SignalFilter/166
  Sensor4/6 -> Reshape_167/1  "<a_Angular_Sensor4_CoorSys_VH[x;y;z][rad|s2]>"
  Reshape_167/1 -> SignalFilter/167
  Sensor4/7 -> Reshape_168/1  "<a_Total_Sensor4_CoorSys_VH[x;y;z][m|s2]>"
  Reshape_168/1 -> SignalFilter/168
  Sensor4/8 -> Reshape_169/1  "<a_Sensor4_CoorSys_VH[x;y;z][m|s2]>"
  Reshape_169/1 -> SignalFilter/169
  Sensor4/9 -> Reshape_170/1  "<v_Sensor4_CoorSys_VH[x;y;z][m|s]>"
  Reshape_170/1 -> SignalFilter/170
  Sensor4/10 -> Reshape_171/1  "<w_Sensor4_CoorSys_VH[x;y;z][rad|s]>"
  Reshape_171/1 -> SignalFilter/171
  VehicleMassAndAdditionalLoads/1 -> SignalFilter/172  "<m_TotalVehicle[kg]>"
  VehicleMassAndAdditionalLoads/2 -> Reshape_173/1  "<PosVec_CoG_TotalVehicle[x;y;z][m]>"
  Reshape_173/1 -> SignalFilter/173
  VehicleMassAndAdditionalLoads/3 -> Reshape_174/1  "<Inertia_Tensor_TotalVehicle[3x3][kgm2]>"
  Reshape_174/1 -> SignalFilter/174
  VehicleMassAndAdditionalLoads/4 -> SignalFilter/175  "<m_TotalV1[kg]>"
  VehicleMassAndAdditionalLoads/5 -> Reshape_176/1  "<PosVec_CoG_TotalV1[x;y;z][m]>"
  Reshape_176/1 -> SignalFilter/176
  VehicleMassAndAdditionalLoads/6 -> Reshape_177/1  "<Inertia_Tensor_TotalV1[3x3][kgm2]>"
  Reshape_177/1 -> SignalFilter/177
  GravitationalForces/1 -> Reshape_178/1  "<F_Vehicle_Gravitational[x;y;z][N]>"
  Reshape_178/1 -> SignalFilter/178
  GravitationalForces/2 -> Reshape_179/1  "<F_FL_Gravitational[x;y;z][N]>"
  Reshape_179/1 -> SignalFilter/179
  GravitationalForces/3 -> Reshape_180/1  "<F_FR_Gravitational[x;y;z][N]>"
  Reshape_180/1 -> SignalFilter/180
  GravitationalForces/4 -> Reshape_181/1  "<F_RL_Gravitational[x;y;z][N]>"
  Reshape_181/1 -> SignalFilter/181
  GravitationalForces/5 -> Reshape_182/1  "<F_RR_Gravitationa[x;y;z]l[N]>"
  Reshape_182/1 -> SignalFilter/182
  GyroscopicForces/1 -> Reshape_183/1  "<F_Vehicle_Gyroscopic[x;y;z][N]>"
  Reshape_183/1 -> SignalFilter/183
  GyroscopicForces/2 -> Reshape_184/1  "<F_FL_Gyroscopic[x;y;z][N]>"
  Reshape_184/1 -> SignalFilter/184
  GyroscopicForces/3 -> Reshape_185/1  "<F_FR_Gyroscopic[x;y;z][N]>"
  Reshape_185/1 -> SignalFilter/185
  GyroscopicForces/4 -> Reshape_186/1  "<F_RL_Gyroscopic[x;y;z][N]>"
  Reshape_186/1 -> SignalFilter/186
  GyroscopicForces/5 -> Reshape_187/1  "<F_RR_Gyroscopic[x;y;z][N]>"
  Reshape_187/1 -> SignalFilter/187
  GyroscopicTorques/1 -> Reshape_188/1  "<Trq_Vehicle_Gyroscope[x;y;z][Nm]>"
  Reshape_188/1 -> SignalFilter/188
  GyroscopicTorques/2 -> Reshape_189/1  "<Trq_FL_Gyroscope[x;y;z][Nm]>"
  Reshape_189/1 -> SignalFilter/189
  GyroscopicTorques/3 -> Reshape_190/1  "<Trq_FR_Gyroscope[x;y;z][Nm]>"
  Reshape_190/1 -> SignalFilter/190
  GyroscopicTorques/4 -> Reshape_191/1  "<Trq_RL_Gyroscope[x;y;z][Nm]>"
  Reshape_191/1 -> SignalFilter/191
  GyroscopicTorques/5 -> Reshape_192/1  "<Trq_RR_Gyroscope[x;y;z][Nm]>"
  Reshape_192/1 -> SignalFilter/192
  ResidualAccelerations/1 -> Reshape_193/1  "<a_Vehicle_CoG_Residual[x;y;z][m|s2]>"
  Reshape_193/1 -> SignalFilter/193
  ResidualAccelerations/2 -> Reshape_194/1  "<a_FL_Residual[x;y;z][m|s2]>"
  Reshape_194/1 -> SignalFilter/194
  ResidualAccelerations/3 -> Reshape_195/1  "<a_FR_Residual[x;y;z][m|s2]>"
  Reshape_195/1 -> SignalFilter/195
  ResidualAccelerations/4 -> Reshape_196/1  "<a_RL_Residua[x;y;z]l[m|s2]>"
  Reshape_196/1 -> SignalFilter/196
  ResidualAccelerations/5 -> Reshape_197/1  "<a_RR_Residual[x;y;z][m|s2]>"
  Reshape_197/1 -> SignalFilter/197
  ContactPoint/1 -> SignalFilter/198  "<r_FL_Tire[m]>"
  ContactPoint/2 -> Reshape_199/1  "<Pos_CP_FL_CoorSys_E[x;y][m]>"
  Reshape_199/1 -> SignalFilter/199
  F_FL_Tire_CoorSys_V[x;y;z][N]/1 -> SignalFilter/200  "<F_x_FL_Tire_CoorSys_V[N]>"
  F_FL_Tire_CoorSys_V[x;y;z][N]/2 -> SignalFilter/201  "<F_y_FL_Tire_CoorSys_V[N]>"
  F_FL_Tire_CoorSys_V[x;y;z][N]/3 -> SignalFilter/202  "<F_z_FL_Tire_CoorSys_V[N]>"
  Trq_FL_Tire_CoorSys_V[x;y;z][Nm]/1 -> SignalFilter/203  "<Trq_x_FL_Tire_CoorSys_V[Nm]>"
  Trq_FL_Tire_CoorSys_V[x;y;z][Nm]/2 -> SignalFilter/204  "<Trq_y_FL_Tire_CoorSys_V[Nm]>"
  Trq_FL_Tire_CoorSys_V[x;y;z][Nm]/3 -> SignalFilter/205  "<Trq_z_FL_Tire_CoorSys_V[Nm]>"
  ActiveTire/1 -> SignalFilter/206  "<v_Circumf_Dyn_FL_Wheel[km|h]>"
  ActiveTire/2 -> SignalFilter/207  "<Slip_x_FL[]>"
  ActiveTire/3 -> SignalFilter/208  "<Slip_y_FL[]>"
  ActiveTire/4 -> SignalFilter/209  "<r_Dyn_FL_Tire[m]>"
  ActiveTire/5 -> SignalFilter/210  "<CorneringStiffness_FL[N]>"
  ActiveTire/6 -> SignalFilter/211  "<Coef_RollingRes_FL[]>"
  ActiveTire/7 -> SignalFilter/212  "<Trq_x_FL_CoorSys_CP[Nm]>"
  ActiveTire/8 -> SignalFilter/213  "<Trq_y_FL_CoorSys_W[Nm]>"
  ActiveTire/9 -> SignalFilter/214  "<Trq_z_FL_CoorSys_CP[Nm]>"
  ActiveTire/10 -> SignalFilter/215  "<F_x_Dyn_FL_Tire_CoorSys_CP[N]>"
  ActiveTire/11 -> SignalFilter/216  "<F_y_Dyn_FL_Tire_CoorSys_CP[N]>"
  ActiveTire/12 -> SignalFilter/217  "<F_z_Dyn_FL_Tire_CoorSys_CP[N]>"
  ContactPoint1/1 -> SignalFilter/218  "<r_FR_Tire[m]>"
  ContactPoint1/2 -> Reshape_219/1  "<Pos_CP_FR_CoorSys_E[x;y][m]>"
  Reshape_219/1 -> SignalFilter/219
  F_FR_Tire_CoorSys_V[x;y;z][N]/1 -> SignalFilter/220  "<F_x_FR_Tire_CoorSys_V[N]>"
  F_FR_Tire_CoorSys_V[x;y;z][N]/2 -> SignalFilter/221  "<F_y_FR_Tire_CoorSys_V[N]>"
  F_FR_Tire_CoorSys_V[x;y;z][N]/3 -> SignalFilter/222  "<F_z_FR_Tire_CoorSys_V[N]>"
  Trq_FR_Tire_CoorSys_V[x;y;z][Nm]/1 -> SignalFilter/223  "<Trq_x_FR_Tire_CoorSys_V[Nm]>"
  Trq_FR_Tire_CoorSys_V[x;y;z][Nm]/2 -> SignalFilter/224  "<Trq_y_FR_Tire_CoorSys_V[Nm]>"
  Trq_FR_Tire_CoorSys_V[x;y;z][Nm]/3 -> SignalFilter/225  "<Trq_z_FR_Tire_CoorSys_V[Nm]>"
  ActiveTire1/1 -> SignalFilter/226  "<v_Circumf_Dyn_FR_Wheel[km|h]>"
  ActiveTire1/2 -> SignalFilter/227  "<Slip_x_FR[]>"
  ActiveTire1/3 -> SignalFilter/228  "<Slip_y_FR[]>"
  ActiveTire1/4 -> SignalFilter/229  "<r_Dyn_FR_Tire[m]>"
  ActiveTire1/5 -> SignalFilter/230  "<CorneringStiffness_FR[N]>"
  ActiveTire1/6 -> SignalFilter/231  "<Coef_RollingRes_FR[]>"
  ActiveTire1/7 -> SignalFilter/232  "<Trq_x_FR_CoorSys_CP[Nm]>"
  ActiveTire1/8 -> SignalFilter/233  "<Trq_y_FR_CoorSys_W[Nm]>"
  ActiveTire1/9 -> SignalFilter/234  "<Trq_z_FR_CoorSys_CP[Nm]>"
  ActiveTire1/10 -> SignalFilter/235  "<F_x_Dyn_FR_Tire_CoorSys_CP[N]>"
  ActiveTire1/11 -> SignalFilter/236  "<F_y_Dyn_FR_Tire_CoorSys_CP[N]>"
  ActiveTire1/12 -> SignalFilter/237  "<F_z_Dyn_FR_Tire_CoorSys_CP[N]>"
  ContactPoint2/1 -> SignalFilter/238  "<r_RL_Tire[m]>"
  ContactPoint2/2 -> Reshape_239/1  "<Pos_CP_RL_CoorSys_E[x;y][m]>"
  Reshape_239/1 -> SignalFilter/239
  F_RL_Tire_CoorSys_V[x;y;z][N]/1 -> SignalFilter/240  "<F_x_RL_Tire_CoorSys_V[N]>"
  F_RL_Tire_CoorSys_V[x;y;z][N]/2 -> SignalFilter/241  "<F_y_RL_Tire_CoorSys_V[N]>"
  F_RL_Tire_CoorSys_V[x;y;z][N]/3 -> SignalFilter/242  "<F_z_RL_Tire_CoorSys_V[N]>"
  Trq_RL_Tire_CoorSys_V[x;y;z][Nm]/1 -> SignalFilter/243  "<Trq_x_RL_Tire_CoorSys_V[Nm]>"
  Trq_RL_Tire_CoorSys_V[x;y;z][Nm]/2 -> SignalFilter/244  "<Trq_y_RL_Tire_CoorSys_V[Nm]>"
  Trq_RL_Tire_CoorSys_V[x;y;z][Nm]/3 -> SignalFilter/245  "<Trq_z_RL_Tire_CoorSys_V[Nm]>"
  ActiveTire2/1 -> SignalFilter/246  "<v_Circumf_Dyn_RL_Wheel[km|h]>"
  ActiveTire2/2 -> SignalFilter/247  "<Slip_x_RL[]>"
  ActiveTire2/3 -> SignalFilter/248  "<Slip_y_RL[]>"
  ActiveTire2/4 -> SignalFilter/249  "<r_Dyn_RL_Tire[m]>"
  ActiveTire2/5 -> SignalFilter/250  "<CorneringStiffness_RL[N]>"
  ActiveTire2/6 -> SignalFilter/251  "<Coef_RollingRes_RL[]>"
  ActiveTire2/7 -> SignalFilter/252  "<Trq_x_RL_CoorSys_CP[Nm]>"
  ActiveTire2/8 -> SignalFilter/253  "<Trq_y_RL_CoorSys_W[Nm]>"
  ActiveTire2/9 -> SignalFilter/254  "<Trq_z_RL_CoorSys_CP[Nm]>"
  ActiveTire2/10 -> SignalFilter/255  "<F_x_Dyn_RL_Tire_CoorSys_CP[N]>"
  ActiveTire2/11 -> SignalFilter/256  "<F_y_Dyn_RL_Tire_CoorSys_CP[N]>"
  ActiveTire2/12 -> SignalFilter/257  "<F_z_Dyn_RL_Tire_CoorSys_CP[N]>"
  ContactPoint3/1 -> SignalFilter/258  "<r_RR_Tire[m]>"
  ContactPoint3/2 -> Reshape_259/1  "<Pos_CP_RR_CoorSys_E[x;y][m]>"
  Reshape_259/1 -> SignalFilter/259
  F_RR_Tire_CoorSys_V[x;y;z][N]/1 -> SignalFilter/260  "<F_x_RR_Tire_CoorSys_V[N]>"
  F_RR_Tire_CoorSys_V[x;y;z][N]/2 -> SignalFilter/261  "<F_y_RR_Tire_CoorSys_V[N]>"
  F_RR_Tire_CoorSys_V[x;y;z][N]/3 -> SignalFilter/262  "<F_z_RR_Tire_CoorSys_V[N]>"
  Trq_RR_Tire_CoorSys_V[x;y;z][Nm]/1 -> SignalFilter/263  "<Trq_x_RR_Tire_CoorSys_V[Nm]>"
  Trq_RR_Tire_CoorSys_V[x;y;z][Nm]/2 -> SignalFilter/264  "<Trq_y_RR_Tire_CoorSys_V[Nm]>"
  Trq_RR_Tire_CoorSys_V[x;y;z][Nm]/3 -> SignalFilter/265  "<Trq_z_RR_Tire_CoorSys_V[Nm]>"
  ActiveTire3/1 -> SignalFilter/266  "<v_Circumf_Dyn_RR_Wheel[km|h]>"
  ActiveTire3/2 -> SignalFilter/267  "<Slip_x_RR[]>"
  ActiveTire3/3 -> SignalFilter/268  "<Slip_y_RR[]>"
  ActiveTire3/4 -> SignalFilter/269  "<r_Dyn_RR_Tire[m]>"
  ActiveTire3/5 -> SignalFilter/270  "<CorneringStiffness_RR[N]>"
  ActiveTire3/6 -> SignalFilter/271  "<Coef_RollingRes_RR[]>"
  ActiveTire3/7 -> SignalFilter/272  "<Trq_x_RR_CoorSys_CP[Nm]>"
  ActiveTire3/8 -> SignalFilter/273  "<Trq_y_RR_CoorSys_W[Nm]>"
  ActiveTire3/9 -> SignalFilter/274  "<Trq_z_RR_CoorSys_CP[Nm]>"
  ActiveTire3/10 -> SignalFilter/275  "<F_x_Dyn_RR_Tire_CoorSys_CP[N]>"
  ActiveTire3/11 -> SignalFilter/276  "<F_y_Dyn_RR_Tire_CoorSys_CP[N]>"
  ActiveTire3/12 -> SignalFilter/277  "<F_z_Dyn_RR_Tire_CoorSys_CP[N]>"
  TireModelSwitch/1 -> SignalFilter/278  "<Sw_Tire_Model[1TMEasy|2MF]>"
  Forces/1 -> SignalFilter/279  "<F_x_Aero_CoorSys_V[N]>"
  Forces/2 -> SignalFilter/280  "<F_y_Aero_CoorSys_V[N]>"
  Forces/3 -> SignalFilter/281  "<F_z_Aero_CoorSys_V[N]>"
  Torques/1 -> SignalFilter/282  "<Trq_x_Aero_CoorSys_V[Nm]>"
  Torques/2 -> SignalFilter/283  "<Trq_y_Aero_CoorSys_V[Nm]>"
  Torques/3 -> SignalFilter/284  "<Trq_z_Aero_CoorSys_V[Nm]>"
  Coefficients/1 -> SignalFilter/285  "<Cw_x[]>"
  WheelSpeed_CoorSys_V/1 -> Reshape_286/1  "<w_Wheel_FL_CoorSys_V[x;y;z][rad|s]>"
  Reshape_286/1 -> SignalFilter/286
  WheelSpeed_CoorSys_V/2 -> Reshape_287/1  "<w_Wheel_FR_CoorSys_V[x;y;z][rad|s]>"
  Reshape_287/1 -> SignalFilter/287
  WheelSpeed_CoorSys_V/3 -> Reshape_288/1  "<w_Wheel_RL_CoorSys_V[x;y;z][rad|s]>"
  Reshape_288/1 -> SignalFilter/288
  WheelSpeed_CoorSys_V/4 -> Reshape_289/1  "<w_Wheel_RR_CoorSys_V[x;y;z][rad|s]>"
  Reshape_289/1 -> SignalFilter/289
  ShaftsTorques_CoorSys_V/1 -> Reshape_290/1  "<Trq_Shaft_FL_CoorSys_V[x;y;z][Nm]>"
  Reshape_290/1 -> SignalFilter/290
  ShaftsTorques_CoorSys_V/2 -> Reshape_291/1  "<Trq_Shaft_FR_CoorSys_V[x;y;z][Nm]>"
  Reshape_291/1 -> SignalFilter/291
  ShaftsTorques_CoorSys_V/3 -> Reshape_292/1  "<Trq_Shaft_RL_CoorSys_V[x;y;z][Nm]>"
  Reshape_292/1 -> SignalFilter/292
  ShaftsTorques_CoorSys_V/4 -> Reshape_293/1  "<Trq_Shaft_RR_CoorSys_V[x;y;z][Nm]>"
  Reshape_293/1 -> SignalFilter/293
  TireWheelTorques/1 -> SignalFilter/294  "<Trq_Tire_Whee_FL[Nm]>"
  TireWheelTorques/2 -> SignalFilter/295  "<Trq_Tire_Whee_FR[Nm]>"
  TireWheelTorques/3 -> SignalFilter/296  "<Trq_Tire_Whee_RL[Nm]>"
  TireWheelTorques/4 -> SignalFilter/297  "<Trq_Tire_Whee_RR[Nm]>"
  WheelSpeed/1 -> SignalFilter/298  "<omega_FL_Wheel[rad|s]>"
  WheelSpeed/2 -> SignalFilter/299  "<omega_FR_Wheel[rad|s]>"
  WheelSpeed/3 -> SignalFilter/300  "<omega_RL_Wheel[rad|s]>"
  WheelSpeed/4 -> SignalFilter/301  "<omega_RR_Wheel[rad|s]>"
  RotationAngle/1 -> SignalFilter/302  "<Angle_Rot_FL_Wheel[deg]>"
  RotationAngle/2 -> SignalFilter/303  "<Angle_Rot_FR_Wheel[deg]>"
  RotationAngle/3 -> SignalFilter/304  "<Angle_Rot_RL_Wheel[deg]>"
  RotationAngle/4 -> SignalFilter/305  "<Angle_Rot_RR_Wheel[deg]>"
  Steering/1 -> SignalFilter/306  "<Displ_Steering[m]>"
  Steering/2 -> SignalFilter/307  "<Displ_Steering_dt[m|s]>"
  Steering/3 -> SignalFilter/308  "<Displ_SteeringRod_dt2[m|s2]>"
  Steering/4 -> SignalFilter/309  "<m_Steering[kg]>"
  ForcesAndTorques/1 -> SignalFilter/310  "<g_F_Steering_SteeringRod[N]>"
  ForcesAndTorques/2 -> SignalFilter/311  "<Trq_Steering[Nm]>"
  ForcesAndTorques/3 -> SignalFilter/312  "<Trq_PowerSteering[Nm]>"
  ForcesAndTorques/4 -> SignalFilter/313  "<TrqSpring_SteeringColumn[Nm]>"
  ForcesAndTorques/5 -> SignalFilter/314  "<Trq_PowerSteeringDynamics[Nm]>"
  ForcesAndTorques/6 -> SignalFilter/315  "<TrqSpring_PowerSteeringSystem[Nm]>"
  GeneralizedForcesAndTorques1/1 -> SignalFilter/316  "<g_FTrq_Tire_Steering[N]>"
  GeneralizedForcesAndTorques1/2 -> SignalFilter/317  "<g_Trq_FL_Steering[N]>"
  GeneralizedForcesAndTorques1/3 -> SignalFilter/318  "<g_Trq_FR_Steering[N]>"
  GeneralizedForcesAndTorques1/4 -> SignalFilter/319  "<g_F_FL_Steering[N]>"
  GeneralizedForcesAndTorques1/5 -> SignalFilter/320  "<g_F_FR_Steering[N]>"
  Steering/7 -> SignalFilter/321  "<i_Steering[rad|m]>"
  Steering/8 -> SignalFilter/322  "<i_Steering_Mean[]>"
  Steering/9 -> SignalFilter/323  "<Angle_SteeringGear[deg]>"
  Steering/10 -> SignalFilter/324  "<Angle_SteeringWheel[deg]>"
  Steering/11 -> SignalFilter/325  "<Angle_SteeringGear_dt[deg|s]>"
  Steering/12 -> SignalFilter/326  "<Angle_SteeringWheel_dt[deg|s]>"
  Steering/13 -> SignalFilter/327  "<Const_Stiffness_SteeringColumn[Nm|rad]>"
  StatesSteeringSystem/1 -> SignalFilter/328  "<Angle_EPSSystem[deg]>"
  StatesSteeringSystem/2 -> SignalFilter/329  "<Angle_EPSSystem_dt[deg|s]>"
  StatesSteeringSystem/3 -> SignalFilter/330  "<Angle_LowerSteeringColumn[deg]>"
  StatesSteeringSystem/4 -> SignalFilter/331  "<Angle_LowerSteeringColumn_dt[deg|s]>"
  StatesSteeringSystem/5 -> SignalFilter/332  "<Angle_UpperSteeringColumn[deg]>"
  StatesSteeringSystem/6 -> SignalFilter/333  "<Angle_UpperSteeringColumn_dt[deg|s]>"
  StatesSteeringSystem/7 -> SignalFilter/334  "<Angle_SteeringWheel[deg]>"
  StatesSteeringSystem/8 -> SignalFilter/335  "<Angle_SteeringWheel_dt[deg|s]>"
  StatesSteeringSystem/9 -> SignalFilter/336  "<Displ_Steering[m]>"
  StatesSteeringSystem/10 -> SignalFilter/337  "<Displ_Steering_dt[m|s]>"
  StatesSteeringSystem/11 -> SignalFilter/338  "<Displ_SteeringRod_dt2[m|s2]>"
  StatesSteeringSystem/12 -> SignalFilter/339  "<Angle_SteeringGear[deg]>"
  StatesSteeringSystem/13 -> SignalFilter/340  "<Angle_SteeringGear_dt[deg|s]>"
  StatesSteeringSystem/14 -> SignalFilter/341  "<Angle_EPSPinion[rad]>"
  StatesSteeringSystem/15 -> SignalFilter/342  "<Angle_EPSPinion_dt[rad|s]>"
  StatesSteeringSystem/16 -> SignalFilter/343  "<i_Steering[rad|m]>"
  StatesSteeringSystem/17 -> SignalFilter/344  "<FrictionForce_SteeringRod[N]>"
  StatesSteeringSystem/18 -> SignalFilter/345  "<i_Steering_Wheel2Rod[rad|m]>"
  Steering/15 -> SignalFilter/346  "<FrictionTrq_SteeringSystem[Nm]>"
  SteeringWheelTorque/1 -> SignalFilter/347  "<TrqSensor_Steering[Nm]>"
  SteeringWheelTorque/2 -> SignalFilter/348  "<Trq_Driver[Nm]>"
  SteeringWheelTorque/3 -> SignalFilter/349  "<g_torque_SteeringWheel[Nm]>"
  SteeringWheelTorque/4 -> SignalFilter/350  "<TrqFriction_SteeringWheel[Nm]>"
  SteeringWheelTorque/5 -> SignalFilter/351  "<Trq_SteeringWheel[Nm]>"
  ActiveBrakeCylinder/1 -> SignalFilter/352  "<p[bar]>"
  ActiveBrakeCylinder/2 -> SignalFilter/353  "<p_max[bar]>"
  ActiveBrakeCylinder/3 -> SignalFilter/354  "<Enable_p_Brake_Desired[0|1]>"
  ActiveBrakeCylinder/4 -> SignalFilter/355  "<p_Brake_Desired[bar]>"
  BrakeCylinderLinear/1 -> SignalFilter/356  "<p[bar]>"
  BrakeCylinderLinear/2 -> SignalFilter/357  "<p_max[bar]>"
  BrakeCylinderPhysical/1 -> SignalFilter/358  "<Displ_Piston[mm]>"
  BrakeCylinderPhysical/2 -> SignalFilter/359  "<F[N]>"
  BrakeCylinderPhysical/3 -> SignalFilter/360  "<p[bar]>"
  BrakeCylinderPhysical/4 -> SignalFilter/361  "<p_max[bar]>"
  Pressure/1 -> SignalFilter/362  "<p_FL_Brake[bar]>"
  Pressure/2 -> SignalFilter/363  "<p_FR_Brake[bar]>"
  Pressure/3 -> SignalFilter/364  "<p_RL_Brake[bar]>"
  Pressure/4 -> SignalFilter/365  "<p_RR_Brake[bar]>"
  BrakeHydraulics/2 -> SignalFilter/366  "<BrakeHydraulicsModel[]>"
  Torque/1 -> SignalFilter/367  "<Trq_FL_Brake[Nm]>"
  Torque/2 -> SignalFilter/368  "<Trq_FR_Brake[Nm]>"
  Torque/3 -> SignalFilter/369  "<Trq_RL_Brake[Nm]>"
  Torque/4 -> SignalFilter/370  "<Trq_RR_Brake[Nm]>"
  MaximumTorque/1 -> SignalFilter/371  "<Trq_FL_max_Brake[Nm]>"
  MaximumTorque/2 -> SignalFilter/372  "<Trq_FR_max_Brake[Nm]>"
  MaximumTorque/3 -> SignalFilter/373  "<Trq_RL_max_Brake[Nm]>"
  MaximumTorque/4 -> SignalFilter/374  "<Trq_RR_max_Brake[Nm]>"
  Pressure1/1 -> SignalFilter/375  "<p_FL_Brake[bar]>"
  Pressure1/2 -> SignalFilter/376  "<p_FR_Brake[bar]>"
  Pressure1/3 -> SignalFilter/377  "<p_RL_Brake[bar]>"
  Pressure1/4 -> SignalFilter/378  "<p_RR_Brake[bar]>"
  Const_BrakeDiscFactor/1 -> SignalFilter/379  "<Const_BrakeDiscFactor_FL[m3]>"
  Const_BrakeDiscFactor/2 -> SignalFilter/380  "<Const_BrakeDiscFactor_FR[m3]>"
  Const_BrakeDiscFactor/3 -> SignalFilter/381  "<Const_BrakeDiscFactor_RL[m3]>"
  Const_BrakeDiscFactor/4 -> SignalFilter/382  "<Const_BrakeDiscFactor_RR[m3]>"
  ManifoldValve/1 -> SignalFilter/383  "<p_In_MainfoldValve[bar]>"
  ManifoldValve/2 -> SignalFilter/384  "<p_Out_MainfoldValve[bar]>"
  ManifoldValve/3 -> SignalFilter/385  "<T_In_MainfoldValve[degC]>"
  ManifoldValve/4 -> SignalFilter/386  "<m_dot_ManifoldValve[Kg|s]>"
  ManifoldValve/5 -> SignalFilter/387  "<m_dot_Out_ManifoldValve[Kg|s]>"
  ManifoldValve/6 -> SignalFilter/388  "<m_dot_In_ManifoldValve[Kg|s]>"
  VacuumChamber/1 -> SignalFilter/389  "<m_dot_In_1_VacuumChamber[kg|s]>"
  VacuumChamber/2 -> SignalFilter/390  "<m_dot_In_2_VacuumChamber[kg|s]>"
  VacuumChamber/3 -> SignalFilter/391  "<m_dot_Out_2_VacuumChamber[kg|s]>"
  VacuumChamber/4 -> SignalFilter/392  "<T_VacuumChamber[degC]>"
  VacuumChamber/5 -> SignalFilter/393  "<p_VacuumChamber[bar]>"
  VacuumChamber/6 -> SignalFilter/394  "<V_VacuumChamber[m3]>"
  BellValve/1 -> SignalFilter/395  "<ValveState[1ChamberCon|2AmbientCon|3CloseAll]>"
  BellValve/2 -> SignalFilter/396  "<p_In_BellValve[bar]>"
  BellValve/3 -> SignalFilter/397  "<p_Out_BellValve[bar]>"
  BellValve/4 -> SignalFilter/398  "<T_In_BellValve[degC]>"
  BellValve/5 -> SignalFilter/399  "<m_dot_BellValve[Kg|s]>"
  BellValve/6 -> SignalFilter/400  "<Ctrl_BellValve[0_1]>"
  RearChamber/1 -> SignalFilter/401  "<m_dot_In_RearChamber[kg|s]>"
  RearChamber/2 -> SignalFilter/402  "<m_dot_Out_RearChamber[kg|s]>"
  RearChamber/3 -> SignalFilter/403  "<T_RearChamber[degC]>"
  RearChamber/4 -> SignalFilter/404  "<p_RearChamber[bar]>"
  RearChamber/5 -> SignalFilter/405  "<V_RearChamber[m3]>"
  PushRod/1 -> SignalFilter/406  "<F_Pedal[N]>"
  PushRod/2 -> SignalFilter/407  "<F_Spring[N]>"
  PushRod/3 -> SignalFilter/408  "<F_RearChamber[N]>"
  PushRod/4 -> SignalFilter/409  "<F_VacuumChamber[N]>"
  PushRod/5 -> SignalFilter/410  "<F_PushRod[N]>"
  PushRod/6 -> SignalFilter/411  "<x[m]>"
  PushRod/7 -> SignalFilter/412  "<V_delta[m3]>"
  PushRod/8 -> SignalFilter/413  "<A_Diaphragm[m2]>"
  OutputPoint/1 -> SignalFilter/414  "<F_OutputPoint[N]>"
  OutputPoint/2 -> SignalFilter/415  "<p_OutputPoint[bar]>"
  OutputPoint/3 -> SignalFilter/416  "<Pos_BrakePedal_OutputPoint[%]>"
  OutputPoint/4 -> SignalFilter/417  "<F_Max_Pedal[N]>"
  OutputPoint/5 -> SignalFilter/418  "<p_Max_Booster[bar]>"
  ControllerBellValve/1 -> SignalFilter/419  "<p_Setpoint[bar]>"
  ControllerBellValve/2 -> SignalFilter/420  "<p_MasterBrakeCyl[bar]>"
  ControllerBellValve/3 -> SignalFilter/421  "<p_delta[bar]>"
  ControllerBellValve/4 -> SignalFilter/422  "<ValveState[1ChamberCon|2AmbientCon]>"
  ControllerBellValve/5 -> SignalFilter/423  "<Ctrl_A_BellValve[0_1]>"
  ControllerBellValve/6 -> SignalFilter/424  "<F_Pedal[N]>"
  Manifold/1 -> SignalFilter/425  "<Pos_AccPedal[%]>"
  Manifold/2 -> SignalFilter/426  "<p_Manifold[bar]>"
  Position_Left/1 -> Reshape_427/1  "<Pos_FL_Wheel[x;y;z][m]>"
  Reshape_427/1 -> SignalFilter/427
  Position_Left/2 -> Reshape_428/1  "<Pos_FL_Wheel_dq1_Front[x;y;z][]>"
  Reshape_428/1 -> SignalFilter/428
  Position_Left/3 -> Reshape_429/1  "<Pos_FL_Wheel_dq2_Front[x;y;z][]>"
  Reshape_429/1 -> SignalFilter/429
  Position_Left/4 -> Reshape_430/1  "<Pos_FL_Wheel_dDispl_SteeringRod[x;y;z][]>"
  Reshape_430/1 -> SignalFilter/430
  Angle_FL_Wheel[Alpha;Beta;Gamma][deg]/1 -> SignalFilter/431  "<Angle_Alpha_FL_Wheel[deg]>"
  Angle_FL_Wheel[Alpha;Beta;Gamma][deg]/2 -> SignalFilter/432  "<Angle_Beta_FL_Wheel[deg]>"
  Angle_FL_Wheel[Alpha;Beta;Gamma][deg]/3 -> SignalFilter/433  "<Angle_Gamma_FL_Wheel[deg]>"
  Orientation_Left/2 -> Reshape_434/1  "<w_Rel_FL_Wheel_dq1_Front_dt[x;y;z][]>"
  Reshape_434/1 -> SignalFilter/434
  Orientation_Left/3 -> Reshape_435/1  "<w_Rel_FL_Wheel_dq2_Front_dt[x;y;z][]>"
  Reshape_435/1 -> SignalFilter/435
  Orientation_Left/4 -> Reshape_436/1  "<w_Rel_FL_Wheel_dDispl_SteeringRod_dt[x;y;z][rad|m]>"
  Reshape_436/1 -> SignalFilter/436
  Orientation_Left/5 -> Reshape_437/1  "<UnitVec_y_Wheel_FL_CoorSys_V[x;y;z]>"
  Reshape_437/1 -> SignalFilter/437
  Spring_Left/1 -> SignalFilter/438  "<Displ_Spring_FL[m]>"
  Spring_Left/2 -> SignalFilter/439  "<Displ_Spring_FL_dq1_Front[]>"
  Spring_Left/3 -> SignalFilter/440  "<Displ_Spring_FL_dq2_Front[]>"
  Damper_Left/1 -> SignalFilter/441  "<Displ_Damper_FL_dt[m|s]>"
  Damper_Left/2 -> SignalFilter/442  "<Displ_Damper_FL_dq1_Front[]>"
  Damper_Left/3 -> SignalFilter/443  "<Displ_Damper_FL_dq2_Front[]>"
  Damper_Left/4 -> SignalFilter/444  "<Displ_Damper_FL[m]>"
  Position_Right/1 -> Reshape_445/1  "<Pos_FR_Wheel[x;y;z][m]>"
  Reshape_445/1 -> SignalFilter/445
  Position_Right/2 -> Reshape_446/1  "<Pos_FR_Wheel_dq1_Front[x;y;z][]>"
  Reshape_446/1 -> SignalFilter/446
  Position_Right/3 -> Reshape_447/1  "<Pos_FR_Wheel_dq2_Front[x;y;z][]>"
  Reshape_447/1 -> SignalFilter/447
  Position_Right/4 -> Reshape_448/1  "<Pos_FR_Wheel_dDispl_SteeringRod[x;y;z][]>"
  Reshape_448/1 -> SignalFilter/448
  Angle_FR_Wheel[Alpha;Beta;Gamma][deg]/1 -> SignalFilter/449  "<Angle_Alpha_FR_Wheel[deg]>"
  Angle_FR_Wheel[Alpha;Beta;Gamma][deg]/2 -> SignalFilter/450  "<Angle_Beta_FR_Wheel[deg]>"
  Angle_FR_Wheel[Alpha;Beta;Gamma][deg]/3 -> SignalFilter/451  "<Angle_Gamma_FR_Wheel[deg]>"
  Orientation_Right/2 -> Reshape_452/1  "<w_Rel_FR_Wheel_dq1_Front[x;y;z][]>"
  Reshape_452/1 -> SignalFilter/452
  Orientation_Right/3 -> Reshape_453/1  "<w_Rel_FR_Wheel_dq2_Front[x;y;z][]>"
  Reshape_453/1 -> SignalFilter/453
  Orientation_Right/4 -> Reshape_454/1  "<w_Rel_FR_Wheel_dDispl_SteeringRod_dt[x;y;z][rad|m]>"
  Reshape_454/1 -> SignalFilter/454
  Orientation_Right/5 -> Reshape_455/1  "<UnitVec_y_Wheel_FR_CoorSys_V[x;y;z]>"
  Reshape_455/1 -> SignalFilter/455
  Spring_Right/1 -> SignalFilter/456  "<Displ_Spring_FR[m]>"
  Spring_Right/2 -> SignalFilter/457  "<Displ_Spring_FR_dq1_Front[]>"
  Spring_Right/3 -> SignalFilter/458  "<Displ_Spring_FR_dq2_Front[]>"
  Damper_Right/1 -> SignalFilter/459  "<Displ_Damper_FR_dt[m|s]>"
  Damper_Right/2 -> SignalFilter/460  "<Displ_Damper_FR_dq1_Front[]>"
  Damper_Right/3 -> SignalFilter/461  "<Displ_Damper_FR_dq2_Front[]>"
  Damper_Right/4 -> SignalFilter/462  "<Displ_Damper_FR[m]>"
  Stabilizer/1 -> SignalFilter/463  "<Displ_Stabilizer[m]>"
  Stabilizer/2 -> SignalFilter/464  "<Displ_Stabilizer_FL[m]>"
  Stabilizer/3 -> SignalFilter/465  "<Displ_Stabilizer_FR[m]>"
  Stabilizer/4 -> SignalFilter/466  "<Displ_Stabilizer_dq1_Front[]>"
  Stabilizer/5 -> SignalFilter/467  "<Displ_Stabilizer_dq2_Front[]>"
  SuspensionKinematicsFront/4 -> SignalFilter/468  "<SusKinFrontModel[]>"
  SuspensionComplianceFront/1 -> Reshape_469/1  "<Angle_Comp_FR_Wheel_dt[x;y;z][m]>"
  Reshape_469/1 -> SignalFilter/469
  SuspensionComplianceFront/2 -> Reshape_470/1  "<Angle_Comp_FL_Wheel_dt[x;y;z][m]>"
  Reshape_470/1 -> SignalFilter/470
  SuspensionComplianceFront/3 -> Reshape_471/1  "<Angle_Comp_FR_Wheel[x;y;z][rad]>"
  Reshape_471/1 -> SignalFilter/471
  SuspensionComplianceFront/4 -> Reshape_472/1  "<Angle_Comp_FL_Wheel[x;y;z][rad]>"
  Reshape_472/1 -> SignalFilter/472
  SuspensionComplianceFront/5 -> Reshape_473/1  "<Displ_Comp_FR_Wheel_dt[x;y;z][m]>"
  Reshape_473/1 -> SignalFilter/473
  SuspensionComplianceFront/6 -> Reshape_474/1  "<Displ_Comp_FL_Wheel_dt[x;y;z][m]>"
  Reshape_474/1 -> SignalFilter/474
  SuspensionComplianceFront/7 -> Reshape_475/1  "<Displ_Comp_FR_Wheel[x;y;z][m]>"
  Reshape_475/1 -> SignalFilter/475
  SuspensionComplianceFront/8 -> Reshape_476/1  "<Displ_Comp_FL_Wheel[x;y;z][m]>"
  Reshape_476/1 -> SignalFilter/476
  ComplianceLongForce/1 -> SignalFilter/477  "<Displ_x_Wheel_F_x_Left[mm]>"
  ComplianceLongForce/2 -> SignalFilter/478  "<Displ_x_Wheel_F_x_Right[mm]>"
  ComplianceLongForce/3 -> SignalFilter/479  "<Displ_y_Wheel_F_x_Left[mm]>"
  ComplianceLongForce/4 -> SignalFilter/480  "<Displ_y_Wheel_F_x_Right[mm]>"
  ComplianceLongForce/5 -> SignalFilter/481  "<Angle_Alpha_Wheel_F_x_Left[deg]>"
  ComplianceLongForce/6 -> SignalFilter/482  "<Angle_Alpha_Wheel_F_x_Right[deg]>"
  ComplianceLongForce/7 -> SignalFilter/483  "<Angle_Gamma_Wheel_F_x_Left[deg]>"
  ComplianceLongForce/8 -> SignalFilter/484  "<Angle_Gamma_Wheel_F_x_Right[deg]>"
  ComplianceLatForce/1 -> SignalFilter/485  "<Displ_x_Wheel_F_y_Left[mm]>"
  ComplianceLatForce/2 -> SignalFilter/486  "<Displ_x_Wheel_F_y_Right[mm]>"
  ComplianceLatForce/3 -> SignalFilter/487  "<Displ_y_Wheel_F_y_Left[mm]>"
  ComplianceLatForce/4 -> SignalFilter/488  "<Displ_y_Wheel_F_y_Right[mm]>"
  ComplianceLatForce/5 -> SignalFilter/489  "<Angle_Alpha_Wheel_F_y_Left[deg]>"
  ComplianceLatForce/6 -> SignalFilter/490  "<Angle_Alpha_Wheel_F_y_Right[deg]>"
  ComplianceLatForce/7 -> SignalFilter/491  "<Angle_Gamma_Wheel_F_y_Left[deg]>"
  ComplianceLatForce/8 -> SignalFilter/492  "<Angle_Gamma_Wheel_F_y_Right[deg]>"
  ComplianceAligningTorque/1 -> SignalFilter/493  "<Displ_x_Wheel_Trq_z_Left[mm]>"
  ComplianceAligningTorque/2 -> SignalFilter/494  "<Displ_x_Wheel_Trq_z_Right[mm]>"
  ComplianceAligningTorque/3 -> SignalFilter/495  "<Displ_y_Wheel_Trq_z_Left[mm]>"
  ComplianceAligningTorque/4 -> SignalFilter/496  "<Displ_y_Wheel_Trq_z_Right[mm]>"
  ComplianceAligningTorque/5 -> SignalFilter/497  "<Angle_Alpha_Wheel_Trq_z_Left[deg]>"
  ComplianceAligningTorque/6 -> SignalFilter/498  "<Angle_Alpha_Wheel_Trq_z_Right[deg]>"
  ComplianceAligningTorque/7 -> SignalFilter/499  "<Angle_Gamma_Wheel_Trq_z_Left[deg]>"
  ComplianceAligningTorque/8 -> SignalFilter/500  "<Angle_Gamma_Wheel_Trq_z_Right[deg]>"
  ComplianceLongTorque/1 -> SignalFilter/501  "<Displ_x_Wheel_Trq_x_Left[mm]>"
  ComplianceLongTorque/2 -> SignalFilter/502  "<Displ_x_Wheel_Trq_x_Right[mm]>"
  ComplianceLongTorque/3 -> SignalFilter/503  "<Displ_y_Wheel_Trq_x_Left[mm]>"
  ComplianceLongTorque/4 -> SignalFilter/504  "<Displ_y_Wheel_Trq_x_Right[mm]>"
  ComplianceLongTorque/5 -> SignalFilter/505  "<Angle_Alpha_Wheel_Trq_x_Left[deg]>"
  ComplianceLongTorque/6 -> SignalFilter/506  "<Angle_Alpha_Wheel_Trq_x_Right[deg]>"
  ComplianceLongTorque/7 -> SignalFilter/507  "<Angle_Gamma_Wheel_Trq_x_Left[deg]>"
  ComplianceLongTorque/8 -> SignalFilter/508  "<Angle_Gamma_Wheel_Trq_x_Right[deg]>"
  SuspensionForcesFront/1 -> SignalFilter/509  "<F_FL_Spring[N]>"
  SuspensionForcesFront/2 -> SignalFilter/510  "<F_FL_Spring_dDispl_FL_Spring[N|m]>"
  SuspensionForcesFront/3 -> SignalFilter/511  "<F_FL_Damper[N]>"
  SuspensionForcesFront/4 -> SignalFilter/512  "<F_FL_Damper_dDispl_FL_Damper_dt[N|(m|s)]>"
  SuspensionForcesFront/5 -> SignalFilter/513  "<F_Stabilizer[N]>"
  SuspensionForcesFront/6 -> SignalFilter/514  "<F_Stabilizer_dDispl_Stabilizer[N|m]>"
  SuspensionForcesFront/7 -> SignalFilter/515  "<F_FR_Spring[N]>"
  SuspensionForcesFront/8 -> SignalFilter/516  "<F_FR_Spring_dDispl_FR_Spring[N|m]>"
  SuspensionForcesFront/9 -> SignalFilter/517  "<F_FR_Damper[N]>"
  SuspensionForcesFront/10 -> SignalFilter/518  "<F_FR_Damper_dDispl_FR_Damper_dt[N|(m|s)]>"
  Pos_Wheel[FL;FR][x;y;z][m]/1 -> Reshape_519/1  "<Pos_FL_Wheel[x;y;z][m]>"
  Reshape_519/1 -> SignalFilter/519
  Pos_Wheel[FL;FR][x;y;z][m]/2 -> Reshape_520/1  "<Pos_FR_Wheel[x;y;z][m]>"
  Reshape_520/1 -> SignalFilter/520
  UnitVec_y_Wheel_CoorSys_V[FL;FR][x;y;z]/1 -> Reshape_521/1  "<UnitVec_y_FL_Wheel_CoorSys_V[x;y;z]>"
  Reshape_521/1 -> SignalFilter/521
  UnitVec_y_Wheel_CoorSys_V[FL;FR][x;y;z]/2 -> Reshape_522/1  "<UnitVec_y_FR_Wheel_CoorSys_V[x;y;z]>"
  Reshape_522/1 -> SignalFilter/522
  Angle_FL_Wheel[Toe;Camber][deg]/1 -> SignalFilter/523  "<Angle_Toe_FL_Wheel_CoorSys_V[deg]>"
  Angle_FL_Wheel[Toe;Camber][deg]/2 -> SignalFilter/524  "<Angle_Camber_FL_Wheel_CoorSys_V[deg]>"
  Angle_FR_Wheel[Toe;Camber][deg]/1 -> SignalFilter/525  "<Angle_Toe_FR_Wheel_CoorSys_V[deg]>"
  Angle_FR_Wheel[Toe;Camber][deg]/2 -> SignalFilter/526  "<Angle_Camber_FR_Wheel_CoorSys_V[deg]>"
  Position_Left1/1 -> Reshape_527/1  "<Pos_RL_Wheel[x;y;z][m]>"
  Reshape_527/1 -> SignalFilter/527
  Position_Left1/2 -> Reshape_528/1  "<Pos_RL_Wheel_dq1_Rear[x;y;z][]>"
  Reshape_528/1 -> SignalFilter/528
  Position_Left1/3 -> Reshape_529/1  "<Pos_RL_Wheel_dq2_Rear[x;y;z][]>"
  Reshape_529/1 -> SignalFilter/529
  Position_Left1/4 -> Reshape_530/1  "<Pos_RL_Wheel_dDispl_SteeringRod[x;y;z][]>"
  Reshape_530/1 -> SignalFilter/530
  Angle_RL_Wheel[Alpha;Beta;Gamma][deg]/1 -> SignalFilter/531  "<Angle_Alpha_RL_Wheel[deg]>"
  Angle_RL_Wheel[Alpha;Beta;Gamma][deg]/2 -> SignalFilter/532  "<Angle_Beta_RL_Wheel[deg]>"
  Angle_RL_Wheel[Alpha;Beta;Gamma][deg]/3 -> SignalFilter/533  "<Angle_Gamma_RL_Wheel[deg]>"
  Orientation_Left1/2 -> Reshape_534/1  "<w_Rel_RL_Wheel_dq1_Rear_dt[x;y;z][]>"
  Reshape_534/1 -> SignalFilter/534
  Orientation_Left1/3 -> Reshape_535/1  "<w_Rel_RL_Wheel_dq2_Rear_dt[x;y;z][]>"
  Reshape_535/1 -> SignalFilter/535
  Orientation_Left1/4 -> Reshape_536/1  "<w_Rel_RL_Wheel_dDispl_SteeringRod_dt[x;y;z][rad|m]>"
  Reshape_536/1 -> SignalFilter/536
  Orientation_Left1/5 -> Reshape_537/1  "<UnitVec_y_Wheel_RL_CoorSys_V[x;y;z]>"
  Reshape_537/1 -> SignalFilter/537
  Spring_Left1/1 -> SignalFilter/538  "<Displ_Spring_RL[m]>"
  Spring_Left1/2 -> SignalFilter/539  "<Displ_Spring_RL_dq1_Rear[]>"
  Spring_Left1/3 -> SignalFilter/540  "<Displ_Spring_RL_dq2_Rear[]>"
  Damper_Left1/1 -> SignalFilter/541  "<Displ_Damper_RL_dt[m|s]>"
  Damper_Left1/2 -> SignalFilter/542  "<Displ_Damper_RL_dq1_Rear>"
  Damper_Left1/3 -> SignalFilter/543  "<Displ_Damper_RL_dq2_Rear>"
  Damper_Left1/4 -> SignalFilter/544  "<Displ_Damper_RL[m]>"
  Position_Right1/1 -> Reshape_545/1  "<Pos_RR_Wheel[x;y;z][m]>"
  Reshape_545/1 -> SignalFilter/545
  Position_Right1/2 -> Reshape_546/1  "<Pos_RR_Wheel_dq1_Rear[x;y;z][]>"
  Reshape_546/1 -> SignalFilter/546
  Position_Right1/3 -> Reshape_547/1  "<Pos_RR_Wheel_dq2_Rear[x;y;z][]>"
  Reshape_547/1 -> SignalFilter/547
  Position_Right1/4 -> Reshape_548/1  "<Pos_RR_Wheel_dDispl_SteeringRod[x;y;z][]>"
  Reshape_548/1 -> SignalFilter/548
  Angle_RR_Wheel[Alpha;Beta;Gamma][deg]/1 -> SignalFilter/549  "<Angle_Alpha_RR_Wheel[deg]>"
  Angle_RR_Wheel[Alpha;Beta;Gamma][deg]/2 -> SignalFilter/550  "<Angle_Beta_RR_Wheel[deg]>"
  Angle_RR_Wheel[Alpha;Beta;Gamma][deg]/3 -> SignalFilter/551  "<Angle_Gamma_RR_Wheel[deg]>"
  Orientation_Right1/2 -> Reshape_552/1  "<w_Rel_RR_Wheel_dq1_Rear[x;y;z][]>"
  Reshape_552/1 -> SignalFilter/552
  Orientation_Right1/3 -> Reshape_553/1  "<w_Rel_RR_Wheel_dq2_Rear[x;y;z][]>"
  Reshape_553/1 -> SignalFilter/553
  Orientation_Right1/4 -> Reshape_554/1  "<w_Rel_RR_Wheel_dDispl_SteeringRod_dt[x;y;z][rad|m]>"
  Reshape_554/1 -> SignalFilter/554
  Orientation_Right1/5 -> Reshape_555/1  "<UnitVec_y_Wheel_RR_CoorSys_V[x;y;z]>"
  Reshape_555/1 -> SignalFilter/555
  Spring_Right1/1 -> SignalFilter/556  "<Displ_Spring_RR[m]>"
  Spring_Right1/2 -> SignalFilter/557  "<Displ_Spring_RR_dq1_Rear[]>"
  Spring_Right1/3 -> SignalFilter/558  "<Displ_Spring_RR_dq2_Rear[]>"
  Damper_Right1/1 -> SignalFilter/559  "<Displ_Damper_RR_dt[m|s]>"
  Damper_Right1/2 -> SignalFilter/560  "<Displ_Damper_RR_dq1_Rear[]>"
  Damper_Right1/3 -> SignalFilter/561  "<Displ_Damper_RR_dq2_Rear[]>"
  Damper_Right1/4 -> SignalFilter/562  "<Displ_Damper_RR[m]>"
  Stabilizer1/1 -> SignalFilter/563  "<Displ_Stabilizer[m]>"
  Stabilizer1/2 -> SignalFilter/564  "<Displ_Stabilizer_RL[m]>"
  Stabilizer1/3 -> SignalFilter/565  "<Displ_Stabilizer_RR[m]>"
  Stabilizer1/4 -> SignalFilter/566  "<Displ_Stabilizer_dq1_Rear[]>"
  Stabilizer1/5 -> SignalFilter/567  "<Displ_Stabilizer_dq2_Rear[]>"
  SuspensionKinematicsRear/4 -> SignalFilter/568  "<SusKinRearModel[]>"
  SuspensionComplianceRear/1 -> Reshape_569/1  "<Angle_Comp_RR_Wheel_dt[x;y;z][m]>"
  Reshape_569/1 -> SignalFilter/569
  SuspensionComplianceRear/2 -> Reshape_570/1  "<Angle_Comp_RL_Wheel_dt[x;y;z][m]>"
  Reshape_570/1 -> SignalFilter/570
  SuspensionComplianceRear/3 -> Reshape_571/1  "<Angle_Comp_RR_Wheel[x;y;z][rad]>"
  Reshape_571/1 -> SignalFilter/571
  SuspensionComplianceRear/4 -> Reshape_572/1  "<Angle_Comp_RL_Wheel[x;y;z][rad]>"
  Reshape_572/1 -> SignalFilter/572
  SuspensionComplianceRear/5 -> Reshape_573/1  "<Displ_Comp_RR_Wheel_dt[x;y;z][m]>"
  Reshape_573/1 -> SignalFilter/573
  SuspensionComplianceRear/6 -> Reshape_574/1  "<Displ_Comp_RL_Wheel_dt[x;y;z][m]>"
  Reshape_574/1 -> SignalFilter/574
  SuspensionComplianceRear/7 -> Reshape_575/1  "<Displ_Comp_RR_Wheel[x;y;z][m]>"
  Reshape_575/1 -> SignalFilter/575
  SuspensionComplianceRear/8 -> Reshape_576/1  "<Displ_Comp_RL_Wheel[x;y;z][m]>"
  Reshape_576/1 -> SignalFilter/576
  ComplianceLongForce1/1 -> SignalFilter/577  "<Displ_x_Wheel_F_x_Left[mm]>"
  ComplianceLongForce1/2 -> SignalFilter/578  "<Displ_x_Wheel_F_x_Right[mm]>"
  ComplianceLongForce1/3 -> SignalFilter/579  "<Displ_y_Wheel_F_x_Left[mm]>"
  ComplianceLongForce1/4 -> SignalFilter/580  "<Displ_y_Wheel_F_x_Right[mm]>"
  ComplianceLongForce1/5 -> SignalFilter/581  "<Angle_Alpha_Wheel_F_x_Left[deg]>"
  ComplianceLongForce1/6 -> SignalFilter/582  "<Angle_Alpha_Wheel_F_x_Right[deg]>"
  ComplianceLongForce1/7 -> SignalFilter/583  "<Angle_Gamma_Wheel_F_x_Left[deg]>"
  ComplianceLongForce1/8 -> SignalFilter/584  "<Angle_Gamma_Wheel_F_x_Right[deg]>"
  ComplianceLatForce1/1 -> SignalFilter/585  "<Displ_x_Wheel_F_y_Left[mm]>"
  ComplianceLatForce1/2 -> SignalFilter/586  "<Displ_x_Wheel_F_y_Right[mm]>"
  ComplianceLatForce1/3 -> SignalFilter/587  "<Displ_y_Wheel_F_y_Left[mm]>"
  ComplianceLatForce1/4 -> SignalFilter/588  "<Displ_y_Wheel_F_y_Right[mm]>"
  ComplianceLatForce1/5 -> SignalFilter/589  "<Angle_Alpha_Wheel_F_y_Left[deg]>"
  ComplianceLatForce1/6 -> SignalFilter/590  "<Angle_Alpha_Wheel_F_y_Right[deg]>"
  ComplianceLatForce1/7 -> SignalFilter/591  "<Angle_Gamma_Wheel_F_y_Left[deg]>"
  ComplianceLatForce1/8 -> SignalFilter/592  "<Angle_Gamma_Wheel_F_y_Right[deg]>"
  ComplianceAligningTorque1/1 -> SignalFilter/593  "<Displ_x_Wheel_Trq_z_Left[mm]>"
  ComplianceAligningTorque1/2 -> SignalFilter/594  "<Displ_x_Wheel_Trq_z_Right[mm]>"
  ComplianceAligningTorque1/3 -> SignalFilter/595  "<Displ_y_Wheel_Trq_z_Left[mm]>"
  ComplianceAligningTorque1/4 -> SignalFilter/596  "<Displ_y_Wheel_Trq_z_Right[mm]>"
  ComplianceAligningTorque1/5 -> SignalFilter/597  "<Angle_Alpha_Wheel_Trq_z_Left[deg]>"
  ComplianceAligningTorque1/6 -> SignalFilter/598  "<Angle_Alpha_Wheel_Trq_z_Right[deg]>"
  ComplianceAligningTorque1/7 -> SignalFilter/599  "<Angle_Gamma_Wheel_Trq_z_Left[deg]>"
  ComplianceAligningTorque1/8 -> SignalFilter/600  "<Angle_Gamma_Wheel_Trq_z_Right[deg]>"
  ComplianceLongTorque1/1 -> SignalFilter/601  "<Displ_x_Wheel_Trq_x_Left[mm]>"
  ComplianceLongTorque1/2 -> SignalFilter/602  "<Displ_x_Wheel_Trq_x_Right[mm]>"
  ComplianceLongTorque1/3 -> SignalFilter/603  "<Displ_y_Wheel_Trq_x_Left[mm]>"
  ComplianceLongTorque1/4 -> SignalFilter/604  "<Displ_y_Wheel_Trq_x_Right[mm]>"
  ComplianceLongTorque1/5 -> SignalFilter/605  "<Angle_Alpha_Wheel_Trq_x_Left[deg]>"
  ComplianceLongTorque1/6 -> SignalFilter/606  "<Angle_Alpha_Wheel_Trq_x_Right[deg]>"
  ComplianceLongTorque1/7 -> SignalFilter/607  "<Angle_Gamma_Wheel_Trq_x_Left[deg]>"
  ComplianceLongTorque1/8 -> SignalFilter/608  "<Angle_Gamma_Wheel_Trq_x_Right[deg]>"
  SuspensionForcesRear/1 -> SignalFilter/609  "<F_RL_Spring[N]>"
  SuspensionForcesRear/2 -> SignalFilter/610  "<F_RL_Spring_dDispl_RL_Spring[N|m]>"
  SuspensionForcesRear/3 -> SignalFilter/611  "<F_RL_Damper[N]>"
  SuspensionForcesRear/4 -> SignalFilter/612  "<F_RL_Damper_dDispl_RL_Damper_dt[N|(m|s)]>"
  SuspensionForcesRear/5 -> SignalFilter/613  "<F_Stabilizer[N]>"
  SuspensionForcesRear/6 -> SignalFilter/614  "<F_Stabilizer_dDispl_Stabilizer[N|m]>"
  SuspensionForcesRear/7 -> SignalFilter/615  "<F_RR_Spring[N]>"
  SuspensionForcesRear/8 -> SignalFilter/616  "<F_RR_Spring_dDispl_RR_Spring[N|m]>"
  SuspensionForcesRear/9 -> SignalFilter/617  "<F_RR_Damper[N]>"
  SuspensionForcesRear/10 -> SignalFilter/618  "<F_RR_Damper_dDispl_RR_Damper_dt[N|(m|s)]>"
  Pos_Wheel[RL;RR][x;y;z][m]/1 -> Reshape_619/1  "<Pos_RL_Wheel[x;y;z][m]>"
  Reshape_619/1 -> SignalFilter/619
  Pos_Wheel[RL;RR][x;y;z][m]/2 -> Reshape_620/1  "<Pos_RR_Wheel[x;y;z][m]>"
  Reshape_620/1 -> SignalFilter/620
  UnitVec_y_Wheel_CoorSys_V[RL;RR][x;y;z]/1 -> Reshape_621/1  "<UnitVec_y_RL_Wheel_CoorSys_V[x;y;z]>"
  Reshape_621/1 -> SignalFilter/621
  UnitVec_y_Wheel_CoorSys_V[RL;RR][x;y;z]/2 -> Reshape_622/1  "<UnitVec_y_RR_Wheel_CoorSys_V[x;y;z]>"
  Reshape_622/1 -> SignalFilter/622
  Angle_RL_Wheel[Toe;Camber][deg]/1 -> SignalFilter/623  "<Angle_Toe_RL_Wheel_CoorSys_V[deg]>"
